simulink model "DYN_02x"  (R2021a)
(part 48 of 53)

 (de2*(0.5*(sin(e6)*(sin(e2 + e3)*sin(e5) - 1.0*cos(e2 + e3)*cos(e4)*cos(e5)) - 1.0*cos(e2 + e3)*cos(e6)*sin(e4))*(I6xy*(cos(e4)*cos(e6) - 1.0*cos(e5)*sin(e4)*sin(e6)) - 1.0*I6yy*(cos(e4)*sin(e6) + cos(e5)*cos(e6)*sin(e4))) + 0.5*(cos(e4)*sin(e6) + cos(e5)*cos(e6)*sin(e4))*(I6zy*(sin(e2 + e3)*cos(e5) + cos(e2 + e3)*cos(e4)*sin(e5)) + I6xy*(cos(e6)*(sin(e2 + e3)*sin(e5) - 1.0*cos(e2 + e3)*cos(e4)*cos(e5)) + cos(e2 + e3)*sin(e4)*sin(e6)) - 1.0*I6yy*(sin(e6)*(sin(e2 + e3)*sin(e5) - 1.0*cos(e2 + e3)*cos(e4)*cos(e5)) - 1.0*cos(e2 + e3)*cos(e6)*sin(e4))) + 0.5*(cos(e6)*(sin(e2 + e3)*sin(e5) - 1.0*cos(e2 + e3)*cos(e4)*cos(e5)) + cos(e2 + e3)*sin(e4)*sin(e6))*(I6yy*(cos(e4)*cos(e6) - 1.0*cos(e5)*sin(e4)*sin(e6)) + I6xy*(cos(e4)*sin(e6) + cos(e5)*cos(e6)*sin(e4)) - 1.0*I6zy*sin(e4)*sin(e5)) - 0.5*(cos(e4)*cos(e6) - 1.0*cos(e5)*sin(e4)*sin(e6))*(I6zx*(sin(e2 + e3)*cos(e5) + cos(e2 + e3)*cos(e4)*sin(e5)) + I6xx*(cos(e6)*(sin(e2 + e3)*sin(e5) - 1.0*cos(e2 + e3)*cos(e4)*cos(e5)) + cos(e2 + e3)*sin(e4)*sin(e6)) - 1.0*I6yx*(sin(e6)*(sin(e2 + e3)*sin(e5) - 1.0*cos(e2 + e3)*cos(e4)*cos(e5)) - 1.0*cos(e2 + e3)*cos(e6)*sin(e4))) + 0.5*(sin(e6)*(sin(e2 + e3)*sin(e5) - 1.0*cos(e2 + e3)*cos(e4)*cos(e5)) - 1.0*cos(e2 + e3)*cos(e6)*sin(e4))*(I6yx*(cos(e4)*cos(e6) - 1.0*cos(e5)*sin(e4)*sin(e6)) + I6xx*(cos(e4)*sin(e6) + cos(e5)*cos(e6)*sin(e4)) - 1.0*I6zx*sin(e4)*sin(e5)) - 0.5*(I6xz*(cos(e4)*cos(e6) - 1.0*cos(e5)*sin(e4)*sin(e6)) - 1.0*I6yz*(cos(e4)*sin(e6) + cos(e5)*cos(e6)*sin(e4)))*(sin(e2 + e3)*cos(e5) + cos(e2 + e3)*cos(e4)*sin(e5)) + 0.5*(I6yx*(cos(e6)*(sin(e2 + e3)*sin(e5) - 1.0*cos(e2 + e3)*cos(e4)*cos(e5)) + cos(e2 + e3)*sin(e4)*sin(e6)) + I6xx*(sin(e6)*(sin(e2 + e3)*sin(e5) - 1.0*cos(e2 + e3)*cos(e4)*cos(e5)) - 1.0*cos(e2 + e3)*cos(e6)*sin(e4)))*(cos(e4)*sin(e6) + cos(e5)*cos(e6)*sin(e4)) + 0.5*(I6yy*(cos(e6)*(sin(e2 + e3)*sin(e5) - 1.0*cos(e2 + e3)*cos(e4)*cos(e5)) + cos(e2 + e3)*sin(e4)*sin(e6)) + I6xy*(sin(e6)*(sin(e2 + e3)*sin(e5) - 1.0*cos(e2 + e3)*cos(e4)*cos(e5)) - 1.0*cos(e2 + e3)*cos(e6)*sin(e4)))*(cos(e4)*cos(e6) - 1.0*cos(e5)*sin(e4)*sin(e6)) - 0.5*(cos(e6)*(sin(e2 + e3)*sin(e5) - 1.0*cos(e2 + e3)*cos(e4)*cos(e5)) + cos(e2 + e3)*sin(e4)*sin(e6))*(I6xx*(cos(e4)*cos(e6) - 1.0*cos(e5)*sin(e4)*sin(e6)) - 1.0*I6yx*(cos(e4)*sin(e6) + cos(e5)*cos(e6)*sin(e4))) - 0.5*sin(e4)*sin(e5)*(I6yz*(cos(e6)*(sin(e2 + e3)*sin(e5) - 1.0*cos(e2 + e3)*cos(e4)*cos(e5)) + cos(e2 + e3)*sin(e4)*sin(e6)) + I6xz*(sin(e6)*(sin(e2 + e3)*sin(e5) - 1.0*cos(e2 + e3)*cos(e4)*cos(e5)) - 1.0*cos(e2 + e3)*cos(e6)*sin(e4))) + m6*((cos(e6)*(sin(e5)*(cos(e2)*sin(e3) + cos(e3)*sin(e2)) + cos(e4)*cos(e5)*(sin(e2)*sin(e3) - 1.0*cos(e2)*cos(e3))) - 1.0*sin(e4)*sin(e6)*(sin(e2)*sin(e3) - 1.0*cos(e2)*cos(e3)))*(z6*(cos(e4)*cos(e6) - 1.0*cos(e5)*sin(e4)*sin(e6)) - 1.0*cos(e6)*(sin(e5)*(a3 + a2*cos(e3)) - 1.0*cos(e4)*cos(e5)*(d4 - 1.0*a2*sin(e3))) + y6*sin(e4)*sin(e5) - 1.0*sin(e4)*sin(e6)*(d4 - 1.0*a2*sin(e3))) - 1.0*(cos(e5)*(cos(e2)*sin(e3) + cos(e3)*sin(e2)) - 1.0*cos(e4)*sin(e5)*(sin(e2)*sin(e3) - 1.0*cos(e2)*cos(e3)))*(x6*(cos(e4)*cos(e6) - 1.0*cos(e5)*sin(e4)*sin(e6)) - 1.0*y6*(cos(e4)*sin(e6) + cos(e5)*cos(e6)*sin(e4)) + cos(e5)*(a3 + a2*cos(e3)) + cos(e4)*sin(e5)*(d4 - 1.0*a2*sin(e3))) + (sin(e6)*(sin(e5)*(cos(e2)*sin(e3) + cos(e3)*sin(e2)) + cos(e4)*cos(e5)*(sin(e2)*sin(e3) - 1.0*cos(e2)*cos(e3))) + cos(e6)*sin(e4)*(sin(e2)*sin(e3) - 1.0*cos(e2)*cos(e3)))*(z6*(cos(e4)*sin(e6) + cos(e5)*cos(e6)*sin(e4)) - 1.0*sin(e6)*(sin(e5)*(a3 + a2*cos(e3)) - 1.0*cos(e4)*cos(e5)*(d4 - 1.0*a2*sin(e3))) + x6*sin(e4)*sin(e5) + cos(e6)*sin(e4)*(d4 - 1.0*a2*sin(e3))))*(1.0*(cos(e6)*(sin(e5)*(cos(e2)*sin(e3) + cos(e3)*sin(e2)) + cos(e4)*cos(e5)*(sin(e2)*sin(e3) - 1.0*cos(e2)*cos(e3))) - 1.0*sin(e4)*sin(e6)*(sin(e2)*sin(e3) - 1.0*cos(e2)*cos(e3)))*(x6*(sin(e2 + e3)*cos(e5) + cos(e2 + e3)*cos(e4)*sin(e5)) - 1.0*z6*(cos(e6)*(sin(e2 + e3)*sin(e5) - 1.0*cos(e2 + e3)*cos(e4)*cos(e5)) + cos(e2 + e3)*sin(e4)*sin(e6)) + cos(e4)*cos(e6)*(a1 + d4*cos(e2 + e3) + a3*sin(e2 + e3) + a2*sin(e2)) - 1.0*cos(e5)*sin(e4)*sin(e6)*(a1 + d4*cos(e2 + e3) + a3*sin(e2 + e3) + a2*sin(e2))) - (sin(e6)*(sin(e5)*(cos(e2)*sin(e3) + cos(e3)*sin(e2)) + cos(e4)*cos(e5)*(sin(e2)*sin(e3) - 1.0*cos(e2)*cos(e3))) + cos(e6)*sin(e4)*(sin(e2)*sin(e3) - 1.0*cos(e2)*cos(e3)))*(z6*(sin(e6)*(sin(e2 + e3)*sin(e5) - 1.0*cos(e2 + e3)*cos(e4)*cos(e5)) - 1.0*cos(e2 + e3)*cos(e6)*sin(e4)) + y6*(sin(e2 + e3)*cos(e5) + cos(e2 + e3)*cos(e4)*sin(e5)) - 1.0*cos(e4)*sin(e6)*(a1 + d4*cos(e2 + e3) + a3*sin(e2 + e3) + a2*sin(e2)) - 1.0*cos(e5)*cos(e6)*sin(e4)*(a1 + d4*cos(e2 + e3) + a3*sin(e2 + e3) + a2*sin(e2))) - (sin(e6)*(sin(e5)*(cos(e2)*sin(e3) + cos(e3)*sin(e2)) + cos(e4)*cos(e5)*(sin(e2)*sin(e3) - 1.0*cos(e2)*cos(e3))) + cos(e6)*sin(e4)*(sin(e2)*sin(e3) - 1.0*cos(e2)*cos(e3)))*(cos(e4)*sin(e6)*(a1 + d4*cos(e2 + e3) + a3*sin(e2 + e3) + a2*sin(e2)) - 1.0*z6*(sin(e6)*(sin(e2 + e3)*sin(e5) - 1.0*cos(e2 + e3)*cos(e4)*cos(e5)) - 1.0*cos(e2 + e3)*cos(e6)*sin(e4)) + cos(e5)*cos(e6)*sin(e4)*(a1 + d4*cos(e2 + e3) + a3*sin(e2 + e3) + a2*sin(e2))) + 1.0*(cos(e6)*(sin(e5)*(cos(e2)*sin(e3) + cos(e3)*sin(e2)) + cos(e4)*cos(e5)*(sin(e2)*sin(e3) - 1.0*cos(e2)*cos(e3))) - 1.0*sin(e4)*sin(e6)*(sin(e2)*sin(e3) - 1.0*cos(e2)*cos(e3)))*(z6*(cos(e6)*(sin(e2 + e3)*sin(e5) - 1.0*cos(e2 + e3)*cos(e4)*cos(e5)) + cos(e2 + e3)*sin(e4)*sin(e6)) - 1.0*cos(e4)*cos(e6)*(a1 + d4*cos(e2 + e3) + a3*sin(e2 + e3) + a2*sin(e2)) + cos(e5)*sin(e4)*sin(e6)*(a1 + d4*cos(e2 + e3) + a3*sin(e2 + e3) + a2*sin(e2))) + (1.0*y6*(sin(e6)*(sin(e2 + e3)*sin(e5) - 1.0*cos(e2 + e3)*cos(e4)*cos(e5)) - 1.0*cos(e2 + e3)*cos(e6)*sin(e4)) - x6*(cos(e6)*(sin(e2 + e3)*sin(e5) - 1.0*cos(e2 + e3)*cos(e4)*cos(e5)) + cos(e2 + e3)*sin(e4)*sin(e6)))*(cos(e5)*(cos(e2)*sin(e3) + cos(e3)*sin(e2)) - 1.0*cos(e4)*sin(e5)*(sin(e2)*sin(e3) - 1.0*cos(e2)*cos(e3)))) - m6*((sin(e6)*(1.0*cos(e5)*(cos(e1)*sin(e4) - 1.0*cos(e4)*(cos(e2)*sin(e1)*sin(e3) + cos(e3)*sin(e1)*sin(e2))) - sin(e5)*(cos(e2)*cos(e3)*sin(e1) - 1.0*sin(e1)*sin(e2)*sin(e3))) - cos(e6)*(sin(e4)*(cos(e2)*sin(e1)*sin(e3) + cos(e3)*sin(e1)*sin(e2)) + cos(e1)*cos(e4)))*(x6*(sin(e2 + e3)*cos(e5) + cos(e2 + e3)*cos(e4)*sin(e5)) - 1.0*z6*(cos(e6)*(sin(e2 + e3)*sin(e5) - 1.0*cos(e2 + e3)*cos(e4)*cos(e5)) + cos(e2 + e3)*sin(e4)*sin(e6)) + cos(e4)*cos(e6)*(a1 + d4*cos(e2 + e3) + a3*sin(e2 + e3) + a2*sin(e2)) - 1.0*cos(e5)*sin(e4)*sin(e6)*(a1 + d4*cos(e2 + e3) + a3*sin(e2 + e3) + a2*sin(e2))) + 1.0*(sin(e5)*(cos(e1)*sin(e4) - 1.0*cos(e4)*(cos(e2)*sin(e1)*sin(e3) + cos(e3)*sin(e1)*sin(e2))) + cos(e5)*(cos(e2)*cos(e3)*sin(e1) - 1.0*sin(e1)*sin(e2)*sin(e3)))*(x6*(sin(e6)*(sin(e2 + e3)*sin(e5) - 1.0*cos(e2 + e3)*cos(e4)*cos(e5)) - 1.0*cos(e2 + e3)*cos(e6)*sin(e4)) + y6*(cos(e6)*(sin(e2 + e3)*sin(e5) - 1.0*cos(e2 + e3)*cos(e4)*cos(e5)) + cos(e2 + e3)*sin(e4)*sin(e6)) - 1.0*sin(e4)*sin(e5)*(a1 + d4*cos(e2 + e3) + a3*sin(e2 + e3) + a2*sin(e2))) + (cos(e6)*(1.0*cos(e5)*(cos(e1)*sin(e4) - 1.0*cos(e4)*(cos(e2)*sin(e1)*sin(e3) + cos(e3)*sin(e1)*sin(e2))) - sin(e5)*(cos(e2)*cos(e3)*sin(e1) - 1.0*sin(e1)*sin(e2)*sin(e3))) + 1.0*sin(e6)*(sin(e4)*(cos(e2)*sin(e1)*sin(e3) + cos(e3)*sin(e1)*sin(e2)) + cos(e1)*cos(e4)))*(z6*(sin(e6)*(sin(e2 + e3)*sin(e5) - 1.0*cos(e2 + e3)*cos(e4)*cos(e5)) - 1.0*cos(e2 + e3)*cos(e6)*sin(e4)) + y6*(sin(e2 + e3)*cos(e5) + cos(e2 + e3)*cos(e4)*sin(e5)) - 1.0*cos(e4)*sin(e6)*(a1 + d4*cos(e2 + e3) + a3*sin(e2 + e3) + a2*sin(e2)) - 1.0*cos(e5)*cos(e6)*sin(e4)*(a1 + d4*cos(e2 + e3) + a3*sin(e2 + e3) + a2*sin(e2))))*((sin(e6)*(1.0*cos(e5)*(cos(e1)*sin(e4) - 1.0*cos(e4)*(cos(e2)*sin(e1)*sin(e3) + cos(e3)*sin(e1)*sin(e2))) - sin(e5)*(cos(e2)*cos(e3)*sin(e1) - 1.0*sin(e1)*sin(e2)*sin(e3))) - cos(e6)*(sin(e4)*(cos(e2)*sin(e1)*sin(e3) + cos(e3)*sin(e1)*sin(e2)) + cos(e1)*cos(e4)))*(z6*(cos(e4)*cos(e6) - 1.0*cos(e5)*sin(e4)*sin(e6)) - 1.0*cos(e6)*(sin(e5)*(a3 + a2*cos(e3)) - 1.0*cos(e4)*cos(e5)*(d4 - 1.0*a2*sin(e3))) + y6*sin(e4)*sin(e5) - 1.0*sin(e4)*sin(e6)*(d4 - 1.0*a2*sin(e3))) + (cos(e6)*(1.0*cos(e5)*(cos(e1)*sin(e4) - 1.0*cos(e4)*(cos(e2)*sin(e1)*sin(e3) + cos(e3)*sin(e1)*sin(e2))) - sin(e5)*(cos(e2)*cos(e3)*sin(e1) - 1.0*sin(e1)*sin(e2)*sin(e3))) + 1.0*sin(e6)*(sin(e4)*(cos(e2)*sin(e1)*sin(e3) + cos(e3)*sin(e1)*sin(e2)) + cos(e1)*cos(e4)))*(z6*(cos(e4)*sin(e6) + cos(e5)*cos(e6)*sin(e4)) - 1.0*sin(e6)*(sin(e5)*(a3 + a2*cos(e3)) - 1.0*cos(e4)*cos(e5)*(d4 - 1.0*a2*sin(e3))) + cos(e6)*sin(e4)*(d4 - 1.0*a2*sin(e3))) + (sin(e6)*(1.0*cos(e5)*(cos(e1)*sin(e4) - 1.0*cos(e4)*(cos(e2)*sin(e1)*sin(e3) + cos(e3)*sin(e1)*sin(e2))) - sin(e5)*(cos(e2)*cos(e3)*sin(e1) - 1.0*sin(e1)*sin(e2)*sin(e3))) - cos(e6)*(sin(e4)*(cos(e2)*sin(e1)*sin(e3) + cos(e3)*sin(e1)*sin(e2)) + cos(e1)*cos(e4)))*(cos(e6)*(sin(e5)*(a3 + a2*cos(e3)) - 1.0*cos(e4)*cos(e5)*(d4 - 1.0*a2*sin(e3))) - 1.0*z6*(cos(e4)*cos(e6) - 1.0*cos(e5)*sin(e4)*sin(e6)) + sin(e4)*sin(e6)*(d4 - 1.0*a2*sin(e3))) - 1.0*(cos(e6)*(1.0*cos(e5)*(cos(e1)*sin(e4) - 1.0*cos(e4)*(cos(e2)*sin(e1)*sin(e3) + cos(e3)*sin(e1)*sin(e2))) - sin(e5)*(cos(e2)*cos(e3)*sin(e1) - 1.0*sin(e1)*sin(e2)*sin(e3))) + 1.0*sin(e6)*(sin(e4)*(cos(e2)*sin(e1)*sin(e3) + cos(e3)*sin(e1)*sin(e2)) + cos(e1)*cos(e4)))*(z6*(cos(e4)*sin(e6) + cos(e5)*cos(e6)*sin(e4)) - 1.0*sin(e6)*(sin(e5)*(a3 + a2*cos(e3)) - 1.0*cos(e4)*cos(e5)*(d4 - 1.0*a2*sin(e3))) + x6*sin(e4)*sin(e5) + cos(e6)*sin(e4)*(d4 - 1.0*a2*sin(e3))) + 1.0*(y6*(cos(e4)*cos(e6) - 1.0*cos(e5)*sin(e4)*sin(e6)) + x6*(cos(e4)*sin(e6) + cos(e5)*cos(e6)*sin(e4)))*(sin(e5)*(cos(e1)*sin(e4) - 1.0*cos(e4)*(cos(e2)*sin(e1)*sin(e3) + cos(e3)*sin(e1)*sin(e2))) + cos(e5)*(cos(e2)*cos(e3)*sin(e1) - 1.0*sin(e1)*sin(e2)*sin(e3)))) - m6*((sin(e6)*(sin(e5)*(cos(e2)*sin(e3) + cos(e3)*sin(e2)) + cos(e4)*cos(e5)*(sin(e2)*sin(e3) - 1.0*cos(e2)*cos(e3))) + cos(e6)*sin(e4)*(sin(e2)*sin(e3) - 1.0*cos(e2)*cos(e3)))*(x6*(sin(e2 + e3)*cos(e5) + cos(e2 + e3)*cos(e4)*sin(e5)) - 1.0*z6*(cos(e6)*(sin(e2 + e3)*sin(e5) - 1.0*cos(e2 + e3)*cos(e4)*cos(e5)) + cos(e2 + e3)*sin(e4)*sin(e6)) + cos(e4)*cos(e6)*(a1 + d4*cos(e2 + e3) + a3*sin(e2 + e3) + a2*sin(e2)) - 1.0*cos(e5)*sin(e4)*sin(e6)*(a1 + d4*cos(e2 + e3) + a3*sin(e2 + e3) + a2*sin(e2))) + (cos(e6)*(sin(e5)*(cos(e2)*sin(e3) + cos(e3)*sin(e2)) + cos(e4)*cos(e5)*(sin(e2)*sin(e3) - 1.0*cos(e2)*cos(e3))) - 1.0*sin(e4)*sin(e6)*(sin(e2)*sin(e3) - 1.0*cos(e2)*cos(e3)))*(z6*(sin(e6)*(sin(e2 + e3)*sin(e5) - 1.0*cos(e2 + e3)*cos(e4)*cos(e5)) - 1.0*cos(e2 + e3)*cos(e6)*sin(e4)) + y6*(sin(e2 + e3)*cos(e5) + cos(e2 + e3)*cos(e4)*sin(e5)) - 1.0*cos(e4)*sin(e6)*(a1 + d4*cos(e2 + e3) + a3*sin(e2 + e3) + a2*sin(e2)) - 1.0*cos(e5)*cos(e6)*sin(e4)*(a1 + d4*cos(e2 + e3) + a3*sin(e2 + e3) + a2*sin(e2))) - 1.0*(cos(e5)*(cos(e2)*sin(e3) + cos(e3)*sin(e2)) - 1.0*cos(e4)*sin(e5)*(sin(e2)*sin(e3) - 1.0*cos(e2)*cos(e3)))*(x6*(sin(e6)*(sin(e2 + e3)*sin(e5) - 1.0*cos(e2 + e3)*cos(e4)*cos(e5)) - 1.0*cos(e2 + e3)*cos(e6)*sin(e4)) + y6*(cos(e6)*(sin(e2 + e3)*sin(e5) - 1.0*cos(e2 + e3)*cos(e4)*cos(e5)) + cos(e2 + e3)*sin(e4)*sin(e6)) - 1.0*sin(e4)*sin(e5)*(a1 + d4*cos(e2 + e3) + a3*sin(e2 + e3) + a2*sin(e2))))*((sin(e6)*(sin(e5)*(cos(e2)*sin(e3) + cos(e3)*sin(e2)) + cos(e4)*cos(e5)*(sin(e2)*sin(e3) - 1.0*cos(e2)*cos(e3))) + cos(e6)*sin(e4)*(sin(e2)*sin(e3) - 1.0*cos(e2)*cos(e3)))*(z6*(cos(e4)*cos(e6) - 1.0*cos(e5)*sin(e4)*sin(e6)) - 1.0*cos(e6)*(sin(e5)*(a3 + a2*cos(e3)) - 1.0*cos(e4)*cos(e5)*(d4 - 1.0*a2*sin(e3))) + y6*sin(e4)*sin(e5) - 1.0*sin(e4)*sin(e6)*(d4 - 1.0*a2*sin(e3))) - 1.0*(cos(e6)*(sin(e5)*(cos(e2)*sin(e3) + cos(e3)*sin(e2)) + cos(e4)*cos(e5)*(sin(e2)*sin(e3) - 1.0*cos(e2)*cos(e3))) - 1.0*sin(e4)*sin(e6)*(sin(e2)*sin(e3) - 1.0*cos(e2)*cos(e3)))*(z6*(cos(e4)*sin(e6) + cos(e5)*cos(e6)*sin(e4)) - 1.0*sin(e6)*(sin(e5)*(a3 + a2*cos(e3)) - 1.0*cos(e4)*cos(e5)*(d4 - 1.0*a2*sin(e3))) + x6*sin(e4)*sin(e5) + cos(e6)*sin(e4)*(d4 - 1.0*a2*sin(e3))) + (sin(e6)*(sin(e5)*(cos(e2)*sin(e3) + cos(e3)*sin(e2)) + cos(e4)*cos(e5)*(sin(e2)*sin(e3) - 1.0*cos(e2)*cos(e3))) + cos(e6)*sin(e4)*(sin(e2)*sin(e3) - 1.0*cos(e2)*cos(e3)))*(cos(e6)*(sin(e5)*(a3 + a2*cos(e3)) - 1.0*cos(e4)*cos(e5)*(d4 - 1.0*a2*sin(e3))) - 1.0*z6*(cos(e4)*cos(e6) - 1.0*cos(e5)*sin(e4)*sin(e6)) + sin(e4)*sin(e6)*(d4 - 1.0*a2*sin(e3))) + (cos(e6)*(sin(e5)*(cos(e2)*sin(e3) + cos(e3)*sin(e2)) + cos(e4)*cos(e5)*(sin(e2)*sin(e3) - 1.0*cos(e2)*cos(e3))) - 1.0*sin(e4)*sin(e6)*(sin(e2)*sin(e3) - 1.0*cos(e2)*cos(e3)))*(z6*(cos(e4)*sin(e6) + cos(e5)*cos(e6)*sin(e4)) - 1.0*sin(e6)*(sin(e5)*(a3 + a2*cos(e3)) - 1.0*cos(e4)*cos(e5)*(d4 - 1.0*a2*sin(e3))) + cos(e6)*sin(e4)*(d4 - 1.0*a2*sin(e3))) - 1.0*(y6*(cos(e4)*cos(e6) - 1.0*cos(e5)*sin(e4)*sin(e6)) + x6*(cos(e4)*sin(e6) + cos(e5)*cos(e6)*sin(e4)))*(cos(e5)*(cos(e2)*sin(e3) + cos(e3)*sin(e2)) - 1.0*cos(e4)*sin(e5)*(sin(e2)*sin(e3) - 1.0*cos(e2)*cos(e3)))) + m6*((sin(e6)*(sin(e5)*(cos(e1)*cos(e2)*cos(e3) - 1.0*cos(e1)*sin(e2)*sin(e3)) + cos(e5)*(sin(e1)*sin(e4) + cos(e4)*(cos(e1)*cos(e2)*sin(e3) + cos(e1)*cos(e3)*sin(e2)))) - 1.0*cos(e6)*(cos(e4)*sin(e1) - 1.0*sin(e4)*(cos(e1)*cos(e2)*sin(e3) + cos(e1)*cos(e3)*sin(e2))))*(z6*(cos(e4)*sin(e6) + cos(e5)*cos(e6)*sin(e4)) - 1.0*sin(e6)*(sin(e5)*(a3 + a2*cos(e3)) - 1.0*cos(e4)*cos(e5)*(d4 - 1.0*a2*sin(e3))) + x6*sin(e4)*sin(e5) + cos(e6)*sin(e4)*(d4 - 1.0*a2*sin(e3))) - 1.0*(cos(e5)*(cos(e1)*cos(e2)*cos(e3) - 1.0*cos(e1)*sin(e2)*sin(e3)) - 1.0*sin(e5)*(sin(e1)*sin(e4) + cos(e4)*(cos(e1)*cos(e2)*sin(e3) + cos(e1)*cos(e3)*sin(e2))))*(x6*(cos(e4)*cos(e6) - 1.0*cos(e5)*sin(e4)*sin(e6)) - 1.0*y6*(cos(e4)*sin(e6) + cos(e5)*cos(e6)*sin(e4)) + cos(e5)*(a3 + a2*cos(e3)) + cos(e4)*sin(e5)*(d4 - 1.0*a2*sin(e3))) + (sin(e6)*(cos(e4)*sin(e1) - 1.0*sin(e4)*(cos(e1)*cos(e2)*sin(e3) + cos(e1)*cos(e3)*sin(e2))) + cos(e6)*(sin(e5)*(cos(e1)*cos(e2)*cos(e3) - 1.0*cos(e1)*sin(e2)*sin(e3)) + cos(e5)*(sin(e1)*sin(e4) + cos(e4)*(cos(e1)*cos(e2)*sin(e3) + cos(e1)*cos(e3)*sin(e2)))))*(z6*(cos(e4)*cos(e6) - 1.0*cos(e5)*sin(e4)*sin(e6)) - 1.0*cos(e6)*(sin(e5)*(a3 + a2*cos(e3)) - 1.0*cos(e4)*cos(e5)*(d4 - 1.0*a2*sin(e3))) + y6*sin(e4)*sin(e5) - 1.0*sin(e4)*sin(e6)*(d4 - 1.0*a2*sin(e3))))*(1.0*(sin(e6)*(cos(e4)*sin(e1) - 1.0*sin(e4)*(cos(e1)*cos(e2)*sin(e3) + cos(e1)*cos(e3)*sin(e2))) + cos(e6)*(sin(e5)*(cos(e1)*cos(e2)*cos(e3) - 1.0*cos(e1)*sin(e2)*sin(e3)) + cos(e5)*(sin(e1)*sin(e4) + cos(e4)*(cos(e1)*cos(e2)*sin(e3) + cos(e1)*cos(e3)*sin(e2)))))*(x6*(sin(e2 + e3)*cos(e5) + cos(e2 + e3)*cos(e4)*sin(e5)) - 1.0*z6*(cos(e6)*(sin(e2 + e3)*sin(e5) - 1.0*cos(e2 + e3)*cos(e4)*cos(e5)) + cos(e2 + e3)*sin(e4)*sin(e6)) + cos(e4)*cos(e6)*(a1 + d4*cos(e2 + e3) + a3*sin(e2 + e3) + a2*sin(e2)) - 1.0*cos(e5)*sin(e4)*sin(e6)*(a1 + d4*cos(e2 + e3) + a3*sin(e2 + e3) + a2*sin(e2))) - (sin(e6)*(sin(e5)*(cos(e1)*cos(e2)*cos(e3) - 1.0*cos(e1)*sin(e2)*sin(e3)) + cos(e5)*(sin(e1)*sin(e4) + cos(e4)*(cos(e1)*cos(e2)*sin(e3) + cos(e1)*cos(e3)*sin(e2)))) - 1.0*cos(e6)*(cos(e4)*sin(e1) - 1.0*sin(e4)*(cos(e1)*cos(e2)*sin(e3) + cos(e1)*cos(e3)*sin(e2))))*(cos(e4)*sin(e6)*(a1 + d4*cos(e2 + e3) + a3*sin(e2 + e3) + a2*sin(e2)) - 1.0*z6*(sin(e6)*(sin(e2 + e3)*sin(e5) - 1.0*cos(e2 + e3)*cos(e4)*cos(e5)) - 1.0*cos(e2 + e3)*cos(e6)*sin(e4)) + cos(e5)*cos(e6)*sin(e4)*(a1 + d4*cos(e2 + e3) + a3*sin(e2 + e3) + a2*sin(e2))) - (sin(e6)*(sin(e5)*(cos(e1)*cos(e2)*cos(e3) - 1.0*cos(e1)*sin(e2)*sin(e3)) + cos(e5)*(sin(e1)*sin(e4) + cos(e4)*(cos(e1)*cos(e2)*sin(e3) + cos(e1)*cos(e3)*sin(e2)))) - 1.0*cos(e6)*(cos(e4)*sin(e1) - 1.0*sin(e4)*(cos(e1)*cos(e2)*sin(e3) + cos(e1)*cos(e3)*sin(e2))))*(z6*(sin(e6)*(sin(e2 + e3)*sin(e5) - 1.0*cos(e2 + e3)*cos(e4)*cos(e5)) - 1.0*cos(e2 + e3)*cos(e6)*sin(e4)) + y6*(sin(e2 + e3)*cos(e5) + cos(e2 + e3)*cos(e4)*sin(e5)) - 1.0*cos(e4)*sin(e6)*(a1 + d4*cos(e2 + e3) + a3*sin(e2 + e3) + a2*sin(e2)) - 1.0*cos(e5)*cos(e6)*sin(e4)*(a1 + d4*cos(e2 + e3) + a3*sin(e2 + e3) + a2*sin(e2))) + 1.0*(sin(e6)*(cos(e4)*sin(e1) - 1.0*sin(e4)*(cos(e1)*cos(e2)*sin(e3) + cos(e1)*cos(e3)*sin(e2))) + cos(e6)*(sin(e5)*(cos(e1)*cos(e2)*cos(e3) - 1.0*cos(e1)*sin(e2)*sin(e3)) + cos(e5)*(sin(e1)*sin(e4) + cos(e4)*(cos(e1)*cos(e2)*sin(e3) + cos(e1)*cos(e3)*sin(e2)))))*(z6*(cos(e6)*(sin(e2 + e3)*sin(e5) - 1.0*cos(e2 + e3)*cos(e4)*cos(e5)) + cos(e2 + e3)*sin(e4)*sin(e6)) - 1.0*cos(e4)*cos(e6)*(a1 + d4*cos(e2 + e3) + a3*sin(e2 + e3) + a2*sin(e2)) + cos(e5)*sin(e4)*sin(e6)*(a1 + d4*cos(e2 + e3) + a3*sin(e2 + e3) + a2*sin(e2))) + (cos(e5)*(cos(e1)*cos(e2)*cos(e3) - 1.0*cos(e1)*sin(e2)*sin(e3)) - 1.0*sin(e5)*(sin(e1)*sin(e4) + cos(e4)*(cos(e1)*cos(e2)*sin(e3) + cos(e1)*cos(e3)*sin(e2))))*(1.0*y6*(sin(e6)*(sin(e2 + e3)*sin(e5) - 1.0*cos(e2 + e3)*cos(e4)*cos(e5)) - 1.0*cos(e2 + e3)*cos(e6)*sin(e4)) - x6*(cos(e6)*(sin(e2 + e3)*sin(e5) - 1.0*cos(e2 + e3)*cos(e4)*cos(e5)) + cos(e2 + e3)*sin(e4)*sin(e6)))) - m6*((sin(e6)*(sin(e5)*(cos(e1)*cos(e2)*cos(e3) - 1.0*cos(e1)*sin(e2)*sin(e3)) + cos(e5)*(sin(e1)*sin(e4) + cos(e4)*(cos(e1)*cos(e2)*sin(e3) + cos(e1)*cos(e3)*sin(e2)))) - 1.0*cos(e6)*(cos(e4)*sin(e1) - 1.0*sin(e4)*(cos(e1)*cos(e2)*sin(e3) + cos(e1)*cos(e3)*sin(e2))))*(x6*(sin(e2 + e3)*cos(e5) + cos(e2 + e3)*cos(e4)*sin(e5)) - 1.0*z6*(cos(e6)*(sin(e2 + e3)*sin(e5) - 1.0*cos(e2 + e3)*cos(e4)*cos(e5)) + cos(e2 + e3)*sin(e4)*sin(e6)) + cos(e4)*cos(e6)*(a1 + d4*cos(e2 + e3) + a3*sin(e2 + e3) + a2*sin(e2)) - 1.0*cos(e5)*sin(e4)*sin(e6)*(a1 + d4*cos(e2 + e3) + a3*sin(e2 + e3) + a2*sin(e2))) + (sin(e6)*(cos(e4)*sin(e1) - 1.0*sin(e4)*(cos(e1)*cos(e2)*sin(e3) + cos(e1)*cos(e3)*sin(e2))) + cos(e6)*(sin(e5)*(cos(e1)*cos(e2)*cos(e3) - 1.0*cos(e1)*sin(e2)*sin(e3)) + cos(e5)*(sin(e1)*sin(e4) + cos(e4)*(cos(e1)*cos(e2)*sin(e3) + cos(e1)*cos(e3)*sin(e2)))))*(z6*(sin(e6)*(sin(e2 + e3)*sin(e5) - 1.0*cos(e2 + e3)*cos(e4)*cos(e5)) - 1.0*cos(e2 + e3)*cos(e6)*sin(e4)) + y6*(sin(e2 + e3)*cos(e5) + cos(e2 + e3)*cos(e4)*sin(e5)) - 1.0*cos(e4)*sin(e6)*(a1 + d4*cos(e2 + e3) + a3*sin(e2 + e3) + a2*sin(e2)) - 1.0*cos(e5)*cos(e6)*sin(e4)*(a1 + d4*cos(e2 + e3) + a3*sin(e2 + e3) + a2*sin(e2))) - 1.0*(cos(e5)*(cos(e1)*cos(e2)*cos(e3) - 1.0*cos(e1)*sin(e2)*sin(e3)) - 1.0*sin(e5)*(sin(e1)*sin(e4) + cos(e4)*(cos(e1)*cos(e2)*sin(e3) + cos(e1)*cos(e3)*sin(e2))))*(x6*(sin(e6)*(sin(e2 + e3)*sin(e5) - 1.0*cos(e2 + e3)*cos(e4)*cos(e5)) - 1.0*cos(e2 + e3)*cos(e6)*sin(e4)) + y6*(cos(e6)*(sin(e2 + e3)*sin(e5) - 1.0*cos(e2 + e3)*cos(e4)*cos(e5)) + cos(e2 + e3)*sin(e4)*sin(e6)) - 1.0*sin(e4)*sin(e5)*(a1 + d4*cos(e2 + e3) + a3*sin(e2 + e3) + a2*sin(e2))))*((sin(e6)*(sin(e5)*(cos(e1)*cos(e2)*cos(e3) - 1.0*cos(e1)*sin(e2)*sin(e3)) + cos(e5)*(sin(e1)*sin(e4) + cos(e4)*(cos(e1)*cos(e2)*sin(e3) + cos(e1)*cos(e3)*sin(e2)))) - 1.0*cos(e6)*(cos(e4)*sin(e1) - 1.0*sin(e4)*(cos(e1)*cos(e2)*sin(e3) + cos(e1)*cos(e3)*sin(e2))))*(cos(e6)*(sin(e5)*(a3 + a2*cos(e3)) - 1.0*cos(e4)*cos(e5)*(d4 - 1.0*a2*sin(e3))) - 1.0*z6*(cos(e4)*cos(e6) - 1.0*cos(e5)*sin(e4)*sin(e6)) + sin(e4)*sin(e6)*(d4 - 1.0*a2*sin(e3))) - 1.0*(sin(e6)*(cos(e4)*sin(e1) - 1.0*sin(e4)*(cos(e1)*cos(e2)*sin(e3) + cos(e1)*cos(e3)*sin(e2))) + cos(e6)*(sin(e5)*(cos(e1)*cos(e2)*cos(e3) - 1.0*cos(e1)*sin(e2)*sin(e3)) + cos(e5)*(sin(e1)*sin(e4) + cos(e4)*(cos(e1)*cos(e2)*sin(e3) + cos(e1)*cos(e3)*sin(e2)))))*(z6*(cos(e4)*sin(e6) + cos(e5)*cos(e6)*sin(e4)) - 1.0*sin(e6)*(sin(e5)*(a3 + a2*cos(e3)) - 1.0*cos(e4)*cos(e5)*(d4 - 1.0*a2*sin(e3))) + x6*sin(e4)*sin(e5) + cos(e6)*sin(e4)*(d4 - 1.0*a2*sin(e3))) + (sin(e6)*(cos(e4)*sin(e1) - 1.0*sin(e4)*(cos(e1)*cos(e2)*sin(e3) + cos(e1)*cos(e3)*sin(e2))) + cos(e6)*(sin(e5)*(cos(e1)*cos(e2)*cos(e3) - 1.0*cos(e1)*sin(e2)*sin(e3)) + cos(e5)*(sin(e1)*sin(e4) + cos(e4)*(cos(e1)*cos(e2)*sin(e3) + cos(e1)*cos(e3)*sin(e2)))))*(z6*(cos(e4)*sin(e6) + cos(e5)*cos(e6)*sin(e4)) - 1.0*sin(e6)*(sin(e5)*(a3 + a2*cos(e3)) - 1.0*cos(e4)*cos(e5)*(d4 - 1.0*a2*sin(e3))) + cos(e6)*sin(e4)*(d4 - 1.0*a2*sin(e3))) - 1.0*(y6*(cos(e4)*cos(e6) - 1.0*cos(e5)*sin(e4)*sin(e6)) + x6*(cos(e4)*sin(e6) + cos(e5)*cos(e6)*sin(e4)))*(cos(e5)*(cos(e1)*cos(e2)*cos(e3) - 1.0*cos(e1)*sin(e2)*sin(e3)) - 1.0*sin(e5)*(sin(e1)*sin(e4) + cos(e4)*(cos(e1)*cos(e2)*sin(e3) + cos(e1)*cos(e3)*sin(e2)))) + (sin(e6)*(sin(e5)*(cos(e1)*cos(e2)*cos(e3) - 1.0*cos(e1)*sin(e2)*sin(e3)) + cos(e5)*(sin(e1)*sin(e4) + cos(e4)*(cos(e1)*cos(e2)*sin(e3) + cos(e1)*cos(e3)*sin(e2)))) - 1.0*cos(e6)*(cos(e4)*sin(e1) - 1.0*sin(e4)*(cos(e1)*cos(e2)*sin(e3) + cos(e1)*cos(e3)*sin(e2))))*(z6*(cos(e4)*cos(e6) - 1.0*cos(e5)*sin(e4)*sin(e6)) - 1.0*cos(e6)*(sin(e5)*(a3 + a2*cos(e3)) - 1.0*cos(e4)*cos(e5)*(d4 - 1.0*a2*sin(e3))) + y6*sin(e4)*sin(e5) - 1.0*sin(e4)*sin(e6)*(d4 - 1.0*a2*sin(e3)))) - m6*(1.0*(sin(e5)*(cos(e1)*sin(e4) - 1.0*cos(e4)*(cos(e2)*sin(e1)*sin(e3) + cos(e3)*sin(e1)*sin(e2))) + cos(e5)*(cos(e2)*cos(e3)*sin(e1) - 1.0*sin(e1)*sin(e2)*sin(e3)))*(x6*(cos(e4)*cos(e6) - 1.0*cos(e5)*sin(e4)*sin(e6)) - 1.0*y6*(cos(e4)*sin(e6) + cos(e5)*cos(e6)*sin(e4)) + cos(e5)*(a3 + a2*cos(e3)) + cos(e4)*sin(e5)*(d4 - 1.0*a2*sin(e3))) + (cos(e6)*(1.0*cos(e5)*(cos(e1)*sin(e4) - 1.0*cos(e4)*(cos(e2)*sin(e1)*sin(e3) + cos(e3)*sin(e1)*sin(e2))) - sin(e5)*(cos(e2)*cos(e3)*sin(e1) - 1.0*sin(e1)*sin(e2)*sin(e3))) + 1.0*sin(e6)*(sin(e4)*(cos(e2)*sin(e1)*sin(e3) + cos(e3)*sin(e1)*sin(e2)) + cos(e1)*cos(e4)))*(z6*(cos(e4)*cos(e6) - 1.0*cos(e5)*sin(e4)*sin(e6)) - 1.0*cos(e6)*(sin(e5)*(a3 + a2*cos(e3)) - 1.0*cos(e4)*cos(e5)*(d4 - 1.0*a2*sin(e3))) + y6*sin(e4)*sin(e5) - 1.0*sin(e4)*sin(e6)*(d4 - 1.0*a2*sin(e3))) + (sin(e6)*(1.0*cos(e5)*(cos(e1)*sin(e4) - 1.0*cos(e4)*(cos(e2)*sin(e1)*sin(e3) + cos(e3)*sin(e1)*sin(e2))) - sin(e5)*(cos(e2)*cos(e3)*sin(e1) - 1.0*sin(e1)*sin(e2)*sin(e3))) - cos(e6)*(sin(e4)*(cos(e2)*sin(e1)*sin(e3) + cos(e3)*sin(e1)*sin(e2)) + cos(e1)*cos(e4)))*(z6*(cos(e4)*sin(e6) + cos(e5)*cos(e6)*sin(e4)) - 1.0*sin(e6)*(sin(e5)*(a3 + a2*cos(e3)) - 1.0*cos(e4)*cos(e5)*(d4 - 1.0*a2*sin(e3))) + x6*sin(e4)*sin(e5) + cos(e6)*sin(e4)*(d4 - 1.0*a2*sin(e3))))*((1.0*y6*(sin(e6)*(sin(e2 + e3)*sin(e5) - 1.0*cos(e2 + e3)*cos(e4)*cos(e5)) - 1.0*cos(e2 + e3)*cos(e6)*sin(e4)) - x6*(cos(e6)*(sin(e2 + e3)*sin(e5) - 1.0*cos(e2 + e3)*cos(e4)*cos(e5)) + cos(e2 + e3)*sin(e4)*sin(e6)))*(sin(e5)*(cos(e1)*sin(e4) - 1.0*cos(e4)*(cos(e2)*sin(e1)*sin(e3) + cos(e3)*sin(e1)*sin(e2))) + cos(e5)*(cos(e2)*cos(e3)*sin(e1) - 1.0*sin(e1)*sin(e2)*sin(e3))) - 1.0*(cos(e6)*(1.0*cos(e5)*(cos(e1)*sin(e4) - 1.0*cos(e4)*(cos(e2)*sin(e1)*sin(e3) + cos(e3)*sin(e1)*sin(e2))) - sin(e5)*(cos(e2)*cos(e3)*sin(e1) - 1.0*sin(e1)*sin(e2)*sin(e3))) + 1.0*sin(e6)*(sin(e4)*(cos(e2)*sin(e1)*sin(e3) + cos(e3)*sin(e1)*sin(e2)) + cos(e1)*cos(e4)))*(x6*(sin(e2 + e3)*cos(e5) + cos(e2 + e3)*cos(e4)*sin(e5)) - 1.0*z6*(cos(e6)*(sin(e2 + e3)*sin(e5) - 1.0*cos(e2 + e3)*cos(e4)*cos(e5)) + cos(e2 + e3)*sin(e4)*sin(e6)) + cos(e4)*cos(e6)*(a1 + d4*cos(e2 + e3) + a3*sin(e2 + e3) + a2*sin(e2)) - 1.0*cos(e5)*sin(e4)*sin(e6)*(a1 + d4*cos(e2 + e3) + a3*sin(e2 + e3) + a2*sin(e2))) + (sin(e6)*(1.0*cos(e5)*(cos(e1)*sin(e4) - 1.0*cos(e4)*(cos(e2)*sin(e1)*sin(e3) + cos(e3)*sin(e1)*sin(e2))) - sin(e5)*(cos(e2)*cos(e3)*sin(e1) - 1.0*sin(e1)*sin(e2)*sin(e3))) - cos(e6)*(sin(e4)*(cos(e2)*sin(e1)*sin(e3) + cos(e3)*sin(e1)*sin(e2)) + cos(e1)*cos(e4)))*(z6*(sin(e6)*(sin(e2 + e3)*sin(e5) - 1.0*cos(e2 + e3)*cos(e4)*cos(e5)) - 1.0*cos(e2 + e3)*cos(e6)*sin(e4)) + y6*(sin(e2 + e3)*cos(e5) + cos(e2 + e3)*cos(e4)*sin(e5)) - 1.0*cos(e4)*sin(e6)*(a1 + d4*cos(e2 + e3) + a3*sin(e2 + e3) + a2*sin(e2)) - 1.0*cos(e5)*cos(e6)*sin(e4)*(a1 + d4*cos(e2 + e3) + a3*sin(e2 + e3) + a2*sin(e2))) - 1.0*(cos(e6)*(1.0*cos(e5)*(cos(e1)*sin(e4) - 1.0*cos(e4)*(cos(e2)*sin(e1)*sin(e3) + cos(e3)*sin(e1)*sin(e2))) - sin(e5)*(cos(e2)*cos(e3)*sin(e1) - 1.0*sin(e1)*sin(e2)*sin(e3))) + 1.0*sin(e6)*(sin(e4)*(cos(e2)*sin(e1)*sin(e3) + cos(e3)*sin(e1)*sin(e2)) + cos(e1)*cos(e4)))*(z6*(cos(e6)*(sin(e2 + e3)*sin(e5) - 1.0*cos(e2 + e3)*cos(e4)*cos(e5)) + cos(e2 + e3)*sin(e4)*sin(e6)) - 1.0*cos(e4)*cos(e6)*(a1 + d4*cos(e2 + e3) + a3*sin(e2 + e3) + a2*sin(e2)) + cos(e5)*sin(e4)*sin(e6)*(a1 + d4*cos(e2 + e3) + a3*sin(e2 + e3) + a2*sin(e2))) + (sin(e6)*(1.0*cos(e5)*(cos(e1)*sin(e4) - 1.0*cos(e4)*(cos(e2)*sin(e1)*sin(e3) + cos(e3)*sin(e1)*sin(e2))) - sin(e5)*(cos(e2)*cos(e3)*sin(e1) - 1.0*sin(e1)*sin(e2)*sin(e3))) - cos(e6)*(sin(e4)*(cos(e2)*sin(e1)*sin(e3) + cos(e3)*sin(e1)*sin(e2)) + cos(e1)*cos(e4)))*(cos(e4)*sin(e6)*(a1 + d4*cos(e2 + e3) + a3*sin(e2 + e3) + a2*sin(e2)) - 1.0*z6*(sin(e6)*(sin(e2 + e3)*sin(e5) - 1.0*cos(e2 + e3)*cos(e4)*cos(e5)) - 1.0*cos(e2 + e3)*cos(e6)*sin(e4)) + cos(e5)*cos(e6)*sin(e4)*(a1 + d4*cos(e2 + e3) + a3*sin(e2 + e3) + a2*sin(e2))))))/2 - de5*(m6*(x6*(sin(e6)*(sin(e5)*(cos(e1)*cos(e2)*cos(e3) - cos(e1)*sin(e2)*sin(e3)) + cos(e5)*(sin(e1)*sin(e4) + cos(e4)*(cos(e1)*cos(e2)*sin(e3) + cos(e1)*cos(e3)*sin(e2)))) - cos(e6)*(cos(e4)*sin(e1) - sin(e4)*(cos(e1)*cos(e2)*sin(e3) + cos(e1)*cos(e3)*sin(e2)))) + y6*(cos(e6)*(sin(e5)*(cos(e1)*cos(e2)*cos(e3) - cos(e1)*sin(e2)*sin(e3)) + cos(e5)*(sin(e1)*sin(e4) + cos(e4)*(cos(e1)*cos(e2)*sin(e3) + cos(e1)*cos(e3)*sin(e2)))) + sin(e6)*(cos(e4)*sin(e1) - sin(e4)*(cos(e1)*cos(e2)*sin(e3) + cos(e1)*cos(e3)*sin(e2)))))*((cos(e6)*(sin(e5)*(cos(e1)*cos(e2)*cos(e3) - cos(e1)*sin(e2)*sin(e3)) + cos(e5)*(sin(e1)*sin(e4) + cos(e4)*(cos(e1)*cos(e2)*sin(e3) + cos(e1)*cos(e3)*sin(e2)))) + sin(e6)*(cos(e4)*sin(e1) - sin(e4)*(cos(e1)*cos(e2)*sin(e3) + cos(e1)*cos(e3)*sin(e2))))*(z6*sin(e6)*(sin(e2 + e3)*cos(e5) + cos(e2 + e3)*cos(e4)*sin(e5)) - y6*(sin(e2 + e3)*sin(e5) - cos(e2 + e3)*cos(e4)*cos(e5)) + cos(e6)*sin(e4)*sin(e5)*(a1 + d4*cos(e2 + e3) + a3*sin(e2 + e3) + a2*sin(e2))) - (sin(e6)*(sin(e5)*(cos(e1)*cos(e2)*cos(e3) - cos(e1)*sin(e2)*sin(e3)) + cos(e5)*(sin(e1)*sin(e4) + cos(e4)*(cos(e1)*cos(e2)*sin(e3) + cos(e1)*cos(e3)*sin(e2)))) - cos(e6)*(cos(e4)*sin(e1) - sin(e4)*(cos(e1)*cos(e2)*sin(e3) + cos(e1)*cos(e3)*sin(e2))))*(x6*(sin(e2 + e3)*sin(e5) - cos(e2 + e3)*cos(e4)*cos(e5)) + z6*cos(e6)*(sin(e2 + e3)*cos(e5) + cos(e2 + e3)*cos(e4)*sin(e5)) - sin(e4)*sin(e5)*sin(e6)*(a1 + d4*cos(e2 + e3) + a3*sin(e2 + e3) + a2*sin(e2))) + (sin(e5)*(cos(e1)*cos(e2)*cos(e3) - cos(e1)*sin(e2)*sin(e3)) + cos(e5)*(sin(e1)*sin(e4) + cos(e4)*(cos(e1)*cos(e2)*sin(e3) + cos(e1)*cos(e3)*sin(e2))))*(x6*(sin(e6)*(sin(e2 + e3)*sin(e5) - cos(e2 + e3)*cos(e4)*cos(e5)) - cos(e2 + e3)*cos(e6)*sin(e4)) + y6*(cos(e6)*(sin(e2 + e3)*sin(e5) - cos(e2 + e3)*cos(e4)*cos(e5)) + cos(e2 + e3)*sin(e4)*sin(e6)) - sin(e4)*sin(e5)*(a1 + d4*cos(e2 + e3) + a3*sin(e2 + e3) + a2*sin(e2))) - (cos(e5)*(cos(e1)*cos(e2)*cos(e3) - cos(e1)*sin(e2)*sin(e3)) - sin(e5)*(sin(e1)*sin(e4) + cos(e4)*(cos(e1)*cos(e2)*sin(e3) + cos(e1)*cos(e3)*sin(e2))))*(y6*cos(e6)*(sin(e2 + e3)*cos(e5) + cos(e2 + e3)*cos(e4)*sin(e5)) - cos(e5)*sin(e4)*(a1 + d4*cos(e2 + e3) + a3*sin(e2 + e3) + a2*sin(e2)) + x6*sin(e6)*(sin(e2 + e3)*cos(e5) + cos(e2 + e3)*cos(e4)*sin(e5))) + cos(e6)*(cos(e5)*(cos(e1)*cos(e2)*cos(e3) - cos(e1)*sin(e2)*sin(e3)) - sin(e5)*(sin(e1)*sin(e4) + cos(e4)*(cos(e1)*cos(e2)*sin(e3) + cos(e1)*cos(e3)*sin(e2))))*(y6*(sin(e2 + e3)*cos(e5) + cos(e2 + e3)*cos(e4)*sin(e5)) + z6*(sin(e6)*(sin(e2 + e3)*sin(e5) - cos(e2 + e3)*cos(e4)*cos(e5)) - cos(e2 + e3)*cos(e6)*sin(e4)) - cos(e4)*sin(e6)*(a1 + d4*cos(e2 + e3) + a3*sin(e2 + e3) + a2*sin(e2)) - cos(e5)*cos(e6)*sin(e4)*(a1 + d4*cos(e2 + e3) + a3*sin(e2 + e3) + a2*sin(e2))) + sin(e6)*(cos(e5)*(cos(e1)*cos(e2)*cos(e3) - cos(e1)*sin(e2)*sin(e3)) - sin(e5)*(sin(e1)*sin(e4) + cos(e4)*(cos(e1)*cos(e2)*sin(e3) + cos(e1)*cos(e3)*sin(e2))))*(x6*(sin(e2 + e3)*cos(e5) + cos(e2 + e3)*cos(e4)*sin(e5)) - z6*(cos(e6)*(sin(e2 + e3)*sin(e5) - cos(e2 + e3)*cos(e4)*cos(e5)) + cos(e2 + e3)*sin(e4)*sin(e6)) + cos(e4)*cos(e6)*(a1 + d4*cos(e2 + e3) + a3*sin(e2 + e3) + a2*sin(e2)) - cos(e5)*sin(e4)*sin(e6)*(a1 + d4*cos(e2 + e3) + a3*sin(e2 + e3) + a2*sin(e2)))) - I6zz*(sin(e2 + e3)*sin(e5) - cos(e2 + e3)*cos(e4)*cos(e5)) + (I6xz*cos(e6)*(sin(e2 + e3)*cos(e5) + cos(e2 + e3)*cos(e4)*sin(e5)))/2 + (I6zx*cos(e6)*(sin(e2 + e3)*cos(e5) + cos(e2 + e3)*cos(e4)*sin(e5)))/2 - (I6yz*sin(e6)*(sin(e2 + e3)*cos(e5) + cos(e2 + e3)*cos(e4)*sin(e5)))/2 - (I6zy*sin(e6)*(sin(e2 + e3)*cos(e5) + cos(e2 + e3)*cos(e4)*sin(e5)))/2 + m6*(y6*cos(e6)*(cos(e5)*(cos(e1)*cos(e2)*cos(e3) - cos(e1)*sin(e2)*sin(e3)) - sin(e5)*(sin(e1)*sin(e4) + cos(e4)*(cos(e1)*cos(e2)*sin(e3) + cos(e1)*cos(e3)*sin(e2)))) + x6*sin(e6)*(cos(e5)*(cos(e1)*cos(e2)*cos(e3) - cos(e1)*sin(e2)*sin(e3)) - sin(e5)*(sin(e1)*sin(e4) + cos(e4)*(cos(e1)*cos(e2)*sin(e3) + cos(e1)*cos(e3)*sin(e2)))))*((sin(e6)*(sin(e5)*(cos(e1)*cos(e2)*cos(e3) - cos(e1)*sin(e2)*sin(e3)) + cos(e5)*(sin(e1)*sin(e4) + cos(e4)*(cos(e1)*cos(e2)*sin(e3) + cos(e1)*cos(e3)*sin(e2)))) - cos(e6)*(cos(e4)*sin(e1) - sin(e4)*(cos(e1)*cos(e2)*sin(e3) + cos(e1)*cos(e3)*sin(e2))))*(x6*(sin(e2 + e3)*cos(e5) + cos(e2 + e3)*cos(e4)*sin(e5)) - z6*(cos(e6)*(sin(e2 + e3)*sin(e5) - cos(e2 + e3)*cos(e4)*cos(e5)) + cos(e2 + e3)*sin(e4)*sin(e6)) + cos(e4)*cos(e6)*(a1 + d4*cos(e2 + e3) + a3*sin(e2 + e3) + a2*sin(e2)) - cos(e5)*sin(e4)*sin(e6)*(a1 + d4*cos(e2 + e3) + a3*sin(e2 + e3) + a2*sin(e2))) + (cos(e6)*(sin(e5)*(cos(e1)*cos(e2)*cos(e3) - cos(e1)*sin(e2)*sin(e3)) + cos(e5)*(sin(e1)*sin(e4) + cos(e4)*(cos(e1)*cos(e2)*sin(e3) + cos(e1)*cos(e3)*sin(e2)))) + sin(e6)*(cos(e4)*sin(e1) - sin(e4)*(cos(e1)*cos(e2)*sin(e3) + cos(e1)*cos(e3)*sin(e2))))*(y6*(sin(e2 + e3)*cos(e5) + cos(e2 + e3)*cos(e4)*sin(e5)) + z6*(sin(e6)*(sin(e2 + e3)*sin(e5) - cos(e2 + e3)*cos(e4)*cos(e5)) - cos(e2 + e3)*cos(e6)*sin(e4)) - cos(e4)*sin(e6)*(a1 + d4*cos(e2 + e3) + a3*sin(e2 + e3) + a2*sin(e2)) - cos(e5)*cos(e6)*sin(e4)*(a1 + d4*cos(e2 + e3) + a3*sin(e2 + e3) + a2*sin(e2))) - (cos(e5)*(cos(e1)*cos(e2)*cos(e3) - cos(e1)*sin(e2)*sin(e3)) - sin(e5)*(sin(e1)*sin(e4) + cos(e4)*(cos(e1)*cos(e2)*sin(e3) + cos(e1)*cos(e3)*sin(e2))))*(x6*(sin(e6)*(sin(e2 + e3)*sin(e5) - cos(e2 + e3)*cos(e4)*cos(e5)) - cos(e2 + e3)*cos(e6)*sin(e4)) + y6*(cos(e6)*(sin(e2 + e3)*sin(e5) - cos(e2 + e3)*cos(e4)*cos(e5)) + cos(e2 + e3)*sin(e4)*sin(e6)) - sin(e4)*sin(e5)*(a1 + d4*cos(e2 + e3) + a3*sin(e2 + e3) + a2*sin(e2)))) + m6*(x6*(sin(e6)*(sin(e5)*(cos(e2)*sin(e3) + cos(e3)*sin(e2)) + cos(e4)*cos(e5)*(sin(e2)*sin(e3) - cos(e2)*cos(e3))) + cos(e6)*sin(e4)*(sin(e2)*sin(e3) - cos(e2)*cos(e3))) + y6*(cos(e6)*(sin(e5)*(cos(e2)*sin(e3) + cos(e3)*sin(e2)) + cos(e4)*cos(e5)*(sin(e2)*sin(e3) - cos(e2)*cos(e3))) - sin(e4)*sin(e6)*(sin(e2)*sin(e3) - cos(e2)*cos(e3))))*((sin(e5)*(cos(e2)*sin(e3) + cos(e3)*sin(e2)) + cos(e4)*cos(e5)*(sin(e2)*sin(e3) - cos(e2)*cos(e3)))*(x6*(sin(e6)*(sin(e2 + e3)*sin(e5) - cos(e2 + e3)*cos(e4)*cos(e5)) - cos(e2 + e3)*cos(e6)*sin(e4)) + y6*(cos(e6)*(sin(e2 + e3)*sin(e5) - cos(e2 + e3)*cos(e4)*cos(e5)) + cos(e2 + e3)*sin(e4)*sin(e6)) - sin(e4)*sin(e5)*(a1 + d4*cos(e2 + e3) + a3*sin(e2 + e3) + a2*sin(e2))) - (cos(e5)*(cos(e2)*sin(e3) + cos(e3)*sin(e2)) - cos(e4)*sin(e5)*(sin(e2)*sin(e3) - cos(e2)*cos(e3)))*(y6*cos(e6)*(sin(e2 + e3)*cos(e5) + cos(e2 + e3)*cos(e4)*sin(e5)) - cos(e5)*sin(e4)*(a1 + d4*cos(e2 + e3) + a3*sin(e2 + e3) + a2*sin(e2)) + x6*sin(e6)*(sin(e2 + e3)*cos(e5) + cos(e2 + e3)*cos(e4)*sin(e5))) - (sin(e6)*(sin(e5)*(cos(e2)*sin(e3) + cos(e3)*sin(e2)) + cos(e4)*cos(e5)*(sin(e2)*sin(e3) - cos(e2)*cos(e3))) + cos(e6)*sin(e4)*(sin(e2)*sin(e3) - cos(e2)*cos(e3)))*(x6*(sin(e2 + e3)*sin(e5) - cos(e2 + e3)*cos(e4)*cos(e5)) + z6*cos(e6)*(sin(e2 + e3)*cos(e5) + cos(e2 + e3)*cos(e4)*sin(e5)) - sin(e4)*sin(e5)*sin(e6)*(a1 + d4*cos(e2 + e3) + a3*sin(e2 + e3) + a2*sin(e2))) + (cos(e6)*(sin(e5)*(cos(e2)*sin(e3) + cos(e3)*sin(e2)) + cos(e4)*cos(e5)*(sin(e2)*sin(e3) - cos(e2)*cos(e3))) - sin(e4)*sin(e6)*(sin(e2)*sin(e3) - cos(e2)*cos(e3)))*(z6*sin(e6)*(sin(e2 + e3)*cos(e5) + cos(e2 + e3)*cos(e4)*sin(e5)) - y6*(sin(e2 + e3)*sin(e5) - cos(e2 + e3)*cos(e4)*cos(e5)) + cos(e6)*sin(e4)*sin(e5)*(a1 + d4*cos(e2 + e3) + a3*sin(e2 + e3) + a2*sin(e2))) + cos(e6)*(cos(e5)*(cos(e2)*sin(e3) + cos(e3)*sin(e2)) - cos(e4)*sin(e5)*(sin(e2)*sin(e3) - cos(e2)*cos(e3)))*(y6*(sin(e2 + e3)*cos(e5) + cos(e2 + e3)*cos(e4)*sin(e5)) + z6*(sin(e6)*(sin(e2 + e3)*sin(e5) - cos(e2 + e3)*cos(e4)*cos(e5)) - cos(e2 + e3)*cos(e6)*sin(e4)) - cos(e4)*sin(e6)*(a1 + d4*cos(e2 + e3) + a3*sin(e2 + e3) + a2*sin(e2)) - cos(e5)*cos(e6)*sin(e4)*(a1 + d4*cos(e2 + e3) + a3*sin(e2 + e3) + a2*sin(e2))) + sin(e6)*(cos(e5)*(cos(e2)*sin(e3) + cos(e3)*sin(e2)) - cos(e4)*sin(e5)*(sin(e2)*sin(e3) - cos(e2)*cos(e3)))*(x6*(sin(e2 + e3)*cos(e5) + cos(e2 + e3)*cos(e4)*sin(e5)) - z6*(cos(e6)*(sin(e2 + e3)*sin(e5) - cos(e2 + e3)*cos(e4)*cos(e5)) + cos(e2 + e3)*sin(e4)*sin(e6)) + cos(e4)*cos(e6)*(a1 + d4*cos(e2 + e3) + a3*sin(e2 + e3) + a2*sin(e2)) - cos(e5)*sin(e4)*sin(e6)*(a1 + d4*cos(e2 + e3) + a3*sin(e2 + e3) + a2*sin(e2)))) + m6*(y6*cos(e6)*(cos(e5)*(cos(e2)*cos(e3)*sin(e1) - sin(e1)*sin(e2)*sin(e3)) + sin(e5)*(cos(e1)*sin(e4) - cos(e4)*(cos(e2)*sin(e1)*sin(e3) + cos(e3)*sin(e1)*sin(e2)))) + x6*sin(e6)*(cos(e5)*(cos(e2)*cos(e3)*sin(e1) - sin(e1)*sin(e2)*sin(e3)) + sin(e5)*(cos(e1)*sin(e4) - cos(e4)*(cos(e2)*sin(e1)*sin(e3) + cos(e3)*sin(e1)*sin(e2)))))*((sin(e6)*(sin(e5)*(cos(e2)*cos(e3)*sin(e1) - sin(e1)*sin(e2)*sin(e3)) - cos(e5)*(cos(e1)*sin(e4) - cos(e4)*(cos(e2)*sin(e1)*sin(e3) + cos(e3)*sin(e1)*sin(e2)))) + cos(e6)*(sin(e4)*(cos(e2)*sin(e1)*sin(e3) + cos(e3)*sin(e1)*sin(e2)) + cos(e1)*cos(e4)))*(x6*(sin(e2 + e3)*cos(e5) + cos(e2 + e3)*cos(e4)*sin(e5)) - z6*(cos(e6)*(sin(e2 + e3)*sin(e5) - cos(e2 + e3)*cos(e4)*cos(e5)) + cos(e2 + e3)*sin(e4)*sin(e6)) + cos(e4)*cos(e6)*(a1 + d4*cos(e2 + e3) + a3*sin(e2 + e3) + a2*sin(e2)) - cos(e5)*sin(e4)*sin(e6)*(a1 + d4*cos(e2 + e3) + a3*sin(e2 + e3) + a2*sin(e2))) + (cos(e6)*(sin(e5)*(cos(e2)*cos(e3)*sin(e1) - sin(e1)*sin(e2)*sin(e3)) - cos(e5)*(cos(e1)*sin(e4) - cos(e4)*(cos(e2)*sin(e1)*sin(e3) + cos(e3)*sin(e1)*sin(e2)))) - sin(e6)*(sin(e4)*(cos(e2)*sin(e1)*sin(e3) + cos(e3)*sin(e1)*sin(e2)) + cos(e1)*cos(e4)))*(y6*(sin(e2 + e3)*cos(e5) + cos(e2 + e3)*cos(e4)*sin(e5)) + z6*(sin(e6)*(sin(e2 + e3)*sin(e5) - cos(e2 + e3)*cos(e4)*cos(e5)) - cos(e2 + e3)*cos(e6)*sin(e4)) - cos(e4)*sin(e6)*(a1 + d4*cos(e2 + e3) + a3*sin(e2 + e3) + a2*sin(e2)) - cos(e5)*cos(e6)*sin(e4)*(a1 + d4*cos(e2 + e3) + a3*sin(e2 + e3) + a2*sin(e2))) - (cos(e5)*(cos(e2)*cos(e3)*sin(e1) - sin(e1)*sin(e2)*sin(e3)) + sin(e5)*(cos(e1)*sin(e4) - cos(e4)*(cos(e2)*sin(e1)*sin(e3) + cos(e3)*sin(e1)*sin(e2))))*(x6*(sin(e6)*(sin(e2 + e3)*sin(e5) - cos(e2 + e3)*cos(e4)*cos(e5)) - cos(e2 + e3)*cos(e6)*sin(e4)) + y6*(cos(e6)*(sin(e2 + e3)*sin(e5) - cos(e2 + e3)*cos(e4)*cos(e5)) + cos(e2 + e3)*sin(e4)*sin(e6)) - sin(e4)*sin(e5)*(a1 + d4*cos(e2 + e3) + a3*sin(e2 + e3) + a2*sin(e2)))) + m6*(x6*(sin(e6)*(sin(e5)*(cos(e2)*cos(e3)*sin(e1) - sin(e1)*sin(e2)*sin(e3)) - cos(e5)*(cos(e1)*sin(e4) - cos(e4)*(cos(e2)*sin(e1)*sin(e3) + cos(e3)*sin(e1)*sin(e2)))) + cos(e6)*(sin(e4)*(cos(e2)*sin(e1)*sin(e3) + cos(e3)*sin(e1)*sin(e2)) + cos(e1)*cos(e4))) + y6*(cos(e6)*(sin(e5)*(cos(e2)*cos(e3)*sin(e1) - sin(e1)*sin(e2)*sin(e3)) - cos(e5)*(cos(e1)*sin(e4) - cos(e4)*(cos(e2)*sin(e1)*sin(e3) + cos(e3)*sin(e1)*sin(e2)))) - sin(e6)*(sin(e4)*(cos(e2)*sin(e1)*sin(e3) + cos(e3)*sin(e1)*sin(e2)) + cos(e1)*cos(e4))))*((cos(e6)*(sin(e5)*(cos(e2)*cos(e3)*sin(e1) - sin(e1)*sin(e2)*sin(e3)) - cos(e5)*(cos(e1)*sin(e4) - cos(e4)*(cos(e2)*sin(e1)*sin(e3) + cos(e3)*sin(e1)*sin(e2)))) - sin(e6)*(sin(e4)*(cos(e2)*sin(e1)*sin(e3) + cos(e3)*sin(e1)*sin(e2)) + cos(e1)*cos(e4)))*(z6*sin(e6)*(sin(e2 + e3)*cos(e5) + cos(e2 + e3)*cos(e4)*sin(e5)) - y6*(sin(e2 + e3)*sin(e5) - cos(e2 + e3)*cos(e4)*cos(e5)) + cos(e6)*sin(e4)*sin(e5)*(a1 + d4*cos(e2 + e3) + a3*sin(e2 + e3) + a2*sin(e2))) - (sin(e6)*(sin(e5)*(cos(e2)*cos(e3)*sin(e1) - sin(e1)*sin(e2)*sin(e3)) - cos(e5)*(cos(e1)*sin(e4) - cos(e4)*(cos(e2)*sin(e1)*sin(e3) + cos(e3)*sin(e1)*sin(e2)))) + cos(e6)*(sin(e4)*(cos(e2)*sin(e1)*sin(e3) + cos(e3)*sin(e1)*sin(e2)) + cos(e1)*cos(e4)))*(x6*(sin(e2 + e3)*sin(e5) - cos(e2 + e3)*cos(e4)*cos(e5)) + z6*cos(e6)*(sin(e2 + e3)*cos(e5) + cos(e2 + e3)*cos(e4)*sin(e5)) - sin(e4)*sin(e5)*sin(e6)*(a1 + d4*cos(e2 + e3) + a3*sin(e2 + e3) + a2*sin(e2))) + (sin(e5)*(cos(e2)*cos(e3)*sin(e1) - sin(e1)*sin(e2)*sin(e3)) - cos(e5)*(cos(e1)*sin(e4) - cos(e4)*(cos(e2)*sin(e1)*sin(e3) + cos(e3)*sin(e1)*sin(e2))))*(x6*(sin(e6)*(sin(e2 + e3)*sin(e5) - cos(e2 + e3)*cos(e4)*cos(e5)) - cos(e2 + e3)*cos(e6)*sin(e4)) + y6*(cos(e6)*(sin(e2 + e3)*sin(e5) - cos(e2 + e3)*cos(e4)*cos(e5)) + cos(e2 + e3)*sin(e4)*sin(e6)) - sin(e4)*sin(e5)*(a1 + d4*cos(e2 + e3) + a3*sin(e2 + e3) + a2*sin(e2))) - (cos(e5)*(cos(e2)*cos(e3)*sin(e1) - sin(e1)*sin(e2)*sin(e3)) + sin(e5)*(cos(e1)*sin(e4) - cos(e4)*(cos(e2)*sin(e1)*sin(e3) + cos(e3)*sin(e1)*sin(e2))))*(y6*cos(e6)*(sin(e2 + e3)*cos(e5) + cos(e2 + e3)*cos(e4)*sin(e5)) - cos(e5)*sin(e4)*(a1 + d4*cos(e2 + e3) + a3*sin(e2 + e3) + a2*sin(e2)) + x6*sin(e6)*(sin(e2 + e3)*cos(e5) + cos(e2 + e3)*cos(e4)*sin(e5))) + sin(e6)*(cos(e5)*(cos(e2)*cos(e3)*sin(e1) - sin(e1)*sin(e2)*sin(e3)) + sin(e5)*(cos(e1)*sin(e4) - cos(e4)*(cos(e2)*sin(e1)*sin(e3) + cos(e3)*sin(e1)*sin(e2))))*(x6*(sin(e2 + e3)*cos(e5) + cos(e2 + e3)*cos(e4)*sin(e5)) - z6*(cos(e6)*(sin(e2 + e3)*sin(e5) - cos(e2 + e3)*cos(e4)*cos(e5)) + cos(e2 + e3)*sin(e4)*sin(e6)) + cos(e4)*cos(e6)*(a1 + d4*cos(e2 + e3) + a3*sin(e2 + e3) + a2*sin(e2)) - cos(e5)*sin(e4)*sin(e6)*(a1 + d4*cos(e2 + e3) + a3*sin(e2 + e3) + a2*sin(e2))) + cos(e6)*(cos(e5)*(cos(e2)*cos(e3)*sin(e1) - sin(e1)*sin(e2)*sin(e3)) + sin(e5)*(cos(e1)*sin(e4) - cos(e4)*(cos(e2)*sin(e1)*sin(e3) + cos(e3)*sin(e1)*sin(e2))))*(y6*(sin(e2 + e3)*cos(e5) + cos(e2 + e3)*cos(e4)*sin(e5)) + z6*(sin(e6)*(sin(e2 + e3)*sin(e5) - cos(e2 + e3)*cos(e4)*cos(e5)) - cos(e2 + e3)*cos(e6)*sin(e4)) - cos(e4)*sin(e6)*(a1 + d4*cos(e2 + e3) + a3*sin(e2 + e3) + a2*sin(e2)) - cos(e5)*cos(e6)*sin(e4)*(a1 + d4*cos(e2 + e3) + a3*sin(e2 + e3) + a2*sin(e2)))) + m6*(y6*cos(e6)*(cos(e5)*(cos(e2)*sin(e3) + cos(e3)*sin(e2)) - cos(e4)*sin(e5)*(sin(e2)*sin(e3) - cos(e2)*cos(e3))) + x6*sin(e6)*(cos(e5)*(cos(e2)*sin(e3) + cos(e3)*sin(e2)) - cos(e4)*sin(e5)*(sin(e2)*sin(e3) - cos(e2)*cos(e3))))*((sin(e6)*(sin(e5)*(cos(e2)*sin(e3) + cos(e3)*sin(e2)) + cos(e4)*cos(e5)*(sin(e2)*sin(e3) - cos(e2)*cos(e3))) + cos(e6)*sin(e4)*(sin(e2)*sin(e3) - cos(e2)*cos(e3)))*(x6*(sin(e2 + e3)*cos(e5) + cos(e2 + e3)*cos(e4)*sin(e5)) - z6*(cos(e6)*(sin(e2 + e3)*sin(e5) - cos(e2 + e3)*cos(e4)*cos(e5)) + cos(e2 + e3)*sin(e4)*sin(e6)) + cos(e4)*cos(e6)*(a1 + d4*cos(e2 + e3) + a3*sin(e2 + e3) + a2*sin(e2)) - cos(e5)*sin(e4)*sin(e6)*(a1 + d4*cos(e2 + e3) + a3*sin(e2 + e3) + a2*sin(e2))) + (cos(e6)*(sin(e5)*(cos(e2)*sin(e3) + cos(e3)*sin(e2)) + cos(e4)*cos(e5)*(sin(e2)*sin(e3) - cos(e2)*cos(e3))) - sin(e4)*sin(e6)*(sin(e2)*sin(e3) - cos(e2)*cos(e3)))*(y6*(sin(e2 + e3)*cos(e5) + cos(e2 + e3)*cos(e4)*sin(e5)) + z6*(sin(e6)*(sin(e2 + e3)*sin(e5) - cos(e2 + e3)*cos(e4)*cos(e5)) - cos(e2 + e3)*cos(e6)*sin(e4)) - cos(e4)*sin(e6)*(a1 + d4*cos(e2 + e3) + a3*sin(e2 + e3) + a2*sin(e2)) - cos(e5)*cos(e6)*sin(e4)*(a1 + d4*cos(e2 + e3) + a3*sin(e2 + e3) + a2*sin(e2))) - (cos(e5)*(cos(e2)*sin(e3) + cos(e3)*sin(e2)) - cos(e4)*sin(e5)*(sin(e2)*sin(e3) - cos(e2)*cos(e3)))*(x6*(sin(e6)*(sin(e2 + e3)*sin(e5) - cos(e2 + e3)*cos(e4)*cos(e5)) - cos(e2 + e3)*cos(e6)*sin(e4)) + y6*(cos(e6)*(sin(e2 + e3)*sin(e5) - cos(e2 + e3)*cos(e4)*cos(e5)) + cos(e2 + e3)*sin(e4)*sin(e6)) - sin(e4)*sin(e5)*(a1 + d4*cos(e2 + e3) + a3*sin(e2 + e3) + a2*sin(e2))))) - de4*((I6xz*(cos(e2 + e3)*cos(e4)*sin(e6) + cos(e2 + e3)*cos(e5)*cos(e6)*sin(e4)))/2 + (I6yz*(cos(e2 + e3)*cos(e4)*cos(e6) - cos(e2 + e3)*cos(e5)*sin(e4)*sin(e6)))/2 + (I6zx*(cos(e2 + e3)*cos(e4)*sin(e6) + cos(e2 + e3)*cos(e5)*cos(e6)*sin(e4)))/2 + (I6zy*(cos(e2 + e3)*cos(e4)*cos(e6) - cos(e2 + e3)*cos(e5)*sin(e4)*sin(e6)))/2 + m6*(x6*(sin(e6)*(sin(e5)*(cos(e1)*cos(e2)*cos(e3) - cos(e1)*sin(e2)*sin(e3)) + cos(e5)*(sin(e1)*sin(e4) + cos(e4)*(cos(e1)*cos(e2)*sin(e3) + cos(e1)*cos(e3)*sin(e2)))) - cos(e6)*(cos(e4)*sin(e1) - sin(e4)*(cos(e1)*cos(e2)*sin(e3) + cos(e1)*cos(e3)*sin(e2)))) + y6*(cos(e6)*(sin(e5)*(cos(e1)*cos(e2)*cos(e3) - cos(e1)*sin(e2)*sin(e3)) + cos(e5)*(sin(e1)*sin(e4) + cos(e4)*(cos(e1)*cos(e2)*sin(e3) + cos(e1)*cos(e3)*sin(e2)))) + sin(e6)*(cos(e4)*sin(e1) - sin(e4)*(cos(e1)*cos(e2)*sin(e3) + cos(e1)*cos(e3)*sin(e2)))))*((cos(e5)*(cos(e1)*cos(e2)*cos(e3) - cos(e1)*sin(e2)*sin(e3)) - sin(e5)*(sin(e1)*sin(e4) + cos(e4)*(cos(e1)*cos(e2)*sin(e3) + cos(e1)*cos(e3)*sin(e2))))*(x6*(cos(e2 + e3)*cos(e4)*cos(e6) - cos(e2 + e3)*cos(e5)*sin(e4)*sin(e6)) - y6*(cos(e2 + e3)*cos(e4)*sin(e6) + cos(e2 + e3)*cos(e5)*cos(e6)*sin(e4)) + cos(e4)*sin(e5)*(a1 + d4*cos(e2 + e3) + a3*sin(e2 + e3) + a2*sin(e2))) - (sin(e6)*(sin(e5)*(cos(e1)*cos(e2)*cos(e3) - cos(e1)*sin(e2)*sin(e3)) + cos(e5)*(sin(e1)*sin(e4) + cos(e4)*(cos(e1)*cos(e2)*sin(e3) + cos(e1)*cos(e3)*sin(e2)))) - cos(e6)*(cos(e4)*sin(e1) - sin(e4)*(cos(e1)*cos(e2)*sin(e3) + cos(e1)*cos(e3)*sin(e2))))*(z6*(cos(e2 + e3)*cos(e4)*sin(e6) + cos(e2 + e3)*cos(e5)*cos(e6)*sin(e4)) + cos(e6)*sin(e4)*(a1 + d4*cos(e2 + e3) + a3*sin(e2 + e3) + a2*sin(e2)) + x6*cos(e2 + e3)*sin(e4)*sin(e5) + cos(e4)*cos(e5)*sin(e6)*(a1 + d4*cos(e2 + e3) + a3*sin(e2 + e3) + a2*sin(e2))) - (cos(e6)*(sin(e5)*(cos(e1)*cos(e2)*cos(e3) - cos(e1)*sin(e2)*sin(e3)) + cos(e5)*(sin(e1)*sin(e4) + cos(e4)*(cos(e1)*cos(e2)*sin(e3) + cos(e1)*cos(e3)*sin(e2)))) + sin(e6)*(cos(e4)*sin(e1) - sin(e4)*(cos(e1)*cos(e2)*sin(e3) + cos(e1)*cos(e3)*sin(e2))))*(z6*(cos(e2 + e3)*cos(e4)*cos(e6) - cos(e2 + e3)*cos(e5)*sin(e4)*sin(e6)) - sin(e4)*sin(e6)*(a1 + d4*cos(e2 + e3) + a3*sin(e2 + e3) + a2*sin(e2)) + y6*cos(e2 + e3)*sin(e4)*sin(e5) + cos(e4)*cos(e5)*cos(e6)*(a1 + d4*cos(e2 + e3) + a3*sin(e2 + e3) + a2*sin(e2))) + (cos(e6)*(sin(e1)*sin(e4) + cos(e4)*(cos(e1)*cos(e2)*sin(e3) + cos(e1)*cos(e3)*sin(e2))) + cos(e5)*sin(e6)*(cos(e4)*sin(e1) - sin(e4)*(cos(e1)*cos(e2)*sin(e3) + cos(e1)*cos(e3)*sin(e2))))*(x6*(sin(e2 + e3)*cos(e5) + cos(e2 + e3)*cos(e4)*sin(e5)) - z6*(cos(e6)*(sin(e2 + e3)*sin(e5) - cos(e2 + e3)*cos(e4)*cos(e5)) + cos(e2 + e3)*sin(e4)*sin(e6)) + cos(e4)*cos(e6)*(a1 + d4*cos(e2 + e3) + a3*sin(e2 + e3) + a2*sin(e2)) - cos(e5)*sin(e4)*sin(e6)*(a1 + d4*cos(e2 + e3) + a3*sin(e2 + e3) + a2*sin(e2))) - (sin(e6)*(sin(e1)*sin(e4) + cos(e4)*(cos(e1)*cos(e2)*sin(e3) + cos(e1)*cos(e3)*sin(e2))) - cos(e5)*cos(e6)*(cos(e4)*sin(e1) - sin(e4)*(cos(e1)*cos(e2)*sin(e3) + cos(e1)*cos(e3)*sin(e2))))*(y6*(sin(e2 + e3)*cos(e5) + cos(e2 + e3)*cos(e4)*sin(e5)) + z6*(sin(e6)*(sin(e2 + e3)*sin(e5) - cos(e2 + e3)*cos(e4)*cos(e5)) - cos(e2 + e3)*cos(e6)*sin(e4)) - cos(e4)*sin(e6)*(a1 + d4*cos(e2 + e3) + a3*sin(e2 + e3) + a2*sin(e2)) - cos(e5)*cos(e6)*sin(e4)*(a1 + d4*cos(e2 + e3) + a3*sin(e2 + e3) + a2*sin(e2))) + sin(e5)*(cos(e4)*sin(e1) - sin(e4)*(cos(e1)*cos(e2)*sin(e3) + cos(e1)*cos(e3)*sin(e2)))*(x6*(sin(e6)*(sin(e2 + e3)*sin(e5) - cos(e2 + e3)*cos(e4)*cos(e5)) - cos(e2 + e3)*cos(e6)*sin(e4)) + y6*(cos(e6)*(sin(e2 + e3)*sin(e5) - cos(e2 + e3)*cos(e4)*cos(e5)) + cos(e2 + e3)*sin(e4)*sin(e6)) - sin(e4)*sin(e5)*(a1 + d4*cos(e2 + e3) + a3*sin(e2 + e3) + a2*sin(e2)))) - m6*(x6*(cos(e6)*(cos(e1)*sin(e4) - cos(e4)*(cos(e2)*sin(e1)*sin(e3) + cos(e3)*sin(e1)*sin(e2))) + cos(e5)*sin(e6)*(sin(e4)*(cos(e2)*sin(e1)*sin(e3) + cos(e3)*sin(e1)*sin(e2)) + cos(e1)*cos(e4))) - y6*(sin(e6)*(cos(e1)*sin(e4) - cos(e4)*(cos(e2)*sin(e1)*sin(e3) + cos(e3)*sin(e1)*sin(e2))) - cos(e5)*cos(e6)*(sin(e4)*(cos(e2)*sin(e1)*sin(e3) + cos(e3)*sin(e1)*sin(e2)) + cos(e1)*cos(e4))))*((sin(e6)*(sin(e5)*(cos(e2)*cos(e3)*sin(e1) - sin(e1)*sin(e2)*sin(e3)) - cos(e5)*(cos(e1)*sin(e4) - cos(e4)*(cos(e2)*sin(e1)*sin(e3) + cos(e3)*sin(e1)*sin(e2)))) + cos(e6)*(sin(e4)*(cos(e2)*sin(e1)*sin(e3) + cos(e3)*sin(e1)*sin(e2)) + cos(e1)*cos(e4)))*(x6*(sin(e2 + e3)*cos(e5) + cos(e2 + e3)*cos(e4)*sin(e5)) - z6*(cos(e6)*(sin(e2 + e3)*sin(e5) - cos(e2 + e3)*cos(e4)*cos(e5)) + cos(e2 + e3)*sin(e4)*sin(e6)) + cos(e4)*cos(e6)*(a1 + d4*cos(e2 + e3) + a3*sin(e2 + e3) + a2*sin(e2)) - cos(e5)*sin(e4)*sin(e6)*(a1 + d4*cos(e2 + e3) + a3*sin(e2 + e3) + a2*sin(e2))) + (cos(e6)*(sin(e5)*(cos(e2)*cos(e3)*sin(e1) - sin(e1)*sin(e2)*sin(e3)) - cos(e5)*(cos(e1)*sin(e4) - cos(e4)*(cos(e2)*sin(e1)*sin(e3) + cos(e3)*sin(e1)*sin(e2)))) - sin(e6)*(sin(e4)*(cos(e2)*sin(e1)*sin(e3) + cos(e3)*sin(e1)*sin(e2)) + cos(e1)*cos(e4)))*(y6*(sin(e2 + e3)*cos(e5) + cos(e2 + e3)*cos(e4)*sin(e5)) + z6*(sin(e6)*(sin(e2 + e3)*sin(e5) - cos(e2 + e3)*cos(e4)*cos(e5)) - cos(e2 + e3)*cos(e6)*sin(e4)) - cos(e4)*sin(e6)*(a1 + d4*cos(e2 + e3) + a3*sin(e2 + e3) + a2*sin(e2)) - cos(e5)*cos(e6)*sin(e4)*(a1 + d4*cos(e2 + e3) + a3*sin(e2 + e3) + a2*sin(e2))) - (cos(e5)*(cos(e2)*cos(e3)*sin(e1) - sin(e1)*sin(e2)*sin(e3)) + sin(e5)*(cos(e1)*sin(e4) - cos(e4)*(cos(e2)*sin(e1)*sin(e3) + cos(e3)*sin(e1)*sin(e2))))*(x6*(sin(e6)*(sin(e2 + e3)*sin(e5) - cos(e2 + e3)*cos(e4)*cos(e5)) - cos(e2 + e3)*cos(e6)*sin(e4)) + y6*(cos(e6)*(sin(e2 + e3)*sin(e5) - cos(e2 + e3)*cos(e4)*cos(e5)) + cos(e2 + e3)*sin(e4)*sin(e6)) - sin(e4)*sin(e5)*(a1 + d4*cos(e2 + e3) + a3*sin(e2 + e3) + a2*sin(e2)))) + m6*(x6*(cos(e6)*(sin(e1)*sin(e4) + cos(e4)*(cos(e1)*cos(e2)*sin(e3) + cos(e1)*cos(e3)*sin(e2))) + cos(e5)*sin(e6)*(cos(e4)*sin(e1) - sin(e4)*(cos(e1)*cos(e2)*sin(e3) + cos(e1)*cos(e3)*sin(e2)))) - y6*(sin(e6)*(sin(e1)*sin(e4) + cos(e4)*(cos(e1)*cos(e2)*sin(e3) + cos(e1)*cos(e3)*sin(e2))) - cos(e5)*cos(e6)*(cos(e4)*sin(e1) - sin(e4)*(cos(e1)*cos(e2)*sin(e3) + cos(e1)*cos(e3)*sin(e2)))))*((sin(e6)*(sin(e5)*(cos(e1)*cos(e2)*cos(e3) - cos(e1)*sin(e2)*sin(e3)) + cos(e5)*(sin(e1)*sin(e4) + cos(e4)*(cos(e1)*cos(e2)*sin(e3) + cos(e1)*cos(e3)*sin(e2)))) - cos(e6)*(cos(e4)*sin(e1) - sin(e4)*(cos(e1)*cos(e2)*sin(e3) + cos(e1)*cos(e3)*sin(e2))))*(x6*(sin(e2 + e3)*cos(e5) + cos(e2 + e3)*cos(e4)*sin(e5)) - z6*(cos(e6)*(sin(e2 + e3)*sin(e5) - cos(e2 + e3)*cos(e4)*cos(e5)) + cos(e2 + e3)*sin(e4)*sin(e6)) + cos(e4)*cos(e6)*(a1 + d4*cos(e2 + e3) + a3*sin(e2 + e3) + a2*sin(e2)) - cos(e5)*sin(e4)*sin(e6)*(a1 + d4*cos(e2 + e3) + a3*sin(e2 + e3) + a2*sin(e2))) + (cos(e6)*(sin(e5)*(cos(e1)*cos(e2)*cos(e3) - cos(e1)*sin(e2)*sin(e3)) + cos(e5)*(sin(e1)*sin(e4) + cos(e4)*(cos(e1)*cos(e2)*sin(e3) + cos(e1)*cos(e3)*sin(e2)))) + sin(e6)*(cos(e4)*sin(e1) - sin(e4)*(cos(e1)*cos(e2)*sin(e3) + cos(e1)*cos(e3)*sin(e2))))*(y6*(sin(e2 + e3)*cos(e5) + cos(e2 + e3)*cos(e4)*sin(e5)) + z6*(sin(e6)*(sin(e2 + e3)*sin(e5) - cos(e2 + e3)*cos(e4)*cos(e5)) - cos(e2 + e3)*cos(e6)*sin(e4)) - cos(e4)*sin(e6)*(a1 + d4*cos(e2 + e3) + a3*sin(e2 + e3) + a2*sin(e2)) - cos(e5)*cos(e6)*sin(e4)*(a1 + d4*cos(e2 + e3) + a3*sin(e2 + e3) + a2*sin(e2))) - (cos(e5)*(cos(e1)*cos(e2)*cos(e3) - cos(e1)*sin(e2)*sin(e3)) - sin(e5)*(sin(e1)*sin(e4) + cos(e4)*(cos(e1)*cos(e2)*sin(e3) + cos(e1)*cos(e3)*sin(e2))))*(x6*(sin(e6)*(sin(e2 + e3)*sin(e5) - cos(e2 + e3)*cos(e4)*cos(e5)) - cos(e2 + e3)*cos(e6)*sin(e4)) + y6*(cos(e6)*(sin(e2 + e3)*sin(e5) - cos(e2 + e3)*cos(e4)*cos(e5)) + cos(e2 + e3)*sin(e4)*sin(e6)) - sin(e4)*sin(e5)*(a1 + d4*cos(e2 + e3) + a3*sin(e2 + e3) + a2*sin(e2)))) + m6*(x6*(cos(e4)*cos(e6)*(sin(e2)*sin(e3) - cos(e2)*cos(e3)) - cos(e5)*sin(e4)*sin(e6)*(sin(e2)*sin(e3) - cos(e2)*cos(e3))) - y6*(cos(e4)*sin(e6)*(sin(e2)*sin(e3) - cos(e2)*cos(e3)) + cos(e5)*cos(e6)*sin(e4)*(sin(e2)*sin(e3) - cos(e2)*cos(e3))))*((sin(e6)*(sin(e5)*(cos(e2)*sin(e3) + cos(e3)*sin(e2)) + cos(e4)*cos(e5)*(sin(e2)*sin(e3) - cos(e2)*cos(e3))) + cos(e6)*sin(e4)*(sin(e2)*sin(e3) - cos(e2)*cos(e3)))*(x6*(sin(e2 + e3)*cos(e5) + cos(e2 + e3)*cos(e4)*sin(e5)) - z6*(cos(e6)*(sin(e2 + e3)*sin(e5) - cos(e2 + e3)*cos(e4)*cos(e5)) + cos(e2 + e3)*sin(e4)*sin(e6)) + cos(e4)*cos(e6)*(a1 + d4*cos(e2 + e3) + a3*sin(e2 + e3) + a2*sin(e2)) - cos(e5)*sin(e4)*sin(e6)*(a1 + d4*cos(e2 + e3) + a3*sin(e2 + e3) + a2*sin(e2))) + (cos(e6)*(sin(e5)*(cos(e2)*sin(e3) + cos(e3)*sin(e2)) + cos(e4)*cos(e5)*(sin(e2)*sin(e3) - cos(e2)*cos(e3))) - sin(e4)*sin(e6)*(sin(e2)*sin(e3) - cos(e2)*cos(e3)))*(y6*(sin(e2 + e3)*cos(e5) + cos(e2 + e3)*cos(e4)*sin(e5)) + z6*(sin(e6)*(sin(e2 + e3)*sin(e5) - cos(e2 + e3)*cos(e4)*cos(e5)) - cos(e2 + e3)*cos(e6)*sin(e4)) - cos(e4)*sin(e6)*(a1 + d4*cos(e2 + e3) + a3*sin(e2 + e3) + a2*sin(e2)) - cos(e5)*cos(e6)*sin(e4)*(a1 + d4*cos(e2 + e3) + a3*sin(e2 + e3) + a2*sin(e2))) - (cos(e5)*(cos(e2)*sin(e3) + cos(e3)*sin(e2)) - cos(e4)*sin(e5)*(sin(e2)*sin(e3) - cos(e2)*cos(e3)))*(x6*(sin(e6)*(sin(e2 + e3)*sin(e5) - cos(e2 + e3)*cos(e4)*cos(e5)) - cos(e2 + e3)*cos(e6)*sin(e4)) + y6*(cos(e6)*(sin(e2 + e3)*sin(e5) - cos(e2 + e3)*cos(e4)*cos(e5)) + cos(e2 + e3)*sin(e4)*sin(e6)) - sin(e4)*sin(e5)*(a1 + d4*cos(e2 + e3) + a3*sin(e2 + e3) + a2*sin(e2)))) - m6*(x6*(sin(e6)*(sin(e5)*(cos(e2)*sin(e3) + cos(e3)*sin(e2)) + cos(e4)*cos(e5)*(sin(e2)*sin(e3) - cos(e2)*cos(e3))) + cos(e6)*sin(e4)*(sin(e2)*sin(e3) - cos(e2)*cos(e3))) + y6*(cos(e6)*(sin(e5)*(cos(e2)*sin(e3) + cos(e3)*sin(e2)) + cos(e4)*cos(e5)*(sin(e2)*sin(e3) - cos(e2)*cos(e3))) - sin(e4)*sin(e6)*(sin(e2)*sin(e3) - cos(e2)*cos(e3))))*((sin(e6)*(sin(e5)*(cos(e2)*sin(e3) + cos(e3)*sin(e2)) + cos(e4)*cos(e5)*(sin(e2)*sin(e3) - cos(e2)*cos(e3))) + cos(e6)*sin(e4)*(sin(e2)*sin(e3) - cos(e2)*cos(e3)))*(z6*(cos(e2 + e3)*cos(e4)*sin(e6) + cos(e2 + e3)*cos(e5)*cos(e6)*sin(e4)) + cos(e6)*sin(e4)*(a1 + d4*cos(e2 + e3) + a3*sin(e2 + e3) + a2*sin(e2)) + x6*cos(e2 + e3)*sin(e4)*sin(e5) + cos(e4)*cos(e5)*sin(e6)*(a1 + d4*cos(e2 + e3) + a3*sin(e2 + e3) + a2*sin(e2))) + (cos(e6)*(sin(e5)*(cos(e2)*sin(e3) + cos(e3)*sin(e2)) + cos(e4)*cos(e5)*(sin(e2)*sin(e3) - cos(e2)*cos(e3))) - sin(e4)*sin(e6)*(sin(e2)*sin(e3) - cos(e2)*cos(e3)))*(z6*(cos(e2 + e3)*cos(e4)*cos(e6) - cos(e2 + e3)*cos(e5)*sin(e4)*sin(e6)) - sin(e4)*sin(e6)*(a1 + d4*cos(e2 + e3) + a3*sin(e2 + e3) + a2*sin(e2)) + y6*cos(e2 + e3)*sin(e4)*sin(e5) + cos(e4)*cos(e5)*cos(e6)*(a1 + d4*cos(e2 + e3) + a3*sin(e2 + e3) + a2*sin(e2))) - (cos(e5)*(cos(e2)*sin(e3) + cos(e3)*sin(e2)) - cos(e4)*sin(e5)*(sin(e2)*sin(e3) - cos(e2)*cos(e3)))*(x6*(cos(e2 + e3)*cos(e4)*cos(e6) - cos(e2 + e3)*cos(e5)*sin(e4)*sin(e6)) - y6*(cos(e2 + e3)*cos(e4)*sin(e6) + cos(e2 + e3)*cos(e5)*cos(e6)*sin(e4)) + cos(e4)*sin(e5)*(a1 + d4*cos(e2 + e3) + a3*sin(e2 + e3) + a2*sin(e2))) - (cos(e4)*cos(e6)*(sin(e2)*sin(e3) - cos(e2)*cos(e3)) - cos(e5)*sin(e4)*sin(e6)*(sin(e2)*sin(e3) - cos(e2)*cos(e3)))*(x6*(sin(e2 + e3)*cos(e5) + cos(e2 + e3)*cos(e4)*sin(e5)) - z6*(cos(e6)*(sin(e2 + e3)*sin(e5) - cos(e2 + e3)*cos(e4)*cos(e5)) + cos(e2 + e3)*sin(e4)*sin(e6)) + cos(e4)*cos(e6)*(a1 + d4*cos(e2 + e3) + a3*sin(e2 + e3) + a2*sin(e2)) - cos(e5)*sin(e4)*sin(e6)*(a1 + d4*cos(e2 + e3) + a3*sin(e2 + e3) + a2*sin(e2))) + (cos(e4)*sin(e6)*(sin(e2)*sin(e3) - cos(e2)*cos(e3)) + cos(e5)*cos(e6)*sin(e4)*(sin(e2)*sin(e3) - cos(e2)*cos(e3)))*(y6*(sin(e2 + e3)*cos(e5) + cos(e2 + e3)*cos(e4)*sin(e5)) + z6*(sin(e6)*(sin(e2 + e3)*sin(e5) - cos(e2 + e3)*cos(e4)*cos(e5)) - cos(e2 + e3)*cos(e6)*sin(e4)) - cos(e4)*sin(e6)*(a1 + d4*cos(e2 + e3) + a3*sin(e2 + e3) + a2*sin(e2)) - cos(e5)*cos(e6)*sin(e4)*(a1 + d4*cos(e2 + e3) + a3*sin(e2 + e3) + a2*sin(e2))) + sin(e4)*sin(e5)*(sin(e2)*sin(e3) - cos(e2)*cos(e3))*(x6*(sin(e6)*(sin(e2 + e3)*sin(e5) - cos(e2 + e3)*cos(e4)*cos(e5)) - cos(e2 + e3)*cos(e6)*sin(e4)) + y6*(cos(e6)*(sin(e2 + e3)*sin(e5) - cos(e2 + e3)*cos(e4)*cos(e5)) + cos(e2 + e3)*sin(e4)*sin(e6)) - sin(e4)*sin(e5)*(a1 + d4*cos(e2 + e3) + a3*sin(e2 + e3) + a2*sin(e2)))) - m6*(x6*(sin(e6)*(sin(e5)*(cos(e2)*cos(e3)*sin(e1) - sin(e1)*sin(e2)*sin(e3)) - cos(e5)*(cos(e1)*sin(e4) - cos(e4)*(cos(e2)*sin(e1)*sin(e3) + cos(e3)*sin(e1)*sin(e2)))) + cos(e6)*(sin(e4)*(cos(e2)*sin(e1)*sin(e3) + cos(e3)*sin(e1)*sin(e2)) + cos(e1)*cos(e4))) + y6*(cos(e6)*(sin(e5)*(cos(e2)*cos(e3)*sin(e1) - sin(e1)*sin(e2)*sin(e3)) - cos(e5)*(cos(e1)*sin(e4) - cos(e4)*(cos(e2)*sin(e1)*sin(e3) + cos(e3)*sin(e1)*sin(e2)))) - sin(e6)*(sin(e4)*(cos(e2)*sin(e1)*sin(e3) + cos(e3)*sin(e1)*sin(e2)) + cos(e1)*cos(e4))))*((cos(e6)*(cos(e1)*sin(e4) - cos(e4)*(cos(e2)*sin(e1)*sin(e3) + cos(e3)*sin(e1)*sin(e2))) + cos(e5)*sin(e6)*(sin(e4)*(cos(e2)*sin(e1)*sin(e3) + cos(e3)*sin(e1)*sin(e2)) + cos(e1)*cos(e4)))*(x6*(sin(e2 + e3)*cos(e5) + cos(e2 + e3)*cos(e4)*sin(e5)) - z6*(cos(e6)*(sin(e2 + e3)*sin(e5) - cos(e2 + e3)*cos(e4)*cos(e5)) + cos(e2 + e3)*sin(e4)*sin(e6)) + cos(e4)*cos(e6)*(a1 + d4*cos(e2 + e3) + a3*sin(e2 + e3) + a2*sin(e2)) - cos(e5)*sin(e4)*sin(e6)*(a1 + d4*cos(e2 + e3) + a3*sin(e2 + e3) + a2*sin(e2))) - (cos(e5)*(cos(e2)*cos(e3)*sin(e1) - sin(e1)*sin(e2)*sin(e3)) + sin(e5)*(cos(e1)*sin(e4) - cos(e4)*(cos(e2)*sin(e1)*sin(e3) + cos(e3)*sin(e1)*sin(e2))))*(x6*(cos(e2 + e3)*cos(e4)*cos(e6) - cos(e2 + e3)*cos(e5)*sin(e4)*sin(e6)) - y6*(cos(e2 + e3)*cos(e4)*sin(e6) + cos(e2 + e3)*cos(e5)*cos(e6)*sin(e4)) + cos(e4)*sin(e5)*(a1 + d4*cos(e2 + e3) + a3*sin(e2 + e3) + a2*sin(e2))) + (sin(e6)*(sin(e5)*(cos(e2)*cos(e3)*sin(e1) - sin(e1)*sin(e2)*sin(e3)) - cos(e5)*(cos(e1)*sin(e4) - cos(e4)*(cos(e2)*sin(e1)*sin(e3) + cos(e3)*sin(e1)*sin(e2)))) + cos(e6)*(sin(e4)*(cos(e2)*sin(e1)*sin(e3) + cos(e3)*sin(e1)*sin(e2)) + cos(e1)*cos(e4)))*(z6*(cos(e2 + e3)*cos(e4)*sin(e6) + cos(e2 + e3)*cos(e5)*cos(e6)*sin(e4)) + cos(e6)*sin(e4)*(a1 + d4*cos(e2 + e3) + a3*sin(e2 + e3) + a2*sin(e2)) + x6*cos(e2 + e3)*sin(e4)*sin(e5) + cos(e4)*cos(e5)*sin(e6)*(a1 + d4*cos(e2 + e3) + a3*sin(e2 + e3) + a2*sin(e2))) - (sin(e6)*(cos(e1)*sin(e4) - cos(e4)*(cos(e2)*sin(e1)*sin(e3) + cos(e3)*sin(e1)*sin(e2))) - cos(e5)*cos(e6)*(sin(e4)*(cos(e2)*sin(e1)*sin(e3) + cos(e3)*sin(e1)*sin(e2)) + cos(e1)*cos(e4)))*(y6*(sin(e2 + e3)*cos(e5) + cos(e2 + e3)*cos(e4)*sin(e5)) + z6*(sin(e6)*(sin(e2 + e3)*sin(e5) - cos(e2 + e3)*cos(e4)*cos(e5)) - cos(e2 + e3)*cos(e6)*sin(e4)) - cos(e4)*sin(e6)*(a1 + d4*cos(e2 + e3) + a3*sin(e2 + e3) + a2*sin(e2)) - cos(e5)*cos(e6)*sin(e4)*(a1 + d4*cos(e2 + e3) + a3*sin(e2 + e3) + a2*sin(e2))) + (cos(e6)*(sin(e5)*(cos(e2)*cos(e3)*sin(e1) - sin(e1)*sin(e2)*sin(e3)) - cos(e5)*(cos(e1)*sin(e4) - cos(e4)*(cos(e2)*sin(e1)*sin(e3) + cos(e3)*sin(e1)*sin(e2)))) - sin(e6)*(sin(e4)*(cos(e2)*sin(e1)*sin(e3) + cos(e3)*sin(e1)*sin(e2)) + cos(e1)*cos(e4)))*(z6*(cos(e2 + e3)*cos(e4)*cos(e6) - cos(e2 + e3)*cos(e5)*sin(e4)*sin(e6)) - sin(e4)*sin(e6)*(a1 + d4*cos(e2 + e3) + a3*sin(e2 + e3) + a2*sin(e2)) + y6*cos(e2 + e3)*sin(e4)*sin(e5) + cos(e4)*cos(e5)*cos(e6)*(a1 + d4*cos(e2 + e3) + a3*sin(e2 + e3) + a2*sin(e2))) + sin(e5)*(sin(e4)*(cos(e2)*sin(e1)*sin(e3) + cos(e3)*sin(e1)*sin(e2)) + cos(e1)*cos(e4))*(x6*(sin(e6)*(sin(e2 + e3)*sin(e5) - cos(e2 + e3)*cos(e4)*cos(e5)) - cos(e2 + e3)*cos(e6)*sin(e4)) + y6*(cos(e6)*(sin(e2 + e3)*sin(e5) - cos(e2 + e3)*cos(e4)*cos(e5)) + cos(e2 + e3)*sin(e4)*sin(e6)) - sin(e4)*sin(e5)*(a1 + d4*cos(e2 + e3) + a3*sin(e2 + e3) + a2*sin(e2)))) - I6zz*cos(e2 + e3)*sin(e4)*sin(e5)) - (de6*(0.5*I6yz*(cos(e6)*(sin(e2 + e3)*sin(e5) - 1.0*cos(e2 + e3)*cos(e4)*cos(e5)) + cos(e2 + e3)*sin(e4)*sin(e6)) + 0.5*I6zy*(cos(e6)*(sin(e2 + e3)*sin(e5) - 1.0*cos(e2 + e3)*cos(e4)*cos(e5)) + cos(e2 + e3)*sin(e4)*sin(e6)) + 0.5*I6xz*(sin(e6)*(sin(e2 + e3)*sin(e5) - 1.0*cos(e2 + e3)*cos(e4)*cos(e5)) - 1.0*cos(e2 + e3)*cos(e6)*sin(e4)) + 0.5*I6zx*(sin(e6)*(sin(e2 + e3)*sin(e5) - 1.0*cos(e2 + e3)*cos(e4)*cos(e5)) - 1.0*cos(e2 + e3)*cos(e6)*sin(e4)) - m6*(x6*(sin(e6)*(sin(e5)*(cos(e1)*cos(e2)*cos(e3) - 1.0*cos(e1)*sin(e2)*sin(e3)) + cos(e5)*(sin(e1)*sin(e4) + cos(e4)*(cos(e1)*cos(e2)*sin(e3) + cos(e1)*cos(e3)*sin(e2)))) - 1.0*cos(e6)*(cos(e4)*sin(e1) - 1.0*sin(e4)*(cos(e1)*cos(e2)*sin(e3) + cos(e1)*cos(e3)*sin(e2)))) + y6*(sin(e6)*(cos(e4)*sin(e1) - 1.0*sin(e4)*(cos(e1)*cos(e2)*sin(e3) + cos(e1)*cos(e3)*sin(e2))) + cos(e6)*(sin(e5)*(cos(e1)*cos(e2)*cos(e3) - 1.0*cos(e1)*sin(e2)*sin(e3)) + cos(e5)*(sin(e1)*sin(e4) + cos(e4)*(cos(e1)*cos(e2)*sin(e3) + cos(e1)*cos(e3)*sin(e2))))))*(1.0*(sin(e6)*(cos(e4)*sin(e1) - 1.0*sin(e4)*(cos(e1)*cos(e2)*sin(e3) + cos(e1)*cos(e3)*sin(e2))) + cos(e6)*(sin(e5)*(cos(e1)*cos(e2)*cos(e3) - 1.0*cos(e1)*sin(e2)*sin(e3)) + cos(e5)*(sin(e1)*sin(e4) + cos(e4)*(cos(e1)*cos(e2)*sin(e3) + cos(e1)*cos(e3)*sin(e2)))))*(x6*(sin(e2 + e3)*cos(e5) + cos(e2 + e3)*cos(e4)*sin(e5)) - 1.0*z6*(cos(e6)*(sin(e2 + e3)*sin(e5) - 1.0*cos(e2 + e3)*cos(e4)*cos(e5)) + cos(e2 + e3)*sin(e4)*sin(e6)) + cos(e4)*cos(e6)*(a1 + d4*cos(e2 + e3) + a3*sin(e2 + e3) + a2*sin(e2)) - 1.0*cos(e5)*sin(e4)*sin(e6)*(a1 + d4*cos(e2 + e3) + a3*sin(e2 + e3) + a2*sin(e2))) - (sin(e6)*(sin(e5)*(cos(e1)*cos(e2)*cos(e3) - 1.0*cos(e1)*sin(e2)*sin(e3)) + cos(e5)*(sin(e1)*sin(e4) + cos(e4)*(cos(e1)*cos(e2)*sin(e3) + cos(e1)*cos(e3)*sin(e2)))) - 1.0*cos(e6)*(cos(e4)*sin(e1) - 1.0*sin(e4)*(cos(e1)*cos(e2)*sin(e3) + cos(e1)*cos(e3)*sin(e2))))*(cos(e4)*sin(e6)*(a1 + d4*cos(e2 + e3) + a3*sin(e2 + e3) + a2*sin(e2)) - 1.0*z6*(sin(e6)*(sin(e2 + e3)*sin(e5) - 1.0*cos(e2 + e3)*cos(e4)*cos(e5)) - 1.0*cos(e2 + e3)*cos(e6)*sin(e4)) + cos(e5)*cos(e6)*sin(e4)*(a1 + d4*cos(e2 + e3) + a3*sin(e2 + e3) + a2*sin(e2))) - (sin(e6)*(sin(e5)*(cos(e1)*cos(e2)*cos(e3) - 1.0*cos(e1)*sin(e2)*sin(e3)) + cos(e5)*(sin(e1)*sin(e4) + cos(e4)*(cos(e1)*cos(e2)*sin(e3) + cos(e1)*cos(e3)*sin(e2)))) - 1.0*cos(e6)*(cos(e4)*sin(e1) - 1.0*sin(e4)*(cos(e1)*cos(e2)*sin(e3) + cos(e1)*cos(e3)*sin(e2))))*(z6*(sin(e6)*(sin(e2 + e3)*sin(e5) - 1.0*cos(e2 + e3)*cos(e4)*cos(e5)) - 1.0*cos(e2 + e3)*cos(e6)*sin(e4)) + y6*(sin(e2 + e3)*cos(e5) + cos(e2 + e3)*cos(e4)*sin(e5)) - 1.0*cos(e4)*sin(e6)*(a1 + d4*cos(e2 + e3) + a3*sin(e2 + e3) + a2*sin(e2)) - 1.0*cos(e5)*cos(e6)*sin(e4)*(a1 + d4*cos(e2 + e3) + a3*sin(e2 + e3) + a2*sin(e2))) + 1.0*(sin(e6)*(cos(e4)*sin(e1) - 1.0*sin(e4)*(cos(e1)*cos(e2)*sin(e3) + cos(e1)*cos(e3)*sin(e2))) + cos(e6)*(sin(e5)*(cos(e1)*cos(e2)*cos(e3) - 1.0*cos(e1)*sin(e2)*sin(e3)) + cos(e5)*(sin(e1)*sin(e4) + cos(e4)*(cos(e1)*cos(e2)*sin(e3) + cos(e1)*cos(e3)*sin(e2)))))*(z6*(cos(e6)*(sin(e2 + e3)*sin(e5) - 1.0*cos(e2 + e3)*cos(e4)*cos(e5)) + cos(e2 + e3)*sin(e4)*sin(e6)) - 1.0*cos(e4)*cos(e6)*(a1 + d4*cos(e2 + e3) + a3*sin(e2 + e3) + a2*sin(e2)) + cos(e5)*sin(e4)*sin(e6)*(a1 + d4*cos(e2 + e3) + a3*sin(e2 + e3) + a2*sin(e2))) + (cos(e5)*(cos(e1)*cos(e2)*cos(e3) - 1.0*cos(e1)*sin(e2)*sin(e3)) - 1.0*sin(e5)*(sin(e1)*sin(e4) + cos(e4)*(cos(e1)*cos(e2)*sin(e3) + cos(e1)*cos(e3)*sin(e2))))*(1.0*y6*(sin(e6)*(sin(e2 + e3)*sin(e5) - 1.0*cos(e2 + e3)*cos(e4)*cos(e5)) - 1.0*cos(e2 + e3)*cos(e6)*sin(e4)) - x6*(cos(e6)*(sin(e2 + e3)*sin(e5) - 1.0*cos(e2 + e3)*cos(e4)*cos(e5)) + cos(e2 + e3)*sin(e4)*sin(e6)))) + 1.0*m6*(1.0*y6*(sin(e6)*(sin(e5)*(cos(e1)*cos(e2)*cos(e3) - 1.0*cos(e1)*sin(e2)*sin(e3)) + cos(e5)*(sin(e1)*sin(e4) + cos(e4)*(cos(e1)*cos(e2)*sin(e3) + cos(e1)*cos(e3)*sin(e2)))) - 1.0*cos(e6)*(cos(e4)*sin(e1) - 1.0*sin(e4)*(cos(e1)*cos(e2)*sin(e3) + cos(e1)*cos(e3)*sin(e2)))) - x6*(sin(e6)*(cos(e4)*sin(e1) - 1.0*sin(e4)*(cos(e1)*cos(e2)*sin(e3) + cos(e1)*cos(e3)*sin(e2))) + cos(e6)*(sin(e5)*(cos(e1)*cos(e2)*cos(e3) - 1.0*cos(e1)*sin(e2)*sin(e3)) + cos(e5)*(sin(e1)*sin(e4) + cos(e4)*(cos(e1)*cos(e2)*sin(e3) + cos(e1)*cos(e3)*sin(e2))))))*((sin(e6)*(sin(e5)*(cos(e1)*cos(e2)*cos(e3) - 1.0*cos(e1)*sin(e2)*sin(e3)) + cos(e5)*(sin(e1)*sin(e4) + cos(e4)*(cos(e1)*cos(e2)*sin(e3) + cos(e1)*cos(e3)*sin(e2)))) - 1.0*cos(e6)*(cos(e4)*sin(e1) - 1.0*sin(e4)*(cos(e1)*cos(e2)*sin(e3) + cos(e1)*cos(e3)*sin(e2))))*(x6*(sin(e2 + e3)*cos(e5) + cos(e2 + e3)*cos(e4)*sin(e5)) - 1.0*z6*(cos(e6)*(sin(e2 + e3)*sin(e5) - 1.0*cos(e2 + e3)*cos(e4)*cos(e5)) + cos(e2 + e3)*sin(e4)*sin(e6)) + cos(e4)*cos(e6)*(a1 + d4*cos(e2 + e3) + a3*sin(e2 + e3) + a2*sin(e2)) - 1.0*cos(e5)*sin(e4)*sin(e6)*(a1 + d4*cos(e2 + e3) + a3*sin(e2 + e3) + a2*sin(e2))) + (sin(e6)*(cos(e4)*sin(e1) - 1.0*sin(e4)*(cos(e1)*cos(e2)*sin(e3) + cos(e1)*cos(e3)*sin(e2))) + cos(e6)*(sin(e5)*(cos(e1)*cos(e2)*cos(e3) - 1.0*cos(e1)*sin(e2)*sin(e3)) + cos(e5)*(sin(e1)*sin(e4) + cos(e4)*(cos(e1)*cos(e2)*sin(e3) + cos(e1)*cos(e3)*sin(e2)))))*(z6*(sin(e6)*(sin(e2 + e3)*sin(e5) - 1.0*cos(e2 + e3)*cos(e4)*cos(e5)) - 1.0*cos(e2 + e3)*cos(e6)*sin(e4)) + y6*(sin(e2 + e3)*cos(e5) + cos(e2 + e3)*cos(e4)*sin(e5)) - 1.0*cos(e4)*sin(e6)*(a1 + d4*cos(e2 + e3) + a3*sin(e2 + e3) + a2*sin(e2)) - 1.0*cos(e5)*cos(e6)*sin(e4)*(a1 + d4*cos(e2 + e3) + a3*sin(e2 + e3) + a2*sin(e2))) - 1.0*(cos(e5)*(cos(e1)*cos(e2)*cos(e3) - 1.0*cos(e1)*sin(e2)*sin(e3)) - 1.0*sin(e5)*(sin(e1)*sin(e4) + cos(e4)*(cos(e1)*cos(e2)*sin(e3) + cos(e1)*cos(e3)*sin(e2))))*(x6*(sin(e6)*(sin(e2 + e3)*sin(e5) - 1.0*cos(e2 + e3)*cos(e4)*cos(e5)) - 1.0*cos(e2 + e3)*cos(e6)*sin(e4)) + y6*(cos(e6)*(sin(e2 + e3)*sin(e5) - 1.0*cos(e2 + e3)*cos(e4)*cos(e5)) + cos(e2 + e3)*sin(e4)*sin(e6)) - 1.0*sin(e4)*sin(e5)*(a1 + d4*cos(e2 + e3) + a3*sin(e2 + e3) + a2*sin(e2)))) + 1.0*m6*(1.0*y6*(sin(e6)*(sin(e5)*(cos(e2)*sin(e3) + cos(e3)*sin(e2)) + cos(e4)*cos(e5)*(sin(e2)*sin(e3) - 1.0*cos(e2)*cos(e3))) + cos(e6)*sin(e4)*(sin(e2)*sin(e3) - 1.0*cos(e2)*cos(e3))) - x6*(cos(e6)*(sin(e5)*(cos(e2)*sin(e3) + cos(e3)*sin(e2)) + cos(e4)*cos(e5)*(sin(e2)*sin(e3) - 1.0*cos(e2)*cos(e3))) - 1.0*sin(e4)*sin(e6)*(sin(e2)*sin(e3) - 1.0*cos(e2)*cos(e3))))*((sin(e6)*(sin(e5)*(cos(e2)*sin(e3) + cos(e3)*sin(e2)) + cos(e4)*cos(e5)*(sin(e2)*sin(e3) - 1.0*cos(e2)*cos(e3))) + cos(e6)*sin(e4)*(sin(e2)*sin(e3) - 1.0*cos(e2)*cos(e3)))*(x6*(sin(e2 + e3)*cos(e5) + cos(e2 + e3)*cos(e4)*sin(e5)) - 1.0*z6*(cos(e6)*(sin(e2 + e3)*sin(e5) - 1.0*cos(e2 + e3)*cos(e4)*cos(e5)) + cos(e2 + e3)*sin(e4)*sin(e6)) + cos(e4)*cos(e6)*(a1 + d4*cos(e2 + e3) + a3*sin(e2 + e3) + a2*sin(e2)) - 1.0*cos(e5)*sin(e4)*sin(e6)*(a1 + d4*cos(e2 + e3) + a3*sin(e2 + e3) + a2*sin(e2))) + (cos(e6)*(sin(e5)*(cos(e2)*sin(e3) + cos(e3)*sin(e2)) + cos(e4)*cos(e5)*(sin(e2)*sin(e3) - 1.0*cos(e2)*cos(e3))) - 1.0*sin(e4)*sin(e6)*(sin(e2)*sin(e3) - 1.0*cos(e2)*cos(e3)))*(z6*(sin(e6)*(sin(e2 + e3)*sin(e5) - 1.0*cos(e2 + e3)*cos(e4)*cos(e5)) - 1.0*cos(e2 + e3)*cos(e6)*sin(e4)) + y6*(sin(e2 + e3)*cos(e5) + cos(e2 + e3)*cos(e4)*sin(e5)) - 1.0*cos(e4)*sin(e6)*(a1 + d4*cos(e2 + e3) + a3*sin(e2 + e3) + a2*sin(e2)) - 1.0*cos(e5)*cos(e6)*sin(e4)*(a1 + d4*cos(e2 + e3) + a3*sin(e2 + e3) + a2*sin(e2))) - 1.0*(cos(e5)*(cos(e2)*sin(e3) + cos(e3)*sin(e2)) - 1.0*cos(e4)*sin(e5)*(sin(e2)*sin(e3) - 1.0*cos(e2)*cos(e3)))*(x6*(sin(e6)*(sin(e2 + e3)*sin(e5) - 1.0*cos(e2 + e3)*cos(e4)*cos(e5)) - 1.0*cos(e2 + e3)*cos(e6)*sin(e4)) + y6*(cos(e6)*(sin(e2 + e3)*sin(e5) - 1.0*cos(e2 + e3)*cos(e4)*cos(e5)) + cos(e2 + e3)*sin(e4)*sin(e6)) - 1.0*sin(e4)*sin(e5)*(a1 + d4*cos(e2 + e3) + a3*sin(e2 + e3) + a2*sin(e2)))) + m6*(x6*(sin(e6)*(1.0*cos(e5)*(cos(e1)*sin(e4) - 1.0*cos(e4)*(cos(e2)*sin(e1)*sin(e3) + cos(e3)*sin(e1)*sin(e2))) - sin(e5)*(cos(e2)*cos(e3)*sin(e1) - 1.0*sin(e1)*sin(e2)*sin(e3))) - cos(e6)*(sin(e4)*(cos(e2)*sin(e1)*sin(e3) + cos(e3)*sin(e1)*sin(e2)) + cos(e1)*cos(e4))) + y6*(cos(e6)*(1.0*cos(e5)*(cos(e1)*sin(e4) - 1.0*cos(e4)*(cos(e2)*sin(e1)*sin(e3) + cos(e3)*sin(e1)*sin(e2))) - sin(e5)*(cos(e2)*cos(e3)*sin(e1) - 1.0*sin(e1)*sin(e2)*sin(e3))) + 1.0*sin(e6)*(sin(e4)*(cos(e2)*sin(e1)*sin(e3) + cos(e3)*sin(e1)*sin(e2)) + cos(e1)*cos(e4))))*((1.0*y6*(sin(e6)*(sin(e2 + e3)*sin(e5) - 1.0*cos(e2 + e3)*cos(e4)*cos(e5)) - 1.0*cos(e2 + e3)*cos(e6)*sin(e4)) - x6*(cos(e6)*(sin(e2 + e3)*sin(e5) - 1.0*cos(e2 + e3)*cos(e4)*cos(e5)) + cos(e2 + e3)*sin(e4)*sin(e6)))*(sin(e5)*(cos(e1)*sin(e4) - 1.0*cos(e4)*(cos(e2)*sin(e1)*sin(e3) + cos(e3)*sin(e1)*sin(e2))) + cos(e5)*(cos(e2)*cos(e3)*sin(e1) - 1.0*sin(e1)*sin(e2)*sin(e3))) - 1.0*(cos(e6)*(1.0*cos(e5)*(cos(e1)*sin(e4) - 1.0*cos(e4)*(cos(e2)*sin(e1)*sin(e3) + cos(e3)*sin(e1)*sin(e2))) - sin(e5)*(cos(e2)*cos(e3)*sin(e1) - 1.0*sin(e1)*sin(e2)*sin(e3))) + 1.0*sin(e6)*(sin(e4)*(cos(e2)*sin(e1)*sin(e3) + cos(e3)*sin(e1)*sin(e2)) + cos(e1)*cos(e4)))*(x6*(sin(e2 + e3)*cos(e5) + cos(e2 + e3)*cos(e4)*sin(e5)) - 1.0*z6*(cos(e6)*(sin(e2 + e3)*sin(e5) - 1.0*cos(e2 + e3)*cos(e4)*cos(e5)) + cos(e2 + e3)*sin(e4)*sin(e6)) + cos(e4)*cos(e6)*(a1 + d4*cos(e2 + e3) + a3*sin(e2 + e3) + a2*sin(e2)) - 1.0*cos(e5)*sin(e4)*sin(e6)*(a1 + d4*cos(e2 + e3) + a3*sin(e2 + e3) + a2*sin(e2))) + (sin(e6)*(1.0*cos(e5)*(cos(e1)*sin(e4) - 1.0*cos(e4)*(cos(e2)*sin(e1)*sin(e3) + cos(e3)*sin(e1)*sin(e2))) - sin(e5)*(cos(e2)*cos(e3)*sin(e1) - 1.0*sin(e1)*sin(e2)*sin(e3))) - cos(e6)*(sin(e4)*(cos(e2)*sin(e1)*sin(e3) + cos(e3)*sin(e1)*sin(e2)) + cos(e1)*cos(e4)))*(z6*(sin(e6)*(sin(e2 + e3)*sin(e5) - 1.0*cos(e2 + e3)*cos(e4)*cos(e5)) - 1.0*cos(e2 + e3)*cos(e6)*sin(e4)) + y6*(sin(e2 + e3)*cos(e5) + cos(e2 + e3)*cos(e4)*sin(e5)) - 1.0*cos(e4)*sin(e6)*(a1 + d4*cos(e2 + e3) + a3*sin(e2 + e3) + a2*sin(e2)) - 1.0*cos(e5)*cos(e6)*sin(e4)*(a1 + d4*cos(e2 + e3) + a3*sin(e2 + e3) + a2*sin(e2))) - 1.0*(cos(e6)*(1.0*cos(e5)*(cos(e1)*sin(e4) - 1.0*cos(e4)*(cos(e2)*sin(e1)*sin(e3) + cos(e3)*sin(e1)*sin(e2))) - sin(e5)*(cos(e2)*cos(e3)*sin(e1) - 1.0*sin(e1)*sin(e2)*sin(e3))) + 1.0*sin(e6)*(sin(e4)*(cos(e2)*sin(e1)*sin(e3) + cos(e3)*sin(e1)*sin(e2)) + cos(e1)*cos(e4)))*(z6*(cos(e6)*(sin(e2 + e3)*sin(e5) - 1.0*cos(e2 + e3)*cos(e4)*cos(e5)) + cos(e2 + e3)*sin(e4)*sin(e6)) - 1.0*cos(e4)*cos(e6)*(a1 + d4*cos(e2 + e3) + a3*sin(e2 + e3) + a2*sin(e2)) + cos(e5)*sin(e4)*sin(e6)*(a1 + d4*cos(e2 + e3) + a3*sin(e2 + e3) + a2*sin(e2))) + (sin(e6)*(1.0*cos(e5)*(cos(e1)*sin(e4) - 1.0*cos(e4)*(cos(e2)*sin(e1)*sin(e3) + cos(e3)*sin(e1)*sin(e2))) - sin(e5)*(cos(e2)*cos(e3)*sin(e1) - 1.0*sin(e1)*sin(e2)*sin(e3))) - cos(e6)*(sin(e4)*(cos(e2)*sin(e1)*sin(e3) + cos(e3)*sin(e1)*sin(e2)) + cos(e1)*cos(e4)))*(cos(e4)*sin(e6)*(a1 + d4*cos(e2 + e3) + a3*sin(e2 + e3) + a2*sin(e2)) - 1.0*z6*(sin(e6)*(sin(e2 + e3)*sin(e5) - 1.0*cos(e2 + e3)*cos(e4)*cos(e5)) - 1.0*cos(e2 + e3)*cos(e6)*sin(e4)) + cos(e5)*cos(e6)*sin(e4)*(a1 + d4*cos(e2 + e3) + a3*sin(e2 + e3) + a2*sin(e2)))) + 1.0*m6*(1.0*y6*(sin(e6)*(1.0*cos(e5)*(cos(e1)*sin(e4) - 1.0*cos(e4)*(cos(e2)*sin(e1)*sin(e3) + cos(e3)*sin(e1)*sin(e2))) - sin(e5)*(cos(e2)*cos(e3)*sin(e1) - 1.0*sin(e1)*sin(e2)*sin(e3))) - cos(e6)*(sin(e4)*(cos(e2)*sin(e1)*sin(e3) + cos(e3)*sin(e1)*sin(e2)) + cos(e1)*cos(e4))) - x6*(cos(e6)*(1.0*cos(e5)*(cos(e1)*sin(e4) - 1.0*cos(e4)*(cos(e2)*sin(e1)*sin(e3) + cos(e3)*sin(e1)*sin(e2))) - sin(e5)*(cos(e2)*cos(e3)*sin(e1) - 1.0*sin(e1)*sin(e2)*sin(e3))) + 1.0*sin(e6)*(sin(e4)*(cos(e2)*sin(e1)*sin(e3) + cos(e3)*sin(e1)*sin(e2)) + cos(e1)*cos(e4))))*((sin(e6)*(1.0*cos(e5)*(cos(e1)*sin(e4) - 1.0*cos(e4)*(cos(e2)*sin(e1)*sin(e3) + cos(e3)*sin(e1)*sin(e2))) - sin(e5)*(cos(e2)*cos(e3)*sin(e1) - 1.0*sin(e1)*sin(e2)*sin(e3))) - cos(e6)*(sin(e4)*(cos(e2)*sin(e1)*sin(e3) + cos(e3)*sin(e1)*sin(e2)) + cos(e1)*cos(e4)))*(x6*(sin(e2 + e3)*cos(e5) + cos(e2 + e3)*cos(e4)*sin(e5)) - 1.0*z6*(cos(e6)*(sin(e2 + e3)*sin(e5) - 1.0*cos(e2 + e3)*cos(e4)*cos(e5)) + cos(e2 + e3)*sin(e4)*sin(e6)) + cos(e4)*cos(e6)*(a1 + d4*cos(e2 + e3) + a3*sin(e2 + e3) + a2*sin(e2)) - 1.0*cos(e5)*sin(e4)*sin(e6)*(a1 + d4*cos(e2 + e3) + a3*sin(e2 + e3) + a2*sin(e2))) + 1.0*(sin(e5)*(cos(e1)*sin(e4) - 1.0*cos(e4)*(cos(e2)*sin(e1)*sin(e3) + cos(e3)*sin(e1)*sin(e2))) + cos(e5)*(cos(e2)*cos(e3)*sin(e1) - 1.0*sin(e1)*sin(e2)*sin(e3)))*(x6*(sin(e6)*(sin(e2 + e3)*sin(e5) - 1.0*cos(e2 + e3)*cos(e4)*cos(e5)) - 1.0*cos(e2 + e3)*cos(e6)*sin(e4)) + y6*(cos(e6)*(sin(e2 + e3)*sin(e5) - 1.0*cos(e2 + e3)*cos(e4)*cos(e5)) + cos(e2 + e3)*sin(e4)*sin(e6)) - 1.0*sin(e4)*sin(e5)*(a1 + d4*cos(e2 + e3) + a3*sin(e2 + e3) + a2*sin(e2))) + (cos(e6)*(1.0*cos(e5)*(cos(e1)*sin(e4) - 1.0*cos(e4)*(cos(e2)*sin(e1)*sin(e3) + cos(e3)*sin(e1)*sin(e2))) - sin(e5)*(cos(e2)*cos(e3)*sin(e1) - 1.0*sin(e1)*sin(e2)*sin(e3))) + 1.0*sin(e6)*(sin(e4)*(cos(e2)*sin(e1)*sin(e3) + cos(e3)*sin(e1)*sin(e2)) + cos(e1)*cos(e4)))*(z6*(sin(e6)*(sin(e2 + e3)*sin(e5) - 1.0*cos(e2 + e3)*cos(e4)*cos(e5)) - 1.0*cos(e2 + e3)*cos(e6)*sin(e4)) + y6*(sin(e2 + e3)*cos(e5) + cos(e2 + e3)*cos(e4)*sin(e5)) - 1.0*cos(e4)*sin(e6)*(a1 + d4*cos(e2 + e3) + a3*sin(e2 + e3) + a2*sin(e2)) - 1.0*cos(e5)*cos(e6)*sin(e4)*(a1 + d4*cos(e2 + e3) + a3*sin(e2 + e3) + a2*sin(e2)))) - m6*(x6*(sin(e6)*(sin(e5)*(cos(e2)*sin(e3) + cos(e3)*sin(e2)) + cos(e4)*cos(e5)*(sin(e2)*sin(e3) - 1.0*cos(e2)*cos(e3))) + cos(e6)*sin(e4)*(sin(e2)*sin(e3) - 1.0*cos(e2)*cos(e3))) + y6*(cos(e6)*(sin(e5)*(cos(e2)*sin(e3) + cos(e3)*sin(e2)) + cos(e4)*cos(e5)*(sin(e2)*sin(e3) - 1.0*cos(e2)*cos(e3))) - 1.0*sin(e4)*sin(e6)*(sin(e2)*sin(e3) - 1.0*cos(e2)*cos(e3))))*(1.0*(cos(e6)*(sin(e5)*(cos(e2)*sin(e3) + cos(e3)*sin(e2)) + cos(e4)*cos(e5)*(sin(e2)*sin(e3) - 1.0*cos(e2)*cos(e3))) - 1.0*sin(e4)*sin(e6)*(sin(e2)*sin(e3) - 1.0*cos(e2)*cos(e3)))*(x6*(sin(e2 + e3)*cos(e5) + cos(e2 + e3)*cos(e4)*sin(e5)) - 1.0*z6*(cos(e6)*(sin(e2 + e3)*sin(e5) - 1.0*cos(e2 + e3)*cos(e4)*cos(e5)) + cos(e2 + e3)*sin(e4)*sin(e6)) + cos(e4)*cos(e6)*(a1 + d4*cos(e2 + e3) + a3*sin(e2 + e3) + a2*sin(e2)) - 1.0*cos(e5)*sin(e4)*sin(e6)*(a1 + d4*cos(e2 + e3) + a3*sin(e2 + e3) + a2*sin(e2))) - (sin(e6)*(sin(e5)*(cos(e2)*sin(e3) + cos(e3)*sin(e2)) + cos(e4)*cos(e5)*(sin(e2)*sin(e3) - 1.0*cos(e2)*cos(e3))) + cos(e6)*sin(e4)*(sin(e2)*sin(e3) - 1.0*cos(e2)*cos(e3)))*(z6*(sin(e6)*(sin(e2 + e3)*sin(e5) - 1.0*cos(e2 + e3)*cos(e4)*cos(e5)) - 1.0*cos(e2 + e3)*cos(e6)*sin(e4)) + y6*(sin(e2 + e3)*cos(e5) + cos(e2 + e3)*cos(e4)*sin(e5)) - 1.0*cos(e4)*sin(e6)*(a1 + d4*cos(e2 + e3) + a3*sin(e2 + e3) + a2*sin(e2)) - 1.0*cos(e5)*cos(e6)*sin(e4)*(a1 + d4*cos(e2 + e3) + a3*sin(e2 + e3) + a2*sin(e2))) - (sin(e6)*(sin(e5)*(cos(e2)*sin(e3) + cos(e3)*sin(e2)) + cos(e4)*cos(e5)*(sin(e2)*sin(e3) - 1.0*cos(e2)*cos(e3))) + cos(e6)*sin(e4)*(sin(e2)*sin(e3) - 1.0*cos(e2)*cos(e3)))*(cos(e4)*sin(e6)*(a1 + d4*cos(e2 + e3) + a3*sin(e2 + e3) + a2*sin(e2)) - 1.0*z6*(sin(e6)*(sin(e2 + e3)*sin(e5) - 1.0*cos(e2 + e3)*cos(e4)*cos(e5)) - 1.0*cos(e2 + e3)*cos(e6)*sin(e4)) + cos(e5)*cos(e6)*sin(e4)*(a1 + d4*cos(e2 + e3) + a3*sin(e2 + e3) + a2*sin(e2))) + 1.0*(cos(e6)*(sin(e5)*(cos(e2)*sin(e3) + cos(e3)*sin(e2)) + cos(e4)*cos(e5)*(sin(e2)*sin(e3) - 1.0*cos(e2)*cos(e3))) - 1.0*sin(e4)*sin(e6)*(sin(e2)*sin(e3) - 1.0*cos(e2)*cos(e3)))*(z6*(cos(e6)*(sin(e2 + e3)*sin(e5) - 1.0*cos(e2 + e3)*cos(e4)*cos(e5)) + cos(e2 + e3)*sin(e4)*sin(e6)) - 1.0*cos(e4)*cos(e6)*(a1 + d4*cos(e2 + e3) + a3*sin(e2 + e3) + a2*sin(e2)) + cos(e5)*sin(e4)*sin(e6)*(a1 + d4*cos(e2 + e3) + a3*sin(e2 + e3) + a2*sin(e2))) + (1.0*y6*(sin(e6)*(sin(e2 + e3)*sin(e5) - 1.0*cos(e2 + e3)*cos(e4)*cos(e5)) - 1.0*cos(e2 + e3)*cos(e6)*sin(e4)) - x6*(cos(e6)*(sin(e2 + e3)*sin(e5) - 1.0*cos(e2 + e3)*cos(e4)*cos(e5)) + cos(e2 + e3)*sin(e4)*sin(e6)))*(cos(e5)*(cos(e2)*sin(e3) + cos(e3)*sin(e2)) - 1.0*cos(e4)*sin(e5)*(sin(e2)*sin(e3) - 1.0*cos(e2)*cos(e3))))))/2 + (de5*(0.5*(I6yx*cos(e6) + I6xx*sin(e6))*(sin(e6)*(sin(e2 + e3)*sin(e5) - 1.0*cos(e2 + e3)*cos(e4)*cos(e5)) - 1.0*cos(e2 + e3)*cos(e6)*sin(e4)) - 0.5*(cos(e6)*(sin(e2 + e3)*sin(e5) - 1.0*cos(e2 + e3)*cos(e4)*cos(e5)) + cos(e2 + e3)*sin(e4)*sin(e6))*(I6xx*cos(e6) - 1.0*I6yx*sin(e6)) + 0.5*cos(e6)*(I6yy*(cos(e6)*(sin(e2 + e3)*sin(e5) - 1.0*cos(e2 + e3)*cos(e4)*cos(e5)) + cos(e2 + e3)*sin(e4)*sin(e6)) + I6xy*(sin(e6)*(sin(e2 + e3)*sin(e5) - 1.0*cos(e2 + e3)*cos(e4)*cos(e5)) - 1.0*cos(e2 + e3)*cos(e6)*sin(e4))) + 0.5*(sin(e6)*(sin(e2 + e3)*sin(e5) - 1.0*cos(e2 + e3)*cos(e4)*cos(e5)) - 1.0*cos(e2 + e3)*cos(e6)*sin(e4))*(I6xy*cos(e6) - 1.0*I6yy*sin(e6)) + 0.5*sin(e6)*(I6yx*(cos(e6)*(sin(e2 + e3)*sin(e5) - 1.0*cos(e2 + e3)*cos(e4)*cos(e5)) + cos(e2 + e3)*sin(e4)*sin(e6)) + I6xx*(sin(e6)*(sin(e2 + e3)*sin(e5) - 1.0*cos(e2 + e3)*cos(e4)*cos(e5)) - 1.0*cos(e2 + e3)*cos(e6)*sin(e4))) - 0.5*(I6xz*cos(e6) - 1.0*I6yz*sin(e6))*(sin(e2 + e3)*cos(e5) + cos(e2 + e3)*cos(e4)*sin(e5)) + 0.5*(cos(e6)*(sin(e2 + e3)*sin(e5) - 1.0*cos(e2 + e3)*cos(e4)*cos(e5)) + cos(e2 + e3)*sin(e4)*sin(e6))*(I6yy*cos(e6) + I6xy*sin(e6)) - 0.5*cos(e6)*(I6zx*(sin(e2 + e3)*cos(e5) + cos(e2 + e3)*cos(e4)*sin(e5)) + I6xx*(cos(e6)*(sin(e2 + e3)*sin(e5) - 1.0*cos(e2 + e3)*cos(e4)*cos(e5)) + cos(e2 + e3)*sin(e4)*sin(e6)) - 1.0*I6yx*(sin(e6)*(sin(e2 + e3)*sin(e5) - 1.0*cos(e2 + e3)*cos(e4)*cos(e5)) - 1.0*cos(e2 + e3)*cos(e6)*sin(e4))) + 0.5*sin(e6)*(I6zy*(sin(e2 + e3)*cos(e5) + cos(e2 + e3)*cos(e4)*sin(e5)) + I6xy*(cos(e6)*(sin(e2 + e3)*sin(e5) - 1.0*cos(e2 + e3)*cos(e4)*cos(e5)) + cos(e2 + e3)*sin(e4)*sin(e6)) - 1.0*I6yy*(sin(e6)*(sin(e2 + e3)*sin(e5) - 1.0*cos(e2 + e3)*cos(e4)*cos(e5)) - 1.0*cos(e2 + e3)*cos(e6)*sin(e4))) + m6*(z6*cos(e6)*(sin(e6)*(cos(e4)*sin(e1) - 1.0*sin(e4)*(cos(e1)*cos(e2)*sin(e3) + cos(e1)*cos(e3)*sin(e2))) + cos(e6)*(sin(e5)*(cos(e1)*cos(e2)*cos(e3) - 1.0*cos(e1)*sin(e2)*sin(e3)) + cos(e5)*(sin(e1)*sin(e4) + cos(e4)*(cos(e1)*cos(e2)*sin(e3) + cos(e1)*cos(e3)*sin(e2))))) - 1.0*(cos(e5)*(cos(e1)*cos(e2)*cos(e3) - 1.0*cos(e1)*sin(e2)*sin(e3)) - 1.0*sin(e5)*(sin(e1)*sin(e4) + cos(e4)*(cos(e1)*cos(e2)*sin(e3) + cos(e1)*cos(e3)*sin(e2))))*(x6*cos(e6) - 1.0*y6*sin(e6)) + z6*sin(e6)*(sin(e6)*(sin(e5)*(cos(e1)*cos(e2)*cos(e3) - 1.0*cos(e1)*sin(e2)*sin(e3)) + cos(e5)*(sin(e1)*sin(e4) + cos(e4)*(cos(e1)*cos(e2)*sin(e3) + cos(e1)*cos(e3)*sin(e2)))) - 1.0*cos(e6)*(cos(e4)*sin(e1) - 1.0*sin(e4)*(cos(e1)*cos(e2)*sin(e3) + cos(e1)*cos(e3)*sin(e2)))))*(1.0*(sin(e6)*(cos(e4)*sin(e1) - 1.0*sin(e4)*(cos(e1)*cos(e2)*sin(e3) + cos(e1)*cos(e3)*sin(e2))) + cos(e6)*(sin(e5)*(cos(e1)*cos(e2)*cos(e3) - 1.0*cos(e1)*sin(e2)*sin(e3)) + cos(e5)*(sin(e1)*sin(e4) + cos(e4)*(cos(e1)*cos(e2)*sin(e3) + cos(e1)*cos(e3)*sin(e2)))))*(x6*(sin(e2 + e3)*cos(e5) + cos(e2 + e3)*cos(e4)*sin(e5)) - 1.0*z6*(cos(e6)*(sin(e2 + e3)*sin(e5) - 1.0*cos(e2 + e3)*cos(e4)*cos(e5)) + cos(e2 + e3)*sin(e4)*sin(e6)) + cos(e4)*cos(e6)*(a1 + d4*cos(e2 + e3) + a3*sin(e2 + e3) + a2*sin(e2)) - 1.0*cos(e5)*sin(e4)*sin(e6)*(a1 + d4*cos(e2 + e3) + a3*sin(e2 + e3) + a2*sin(e2))) - (sin(e6)*(sin(e5)*(cos(e1)*cos(e2)*cos(e3) - 1.0*cos(e1)*sin(e2)*sin(e3)) + cos(e5)*(sin(e1)*sin(e4) + cos(e4)*(cos(e1)*cos(e2)*sin(e3) + cos(e1)*cos(e3)*sin(e2)))) - 1.0*cos(e6)*(cos(e4)*sin(e1) - 1.0*sin(e4)*(cos(e1)*cos(e2)*sin(e3) + cos(e1)*cos(e3)*sin(e2))))*(cos(e4)*sin(e6)*(a1 + d4*cos(e2 + e3) + a3*sin(e2 + e3) + a2*sin(e2)) - 1.0*z6*(sin(e6)*(sin(e2 + e3)*sin(e5) - 1.0*cos(e2 + e3)*cos(e4)*cos(e5)) - 1.0*cos(e2 + e3)*cos(e6)*sin(e4)) + cos(e5)*cos(e6)*sin(e4)*(a1 + d4*cos(e2 + e3) + a3*sin(e2 + e3) + a2*sin(e2))) - (sin(e6)*(sin(e5)*(cos(e1)*cos(e2)*cos(e3) - 1.0*cos(e1)*sin(e2)*sin(e3)) + cos(e5)*(sin(e1)*sin(e4) + cos(e4)*(cos(e1)*cos(e2)*sin(e3) + cos(e1)*cos(e3)*sin(e2)))) - 1.0*cos(e6)*(cos(e4)*sin(e1) - 1.0*sin(e4)*(cos(e1)*cos(e2)*sin(e3) + cos(e1)*cos(e3)*sin(e2))))*(z6*(sin(e6)*(sin(e2 + e3)*sin(e5) - 1.0*cos(e2 + e3)*cos(e4)*cos(e5)) - 1.0*cos(e2 + e3)*cos(e6)*sin(e4)) + y6*(sin(e2 + e3)*cos(e5) + cos(e2 + e3)*cos(e4)*sin(e5)) - 1.0*cos(e4)*sin(e6)*(a1 + d4*cos(e2 + e3) + a3*sin(e2 + e3) + a2*sin(e2)) - 1.0*cos(e5)*cos(e6)*sin(e4)*(a1 + d4*cos(e2 + e3) + a3*sin(e2 + e3) + a2*sin(e2))) + 1.0*(sin(e6)*(cos(e4)*sin(e1) - 1.0*sin(e4)*(cos(e1)*cos(e2)*sin(e3) + cos(e1)*cos(e3)*sin(e2))) + cos(e6)*(sin(e5)*(cos(e1)*cos(e2)*cos(e3) - 1.0*cos(e1)*sin(e2)*sin(e3)) + cos(e5)*(sin(e1)*sin(e4) + cos(e4)*(cos(e1)*cos(e2)*sin(e3) + cos(e1)*cos(e3)*sin(e2)))))*(z6*(cos(e6)*(sin(e2 + e3)*sin(e5) - 1.0*cos(e2 + e3)*cos(e4)*cos(e5)) + cos(e2 + e3)*sin(e4)*sin(e6)) - 1.0*cos(e4)*cos(e6)*(a1 + d4*cos(e2 + e3) + a3*sin(e2 + e3) + a2*sin(e2)) + cos(e5)*sin(e4)*sin(e6)*(a1 + d4*cos(e2 + e3) + a3*sin(e2 + e3) + a2*sin(e2))) + (cos(e5)*(cos(e1)*cos(e2)*cos(e3) - 1.0*cos(e1)*sin(e2)*sin(e3)) - 1.0*sin(e5)*(sin(e1)*sin(e4) + cos(e4)*(cos(e1)*cos(e2)*sin(e3) + cos(e1)*cos(e3)*sin(e2))))*(1.0*y6*(sin(e6)*(sin(e2 + e3)*sin(e5) - 1.0*cos(e2 + e3)*cos(e4)*cos(e5)) - 1.0*cos(e2 + e3)*cos(e6)*sin(e4)) - x6*(cos(e6)*(sin(e2 + e3)*sin(e5) - 1.0*cos(e2 + e3)*cos(e4)*cos(e5)) + cos(e2 + e3)*sin(e4)*sin(e6)))) - m6*(1.0*(sin(e5)*(cos(e1)*sin(e4) - 1.0*cos(e4)*(cos(e2)*sin(e1)*sin(e3) + cos(e3)*sin(e1)*sin(e2))) + cos(e5)*(cos(e2)*cos(e3)*sin(e1) - 1.0*sin(e1)*sin(e2)*sin(e3)))*(x6*cos(e6) - 1.0*y6*sin(e6)) + z6*sin(e6)*(sin(e6)*(1.0*cos(e5)*(cos(e1)*sin(e4) - 1.0*cos(e4)*(cos(e2)*sin(e1)*sin(e3) + cos(e3)*sin(e1)*sin(e2))) - sin(e5)*(cos(e2)*cos(e3)*sin(e1) - 1.0*sin(e1)*sin(e2)*sin(e3))) - cos(e6)*(sin(e4)*(cos(e2)*sin(e1)*sin(e3) + cos(e3)*sin(e1)*sin(e2)) + cos(e1)*cos(e4))) + z6*cos(e6)*(cos(e6)*(1.0*cos(e5)*(cos(e1)*sin(e4) - 1.0*cos(e4)*(cos(e2)*sin(e1)*sin(e3) + cos(e3)*sin(e1)*sin(e2))) - sin(e5)*(cos(e2)*cos(e3)*sin(e1) - 1.0*sin(e1)*sin(e2)*sin(e3))) + 1.0*sin(e6)*(sin(e4)*(cos(e2)*sin(e1)*sin(e3) + cos(e3)*sin(e1)*sin(e2)) + cos(e1)*cos(e4))))*((1.0*y6*(sin(e6)*(sin(e2 + e3)*sin(e5) - 1.0*cos(e2 + e3)*cos(e4)*cos(e5)) - 1.0*cos(e2 + e3)*cos(e6)*sin(e4)) - x6*(cos(e6)*(sin(e2 + e3)*sin(e5) - 1.0*cos(e2 + e3)*cos(e4)*cos(e5)) + cos(e2 + e3)*sin(e4)*sin(e6)))*(sin(e5)*(cos(e1)*sin(e4) - 1.0*cos(e4)*(cos(e2)*sin(e1)*sin(e3) + cos(e3)*sin(e1)*sin(e2))) + cos(e5)*(cos(e2)*cos(e3)*sin(e1) - 1.0*sin(e1)*sin(e2)*sin(e3))) - 1.0*(cos(e6)*(1.0*cos(e5)*(cos(e1)*sin(e4) - 1.0*cos(e4)*(cos(e2)*sin(e1)*sin(e3) + cos(e3)*sin(e1)*sin(e2))) - sin(e5)*(cos(e2)*cos(e3)*sin(e1) - 1.0*sin(e1)*sin(e2)*sin(e3))) + 1.0*sin(e6)*(sin(e4)*(cos(e2)*sin(e1)*sin(e3) + cos(e3)*sin(e1)*sin(e2)) + cos(e1)*cos(e4)))*(x6*(sin(e2 + e3)*cos(e5) + cos(e2 + e3)*cos(e4)*sin(e5)) - 1.0*z6*(cos(e6)*(sin(e2 + e3)*sin(e5) - 1.0*cos(e2 + e3)*cos(e4)*cos(e5)) + cos(e2 + e3)*sin(e4)*sin(e6)) + cos(e4)*cos(e6)*(a1 + d4*cos(e2 + e3) + a3*sin(e2 + e3) + a2*sin(e2)) - 1.0*cos(e5)*sin(e4)*sin(e6)*(a1 + d4*cos(e2 + e3) + a3*sin(e2 + e3) + a2*sin(e2))) + (sin(e6)*(1.0*cos(e5)*(cos(e1)*sin(e4) - 1.0*cos(e4)*(cos(e2)*sin(e1)*sin(e3) + cos(e3)*sin(e1)*sin(e2))) - sin(e5)*(cos(e2)*cos(e3)*sin(e1) - 1.0*sin(e1)*sin(e2)*sin(e3))) - cos(e6)*(sin(e4)*(cos(e2)*sin(e1)*sin(e3) + cos(e3)*sin(e1)*sin(e2)) + cos(e1)*cos(e4)))*(z6*(sin(e6)*(sin(e2 + e3)*sin(e5) - 1.0*cos(e2 + e3)*cos(e4)*cos(e5)) - 1.0*cos(e2 + e3)*cos(e6)*sin(e4)) + y6*(sin(e2 + e3)*cos(e5) + cos(e2 + e3)*cos(e4)*sin(e5)) - 1.0*cos(e4)*sin(e6)*(a1 + d4*cos(e2 + e3) + a3*sin(e2 + e3) + a2*sin(e2)) - 1.0*cos(e5)*cos(e6)*sin(e4)*(a1 + d4*cos(e2 + e3) + a3*sin(e2 + e3) + a2*sin(e2))) - 1.0*(cos(e6)*(1.0*cos(e5)*(cos(e1)*sin(e4) - 1.0*cos(e4)*(cos(e2)*sin(e1)*sin(e3) + cos(e3)*sin(e1)*sin(e2))) - sin(e5)*(cos(e2)*cos(e3)*sin(e1) - 1.0*sin(e1)*sin(e2)*sin(e3))) + 1.0*sin(e6)*(sin(e4)*(cos(e2)*sin(e1)*sin(e3) + cos(e3)*sin(e1)*sin(e2)) + cos(e1)*cos(e4)))*(z6*(cos(e6)*(sin(e2 + e3)*sin(e5) - 1.0*cos(e2 + e3)*cos(e4)*cos(e5)) + cos(e2 + e3)*sin(e4)*sin(e6)) - 1.0*cos(e4)*cos(e6)*(a1 + d4*cos(e2 + e3) + a3*sin(e2 + e3) + a2*sin(e2)) + cos(e5)*sin(e4)*sin(e6)*(a1 + d4*cos(e2 + e3) + a3*sin(e2 + e3) + a2*sin(e2))) + (sin(e6)*(1.0*cos(e5)*(cos(e1)*sin(e4) - 1.0*cos(e4)*(cos(e2)*sin(e1)*sin(e3) + cos(e3)*sin(e1)*sin(e2))) - sin(e5)*(cos(e2)*cos(e3)*sin(e1) - 1.0*sin(e1)*sin(e2)*sin(e3))) - cos(e6)*(sin(e4)*(cos(e2)*sin(e1)*sin(e3) + cos(e3)*sin(e1)*sin(e2)) + cos(e1)*cos(e4)))*(cos(e4)*sin(e6)*(a1 + d4*cos(e2 + e3) + a3*sin(e2 + e3) + a2*sin(e2)) - 1.0*z6*(sin(e6)*(sin(e2 + e3)*sin(e5) - 1.0*cos(e2 + e3)*cos(e4)*cos(e5)) - 1.0*cos(e2 + e3)*cos(e6)*sin(e4)) + cos(e5)*cos(e6)*sin(e4)*(a1 + d4*cos(e2 + e3) + a3*sin(e2 + e3) + a2*sin(e2)))) + m6*(z6*sin(e6)*(sin(e6)*(sin(e5)*(cos(e2)*sin(e3) + cos(e3)*sin(e2)) + cos(e4)*cos(e5)*(sin(e2)*sin(e3) - 1.0*cos(e2)*cos(e3))) + cos(e6)*sin(e4)*(sin(e2)*sin(e3) - 1.0*cos(e2)*cos(e3))) - 1.0*(cos(e5)*(cos(e2)*sin(e3) + cos(e3)*sin(e2)) - 1.0*cos(e4)*sin(e5)*(sin(e2)*sin(e3) - 1.0*cos(e2)*cos(e3)))*(x6*cos(e6) - 1.0*y6*sin(e6)) + z6*cos(e6)*(cos(e6)*(sin(e5)*(cos(e2)*sin(e3) + cos(e3)*sin(e2)) + cos(e4)*cos(e5)*(sin(e2)*sin(e3) - 1.0*cos(e2)*cos(e3))) - 1.0*sin(e4)*sin(e6)*(sin(e2)*sin(e3) - 1.0*cos(e2)*cos(e3))))*(1.0*(cos(e6)*(sin(e5)*(cos(e2)*sin(e3) + cos(e3)*sin(e2)) + cos(e4)*cos(e5)*(sin(e2)*sin(e3) - 1.0*cos(e2)*cos(e3))) - 1.0*sin(e4)*sin(e6)*(sin(e2)*sin(e3) - 1.0*cos(e2)*cos(e3)))*(x6*(sin(e2 + e3)*cos(e5) + cos(e2 + e3)*cos(e4)*sin(e5)) - 1.0*z6*(cos(e6)*(sin(e2 + e3)*sin(e5) - 1.0*cos(e2 + e3)*cos(e4)*cos(e5)) + cos(e2 + e3)*sin(e4)*sin(e6)) + cos(e4)*cos(e6)*(a1 + d4*cos(e2 + e3) + a3*sin(e2 + e3) + a2*sin(e2)) - 1.0*cos(e5)*sin(e4)*sin(e6)*(a1 + d4*cos(e2 + e3) + a3*sin(e2 + e3) + a2*sin(e2))) - (sin(e6)*(sin(e5)*(cos(e2)*sin(e3) + cos(e3)*sin(e2)) + cos(e4)*cos(e5)*(sin(e2)*sin(e3) - 1.0*cos(e2)*cos(e3))) + cos(e6)*sin(e4)*(sin(e2)*sin(e3) - 1.0*cos(e2)*cos(e3)))*(z6*(sin(e6)*(sin(e2 + e3)*sin(e5) - 1.0*cos(e2 + e3)*cos(e4)*cos(e5)) - 1.0*cos(e2 + e3)*cos(e6)*sin(e4)) + y6*(sin(e2 + e3)*cos(e5) + cos(e2 + e3)*cos(e4)*sin(e5)) - 1.0*cos(e4)*sin(e6)*(a1 + d4*cos(e2 + e3) + a3*sin(e2 + e3) + a2*sin(e2)) - 1.0*cos(e5)*cos(e6)*sin(e4)*(a1 + d4*cos(e2 + e3) + a3*sin(e2 + e3) + a2*sin(e2))) - (sin(e6)*(sin(e5)*(cos(e2)*sin(e3) + cos(e3)*sin(e2)) + cos(e4)*cos(e5)*(sin(e2)*sin(e3) - 1.0*cos(e2)*cos(e3))) + cos(e6)*sin(e4)*(sin(e2)*sin(e3) - 1.0*cos(e2)*cos(e3)))*(cos(e4)*sin(e6)*(a1 + d4*cos(e2 + e3) + a3*sin(e2 + e3) + a2*sin(e2)) - 1.0*z6*(sin(e6)*(sin(e2 + e3)*sin(e5) - 1.0*cos(e2 + e3)*cos(e4)*cos(e5)) - 1.0*cos(e2 + e3)*cos(e6)*sin(e4)) + cos(e5)*cos(e6)*sin(e4)*(a1 + d4*cos(e2 + e3) + a3*sin(e2 + e3) + a2*sin(e2))) + 1.0*(cos(e6)*(sin(e5)*(cos(e2)*sin(e3) + cos(e3)*sin(e2)) + cos(e4)*cos(e5)*(sin(e2)*sin(e3) - 1.0*cos(e2)*cos(e3))) - 1.0*sin(e4)*sin(e6)*(sin(e2)*sin(e3) - 1.0*cos(e2)*cos(e3)))*(z6*(cos(e6)*(sin(e2 + e3)*sin(e5) - 1.0*cos(e2 + e3)*cos(e4)*cos(e5)) + cos(e2 + e3)*sin(e4)*sin(e6)) - 1.0*cos(e4)*cos(e6)*(a1 + d4*cos(e2 + e3) + a3*sin(e2 + e3) + a2*sin(e2)) + cos(e5)*sin(e4)*sin(e6)*(a1 + d4*cos(e2 + e3) + a3*sin(e2 + e3) + a2*sin(e2))) + (1.0*y6*(sin(e6)*(sin(e2 + e3)*sin(e5) - 1.0*cos(e2 + e3)*cos(e4)*cos(e5)) - 1.0*cos(e2 + e3)*cos(e6)*sin(e4)) - x6*(cos(e6)*(sin(e2 + e3)*sin(e5) - 1.0*cos(e2 + e3)*cos(e4)*cos(e5)) + cos(e2 + e3)*sin(e4)*sin(e6)))*(cos(e5)*(cos(e2)*sin(e3) + cos(e3)*sin(e2)) - 1.0*cos(e4)*sin(e5)*(sin(e2)*sin(e3) - 1.0*cos(e2)*cos(e3)))) + 1.0*m6*(y6*cos(e6) + x6*sin(e6))*(cos(e5)*(cos(e1)*cos(e2)*cos(e3) - 1.0*cos(e1)*sin(e2)*sin(e3)) - 1.0*sin(e5)*(sin(e1)*sin(e4) + cos(e4)*(cos(e1)*cos(e2)*sin(e3) + cos(e1)*cos(e3)*sin(e2))))*((sin(e6)*(sin(e5)*(cos(e1)*cos(e2)*cos(e3) - 1.0*cos(e1)*sin(e2)*sin(e3)) + cos(e5)*(sin(e1)*sin(e4) + cos(e4)*(cos(e1)*cos(e2)*sin(e3) + cos(e1)*cos(e3)*sin(e2)))) - 1.0*cos(e6)*(cos(e4)*sin(e1) - 1.0*sin(e4)*(cos(e1)*cos(e2)*sin(e3) + cos(e1)*cos(e3)*sin(e2))))*(x6*(sin(e2 + e3)*cos(e5) + cos(e2 + e3)*cos(e4)*sin(e5)) - 1.0*z6*(cos(e6)*(sin(e2 + e3)*sin(e5) - 1.0*cos(e2 + e3)*cos(e4)*cos(e5)) + cos(e2 + e3)*sin(e4)*sin(e6)) + cos(e4)*cos(e6)*(a1 + d4*cos(e2 + e3) + a3*sin(e2 + e3) + a2*sin(e2)) - 1.0*cos(e5)*sin(e4)*sin(e6)*(a1 + d4*cos(e2 + e3) + a3*sin(e2 + e3) + a2*sin(e2))) + (sin(e6)*(cos(e4)*sin(e1) - 1.0*sin(e4)*(cos(e1)*cos(e2)*sin(e3) + cos(e1)*cos(e3)*sin(e2))) + cos(e6)*(sin(e5)*(cos(e1)*cos(e2)*cos(e3) - 1.0*cos(e1)*sin(e2)*sin(e3)) + cos(e5)*(sin(e1)*sin(e4) + cos(e4)*(cos(e1)*cos(e2)*sin(e3) + cos(e1)*cos(e3)*sin(e2)))))*(z6*(sin(e6)*(sin(e2 + e3)*sin(e5) - 1.0*cos(e2 + e3)*cos(e4)*cos(e5)) - 1.0*cos(e2 + e3)*cos(e6)*sin(e4)) + y6*(sin(e2 + e3)*cos(e5) + cos(e2 + e3)*cos(e4)*sin(e5)) - 1.0*cos(e4)*sin(e6)*(a1 + d4*cos(e2 + e3) + a3*sin(e2 + e3) + a2*sin(e2)) - 1.0*cos(e5)*cos(e6)*sin(e4)*(a1 + d4*cos(e2 + e3) + a3*sin(e2 + e3) + a2*sin(e2))) - 1.0*(cos(e5)*(cos(e1)*cos(e2)*cos(e3) - 1.0*cos(e1)*sin(e2)*sin(e3)) - 1.0*sin(e5)*(sin(e1)*sin(e4) + cos(e4)*(cos(e1)*cos(e2)*sin(e3) + cos(e1)*cos(e3)*sin(e2))))*(x6*(sin(e6)*(sin(e2 + e3)*sin(e5) - 1.0*cos(e2 + e3)*cos(e4)*cos(e5)) - 1.0*cos(e2 + e3)*cos(e6)*sin(e4)) + y6*(cos(e6)*(sin(e2 + e3)*sin(e5) - 1.0*cos(e2 + e3)*cos(e4)*cos(e5)) + cos(e2 + e3)*sin(e4)*sin(e6)) - 1.0*sin(e4)*sin(e5)*(a1 + d4*cos(e2 + e3) + a3*sin(e2 + e3) + a2*sin(e2)))) - 1.0*m6*(y6*cos(e6) + x6*sin(e6))*(sin(e5)*(cos(e1)*sin(e4) - 1.0*cos(e4)*(cos(e2)*sin(e1)*sin(e3) + cos(e3)*sin(e1)*sin(e2))) + cos(e5)*(cos(e2)*cos(e3)*sin(e1) - 1.0*sin(e1)*sin(e2)*sin(e3)))*((sin(e6)*(1.0*cos(e5)*(cos(e1)*sin(e4) - 1.0*cos(e4)*(cos(e2)*sin(e1)*sin(e3) + cos(e3)*sin(e1)*sin(e2))) - sin(e5)*(cos(e2)*cos(e3)*sin(e1) - 1.0*sin(e1)*sin(e2)*sin(e3))) - cos(e6)*(sin(e4)*(cos(e2)*sin(e1)*sin(e3) + cos(e3)*sin(e1)*sin(e2)) + cos(e1)*cos(e4)))*(x6*(sin(e2 + e3)*cos(e5) + cos(e2 + e3)*cos(e4)*sin(e5)) - 1.0*z6*(cos(e6)*(sin(e2 + e3)*sin(e5) - 1.0*cos(e2 + e3)*cos(e4)*cos(e5)) + cos(e2 + e3)*sin(e4)*sin(e6)) + cos(e4)*cos(e6)*(a1 + d4*cos(e2 + e3) + a3*sin(e2 + e3) + a2*sin(e2)) - 1.0*cos(e5)*sin(e4)*sin(e6)*(a1 + d4*cos(e2 + e3) + a3*sin(e2 + e3) + a2*sin(e2))) + 1.0*(sin(e5)*(cos(e1)*sin(e4) - 1.0*cos(e4)*(cos(e2)*sin(e1)*sin(e3) + cos(e3)*sin(e1)*sin(e2))) + cos(e5)*(cos(e2)*cos(e3)*sin(e1) - 1.0*sin(e1)*sin(e2)*sin(e3)))*(x6*(sin(e6)*(sin(e2 + e3)*sin(e5) - 1.0*cos(e2 + e3)*cos(e4)*cos(e5)) - 1.0*cos(e2 + e3)*cos(e6)*sin(e4)) + y6*(cos(e6)*(sin(e2 + e3)*sin(e5) - 1.0*cos(e2 + e3)*cos(e4)*cos(e5)) + cos(e2 + e3)*sin(e4)*sin(e6)) - 1.0*sin(e4)*sin(e5)*(a1 + d4*cos(e2 + e3) + a3*sin(e2 + e3) + a2*sin(e2))) + (cos(e6)*(1.0*cos(e5)*(cos(e1)*sin(e4) - 1.0*cos(e4)*(cos(e2)*sin(e1)*sin(e3) + cos(e3)*sin(e1)*sin(e2))) - sin(e5)*(cos(e2)*cos(e3)*sin(e1) - 1.0*sin(e1)*sin(e2)*sin(e3))) + 1.0*sin(e6)*(sin(e4)*(cos(e2)*sin(e1)*sin(e3) + cos(e3)*sin(e1)*sin(e2)) + cos(e1)*cos(e4)))*(z6*(sin(e6)*(sin(e2 + e3)*sin(e5) - 1.0*cos(e2 + e3)*cos(e4)*cos(e5)) - 1.0*cos(e2 + e3)*cos(e6)*sin(e4)) + y6*(sin(e2 + e3)*cos(e5) + cos(e2 + e3)*cos(e4)*sin(e5)) - 1.0*cos(e4)*sin(e6)*(a1 + d4*cos(e2 + e3) + a3*sin(e2 + e3) + a2*sin(e2)) - 1.0*cos(e5)*cos(e6)*sin(e4)*(a1 + d4*cos(e2 + e3) + a3*sin(e2 + e3) + a2*sin(e2)))) + 1.0*m6*(y6*cos(e6) + x6*sin(e6))*(cos(e5)*(cos(e2)*sin(e3) + cos(e3)*sin(e2)) - 1.0*cos(e4)*sin(e5)*(sin(e2)*sin(e3) - 1.0*cos(e2)*cos(e3)))*((sin(e6)*(sin(e5)*(cos(e2)*sin(e3) + cos(e3)*sin(e2)) + cos(e4)*cos(e5)*(sin(e2)*sin(e3) - 1.0*cos(e2)*cos(e3))) + cos(e6)*sin(e4)*(sin(e2)*sin(e3) - 1.0*cos(e2)*cos(e3)))*(x6*(sin(e2 + e3)*cos(e5) + cos(e2 + e3)*cos(e4)*sin(e5)) - 1.0*z6*(cos(e6)*(sin(e2 + e3)*sin(e5) - 1.0*cos(e2 + e3)*cos(e4)*cos(e5)) + cos(e2 + e3)*sin(e4)*sin(e6)) + cos(e4)*cos(e6)*(a1 + d4*cos(e2 + e3) + a3*sin(e2 + e3) + a2*sin(e2)) - 1.0*cos(e5)*sin(e4)*sin(e6)*(a1 + d4*cos(e2 + e3) + a3*sin(e2 + e3) + a2*sin(e2))) + (cos(e6)*(sin(e5)*(cos(e2)*sin(e3) + cos(e3)*sin(e2)) + cos(e4)*cos(e5)*(sin(e2)*sin(e3) - 1.0*cos(e2)*cos(e3))) - 1.0*sin(e4)*sin(e6)*(sin(e2)*sin(e3) - 1.0*cos(e2)*cos(e3)))*(z6*(sin(e6)*(sin(e2 + e3)*sin(e5) - 1.0*cos(e2 + e3)*cos(e4)*cos(e5)) - 1.0*cos(e2 + e3)*cos(e6)*sin(e4)) + y6*(sin(e2 + e3)*cos(e5) + cos(e2 + e3)*cos(e4)*sin(e5)) - 1.0*cos(e4)*sin(e6)*(a1 + d4*cos(e2 + e3) + a3*sin(e2 + e3) + a2*sin(e2)) - 1.0*cos(e5)*cos(e6)*sin(e4)*(a1 + d4*cos(e2 + e3) + a3*sin(e2 + e3) + a2*sin(e2))) - 1.0*(cos(e5)*(cos(e2)*sin(e3) + cos(e3)*sin(e2)) - 1.0*cos(e4)*sin(e5)*(sin(e2)*sin(e3) - 1.0*cos(e2)*cos(e3)))*(x6*(sin(e6)*(sin(e2 + e3)*sin(e5) - 1.0*cos(e2 + e3)*cos(e4)*cos(e5)) - 1.0*cos(e2 + e3)*cos(e6)*sin(e4)) + y6*(cos(e6)*(sin(e2 + e3)*sin(e5) - 1.0*cos(e2 + e3)*cos(e4)*cos(e5)) + cos(e2 + e3)*sin(e4)*sin(e6)) - 1.0*sin(e4)*sin(e5)*(a1 + d4*cos(e2 + e3) + a3*sin(e2 + e3) + a2*sin(e2))))))/2 + de6*((I6xz*(sin(e6)*(sin(e2 + e3)*sin(e5) - cos(e2 + e3)*cos(e4)*cos(e5)) - cos(e2 + e3)*cos(e6)*sin(e4)))/2 + (I6yz*(cos(e6)*(sin(e2 + e3)*sin(e5) - cos(e2 + e3)*cos(e4)*cos(e5)) + cos(e2 + e3)*sin(e4)*sin(e6)))/2 + (I6zx*(sin(e6)*(sin(e2 + e3)*sin(e5) - cos(e2 + e3)*cos(e4)*cos(e5)) - cos(e2 + e3)*cos(e6)*sin(e4)))/2 + (I6zy*(cos(e6)*(sin(e2 + e3)*sin(e5) - cos(e2 + e3)*cos(e4)*cos(e5)) + cos(e2 + e3)*sin(e4)*sin(e6)))/2 + m6*(x6*(sin(e6)*(sin(e5)*(cos(e2)*sin(e3) + cos(e3)*sin(e2)) + cos(e4)*cos(e5)*(sin(e2)*sin(e3) - cos(e2)*cos(e3))) + cos(e6)*sin(e4)*(sin(e2)*sin(e3) - cos(e2)*cos(e3))) + y6*(cos(e6)*(sin(e5)*(cos(e2)*sin(e3) + cos(e3)*sin(e2)) + cos(e4)*cos(e5)*(sin(e2)*sin(e3) - cos(e2)*cos(e3))) - sin(e4)*sin(e6)*(sin(e2)*sin(e3) - cos(e2)*cos(e3))))*((sin(e6)*(sin(e5)*(cos(e2)*sin(e3) + cos(e3)*sin(e2)) + cos(e4)*cos(e5)*(sin(e2)*sin(e3) - cos(e2)*cos(e3))) + cos(e6)*sin(e4)*(sin(e2)*sin(e3) - cos(e2)*cos(e3)))*(y6*(sin(e2 + e3)*cos(e5) + cos(e2 + e3)*cos(e4)*sin(e5)) + z6*(sin(e6)*(sin(e2 + e3)*sin(e5) - cos(e2 + e3)*cos(e4)*cos(e5)) - cos(e2 + e3)*cos(e6)*sin(e4)) - cos(e4)*sin(e6)*(a1 + d4*cos(e2 + e3) + a3*sin(e2 + e3) + a2*sin(e2)) - cos(e5)*cos(e6)*sin(e4)*(a1 + d4*cos(e2 + e3) + a3*sin(e2 + e3) + a2*sin(e2))) - (cos(e6)*(sin(e5)*(cos(e2)*sin(e3) + cos(e3)*sin(e2)) + cos(e4)*cos(e5)*(sin(e2)*sin(e3) - cos(e2)*cos(e3))) - sin(e4)*sin(e6)*(sin(e2)*sin(e3) - cos(e2)*cos(e3)))*(x6*(sin(e2 + e3)*cos(e5) + cos(e2 + e3)*cos(e4)*sin(e5)) - z6*(cos(e6)*(sin(e2 + e3)*sin(e5) - cos(e2 + e3)*cos(e4)*cos(e5)) + cos(e2 + e3)*sin(e4)*sin(e6)) + cos(e4)*cos(e6)*(a1 + d4*cos(e2 + e3) + a3*sin(e2 + e3) + a2*sin(e2)) - cos(e5)*sin(e4)*sin(e6)*(a1 + d4*cos(e2 + e3) + a3*sin(e2 + e3) + a2*sin(e2))) + (cos(e5)*(cos(e2)*sin(e3) + cos(e3)*sin(e2)) - cos(e4)*sin(e5)*(sin(e2)*sin(e3) - cos(e2)*cos(e3)))*(x6*(cos(e6)*(sin(e2 + e3)*sin(e5) - cos(e2 + e3)*cos(e4)*cos(e5)) + cos(e2 + e3)*sin(e4)*sin(e6)) - y6*(sin(e6)*(sin(e2 + e3)*sin(e5) - cos(e2 + e3)*cos(e4)*cos(e5)) - cos(e2 + e3)*cos(e6)*sin(e4))) + (sin(e6)*(sin(e5)*(cos(e2)*sin(e3) + cos(e3)*sin(e2)) + cos(e4)*cos(e5)*(sin(e2)*sin(e3) - cos(e2)*cos(e3))) + cos(e6)*sin(e4)*(sin(e2)*sin(e3) - cos(e2)*cos(e3)))*(cos(e4)*sin(e6)*(a1 + d4*cos(e2 + e3) + a3*sin(e2 + e3) + a2*sin(e2)) - z6*(sin(e6)*(sin(e2 + e3)*sin(e5) - cos(e2 + e3)*cos(e4)*cos(e5)) - cos(e2 + e3)*cos(e6)*sin(e4)) + cos(e5)*cos(e6)*sin(e4)*(a1 + d4*cos(e2 + e3) + a3*sin(e2 + e3) + a2*sin(e2))) - (cos(e6)*(sin(e5)*(cos(e2)*sin(e3) + cos(e3)*sin(e2)) + cos(e4)*cos(e5)*(sin(e2)*sin(e3) - cos(e2)*cos(e3))) - sin(e4)*sin(e6)*(sin(e2)*sin(e3) - cos(e2)*cos(e3)))*(z6*(cos(e6)*(sin(e2 + e3)*sin(e5) - cos(e2 + e3)*cos(e4)*cos(e5)) + cos(e2 + e3)*sin(e4)*sin(e6)) - cos(e4)*cos(e6)*(a1 + d4*cos(e2 + e3) + a3*sin(e2 + e3) + a2*sin(e2)) + cos(e5)*sin(e4)*sin(e6)*(a1 + d4*cos(e2 + e3) + a3*sin(e2 + e3) + a2*sin(e2)))) - m6*(x6*(cos(e6)*(sin(e5)*(cos(e1)*cos(e2)*cos(e3) - cos(e1)*sin(e2)*sin(e3)) + cos(e5)*(sin(e1)*sin(e4) + cos(e4)*(cos(e1)*cos(e2)*sin(e3) + cos(e1)*cos(e3)*sin(e2)))) + sin(e6)*(cos(e4)*sin(e1) - sin(e4)*(cos(e1)*cos(e2)*sin(e3) + cos(e1)*cos(e3)*sin(e2)))) - y6*(sin(e6)*(sin(e5)*(cos(e1)*cos(e2)*cos(e3) - cos(e1)*sin(e2)*sin(e3)) + cos(e5)*(sin(e1)*sin(e4) + cos(e4)*(cos(e1)*cos(e2)*sin(e3) + cos(e1)*cos(e3)*sin(e2)))) - cos(e6)*(cos(e4)*sin(e1) - sin(e4)*(cos(e1)*cos(e2)*sin(e3) + cos(e1)*cos(e3)*sin(e2)))))*((sin(e6)*(sin(e5)*(cos(e1)*cos(e2)*cos(e3) - cos(e1)*sin(e2)*sin(e3)) + cos(e5)*(sin(e1)*sin(e4) + cos(e4)*(cos(e1)*cos(e2)*sin(e3) + cos(e1)*cos(e3)*sin(e2)))) - cos(e6)*(cos(e4)*sin(e1) - sin(e4)*(cos(e1)*cos(e2)*sin(e3) + cos(e1)*cos(e3)*sin(e2))))*(x6*(sin(e2 + e3)*cos(e5) + cos(e2 + e3)*cos(e4)*sin(e5)) - z6*(cos(e6)*(sin(e2 + e3)*sin(e5) - cos(e2 + e3)*cos(e4)*cos(e5)) + cos(e2 + e3)*sin(e4)*sin(e6)) + cos(e4)*cos(e6)*(a1 + d4*cos(e2 + e3) + a3*sin(e2 + e3) + a2*sin(e2)) - cos(e5)*sin(e4)*sin(e6)*(a1 + d4*cos(e2 + e3) + a3*sin(e2 + e3) + a2*sin(e2))) + (cos(e6)*(sin(e5)*(cos(e1)*cos(e2)*cos(e3) - cos(e1)*sin(e2)*sin(e3)) + cos(e5)*(sin(e1)*sin(e4) + cos(e4)*(cos(e1)*cos(e2)*sin(e3) + cos(e1)*cos(e3)*sin(e2)))) + sin(e6)*(cos(e4)*sin(e1) - sin(e4)*(cos(e1)*cos(e2)*sin(e3) + cos(e1)*cos(e3)*sin(e2))))*(y6*(sin(e2 + e3)*cos(e5) + cos(e2 + e3)*cos(e4)*sin(e5)) + z6*(sin(e6)*(sin(e2 + e3)*sin(e5) - cos(e2 + e3)*cos(e4)*cos(e5)) - cos(e2 + e3)*cos(e6)*sin(e4)) - cos(e4)*sin(e6)*(a1 + d4*cos(e2 + e3) + a3*sin(e2 + e3) + a2*sin(e2)) - cos(e5)*cos(e6)*sin(e4)*(a1 + d4*cos(e2 + e3) + a3*sin(e2 + e3) + a2*sin(e2))) - (cos(e5)*(cos(e1)*cos(e2)*cos(e3) - cos(e1)*sin(e2)*sin(e3)) - sin(e5)*(sin(e1)*sin(e4) + cos(e4)*(cos(e1)*cos(e2)*sin(e3) + cos(e1)*cos(e3)*sin(e2))))*(x6*(sin(e6)*(sin(e2 + e3)*sin(e5) - cos(e2 + e3)*cos(e4)*cos(e5)) - cos(e2 + e3)*cos(e6)*sin(e4)) + y6*(cos(e6)*(sin(e2 + e3)*sin(e5) - cos(e2 + e3)*cos(e4)*cos(e5)) + cos(e2 + e3)*sin(e4)*sin(e6)) - sin(e4)*sin(e5)*(a1 + d4*cos(e2 + e3) + a3*sin(e2 + e3) + a2*sin(e2)))) - m6*(x6*(cos(e6)*(sin(e5)*(cos(e2)*sin(e3) + cos(e3)*sin(e2)) + cos(e4)*cos(e5)*(sin(e2)*sin(e3) - cos(e2)*cos(e3))) - sin(e4)*sin(e6)*(sin(e2)*sin(e3) - cos(e2)*cos(e3))) - y6*(sin(e6)*(sin(e5)*(cos(e2)*sin(e3) + cos(e3)*sin(e2)) + cos(e4)*cos(e5)*(sin(e2)*sin(e3) - cos(e2)*cos(e3))) + cos(e6)*sin(e4)*(sin(e2)*sin(e3) - cos(e2)*cos(e3))))*((sin(e6)*(sin(e5)*(cos(e2)*sin(e3) + cos(e3)*sin(e2)) + cos(e4)*cos(e5)*(sin(e2)*sin(e3) - cos(e2)*cos(e3))) + cos(e6)*sin(e4)*(sin(e2)*sin(e3) - cos(e2)*cos(e3)))*(x6*(sin(e2 + e3)*cos(e5) + cos(e2 + e3)*cos(e4)*sin(e5)) - z6*(cos(e6)*(sin(e2 + e3)*sin(e5) - cos(e2 + e3)*cos(e4)*cos(e5)) + cos(e2 + e3)*sin(e4)*sin(e6)) + cos(e4)*cos(e6)*(a1 + d4*cos(e2 + e3) + a3*sin(e2 + e3) + a2*sin(e2)) - cos(e5)*sin(e4)*sin(e6)*(a1 + d4*cos(e2 + e3) + a3*sin(e2 + e3) + a2*sin(e2))) + (cos(e6)*(sin(e5)*(cos(e2)*sin(e3) + cos(e3)*sin(e2)) + cos(e4)*cos(e5)*(sin(e2)*sin(e3) - cos(e2)*cos(e3))) - sin(e4)*sin(e6)*(sin(e2)*sin(e3) - cos(e2)*cos(e3)))*(y6*(sin(e2 + e3)*cos(e5) + cos(e2 + e3)*cos(e4)*sin(e5)) + z6*(sin(e6)*(sin(e2 + e3)*sin(e5) - cos(e2 + e3)*cos(e4)*cos(e5)) - cos(e2 + e3)*cos(e6)*sin(e4)) - cos(e4)*sin(e6)*(a1 + d4*cos(e2 + e3) + a3*sin(e2 + e3) + a2*sin(e2)) - cos(e5)*cos(e6)*sin(e4)*(a1 + d4*cos(e2 + e3) + a3*sin(e2 + e3) + a2*sin(e2))) - (cos(e5)*(cos(e2)*sin(e3) + cos(e3)*sin(e2)) - cos(e4)*sin(e5)*(sin(e2)*sin(e3) - cos(e2)*cos(e3)))*(x6*(sin(e6)*(sin(e2 + e3)*sin(e5) - cos(e2 + e3)*cos(e4)*cos(e5)) - cos(e2 + e3)*cos(e6)*sin(e4)) + y6*(cos(e6)*(sin(e2 + e3)*sin(e5) - cos(e2 + e3)*cos(e4)*cos(e5)) + cos(e2 + e3)*sin(e4)*sin(e6)) - sin(e4)*sin(e5)*(a1 + d4*cos(e2 + e3) + a3*sin(e2 + e3) + a2*sin(e2)))) + m6*(x6*(sin(e6)*(sin(e5)*(cos(e2)*cos(e3)*sin(e1) - sin(e1)*sin(e2)*sin(e3)) - cos(e5)*(cos(e1)*sin(e4) - cos(e4)*(cos(e2)*sin(e1)*sin(e3) + cos(e3)*sin(e1)*sin(e2)))) + cos(e6)*(sin(e4)*(cos(e2)*sin(e1)*sin(e3) + cos(e3)*sin(e1)*sin(e2)) + cos(e1)*cos(e4))) + y6*(cos(e6)*(sin(e5)*(cos(e2)*cos(e3)*sin(e1) - sin(e1)*sin(e2)*sin(e3)) - cos(e5)*(cos(e1)*sin(e4) - cos(e4)*(cos(e2)*sin(e1)*sin(e3) + cos(e3)*sin(e1)*sin(e2)))) - sin(e6)*(sin(e4)*(cos(e2)*sin(e1)*sin(e3) + cos(e3)*sin(e1)*sin(e2)) + cos(e1)*cos(e4))))*((sin(e6)*(sin(e5)*(cos(e2)*cos(e3)*sin(e1) - sin(e1)*sin(e2)*sin(e3)) - cos(e5)*(cos(e1)*sin(e4) - cos(e4)*(cos(e2)*sin(e1)*sin(e3) + cos(e3)*sin(e1)*sin(e2)))) + cos(e6)*(sin(e4)*(cos(e2)*sin(e1)*sin(e3) + cos(e3)*sin(e1)*sin(e2)) + cos(e1)*cos(e4)))*(cos(e4)*sin(e6)*(a1 + d4*cos(e2 + e3) + a3*sin(e2 + e3) + a2*sin(e2)) - z6*(sin(e6)*(sin(e2 + e3)*sin(e5) - cos(e2 + e3)*cos(e4)*cos(e5)) - cos(e2 + e3)*cos(e6)*sin(e4)) + cos(e5)*cos(e6)*sin(e4)*(a1 + d4*cos(e2 + e3) + a3*sin(e2 + e3) + a2*sin(e2))) - (cos(e6)*(sin(e5)*(cos(e2)*cos(e3)*sin(e1) - sin(e1)*sin(e2)*sin(e3)) - cos(e5)*(cos(e1)*sin(e4) - cos(e4)*(cos(e2)*sin(e1)*sin(e3) + cos(e3)*sin(e1)*sin(e2)))) - sin(e6)*(sin(e4)*(cos(e2)*sin(e1)*sin(e3) + cos(e3)*sin(e1)*sin(e2)) + cos(e1)*cos(e4)))*(z6*(cos(e6)*(sin(e2 + e3)*sin(e5) - cos(e2 + e3)*cos(e4)*cos(e5)) + cos(e2 + e3)*sin(e4)*sin(e6)) - cos(e4)*cos(e6)*(a1 + d4*cos(e2 + e3) + a3*sin(e2 + e3) + a2*sin(e2)) + cos(e5)*sin(e4)*sin(e6)*(a1 + d4*cos(e2 + e3) + a3*sin(e2 + e3) + a2*sin(e2))) + (cos(e5)*(cos(e2)*cos(e3)*sin(e1) - sin(e1)*sin(e2)*sin(e3)) + sin(e5)*(cos(e1)*sin(e4) - cos(e4)*(cos(e2)*sin(e1)*sin(e3) + cos(e3)*sin(e1)*sin(e2))))*(x6*(cos(e6)*(sin(e2 + e3)*sin(e5) - cos(e2 + e3)*cos(e4)*cos(e5)) + cos(e2 + e3)*sin(e4)*sin(e6)) - y6*(sin(e6)*(sin(e2 + e3)*sin(e5) - cos(e2 + e3)*cos(e4)*cos(e5)) - cos(e2 + e3)*cos(e6)*sin(e4))) - (cos(e6)*(sin(e5)*(cos(e2)*cos(e3)*sin(e1) - sin(e1)*sin(e2)*sin(e3)) - cos(e5)*(cos(e1)*sin(e4) - cos(e4)*(cos(e2)*sin(e1)*sin(e3) + cos(e3)*sin(e1)*sin(e2)))) - sin(e6)*(sin(e4)*(cos(e2)*sin(e1)*sin(e3) + cos(e3)*sin(e1)*sin(e2)) + cos(e1)*cos(e4)))*(x6*(sin(e2 + e3)*cos(e5) + cos(e2 + e3)*cos(e4)*sin(e5)) - z6*(cos(e6)*(sin(e2 + e3)*sin(e5) - cos(e2 + e3)*cos(e4)*cos(e5)) + cos(e2 + e3)*sin(e4)*sin(e6)) + cos(e4)*cos(e6)*(a1 + d4*cos(e2 + e3) + a3*sin(e2 + e3) + a2*sin(e2)) - cos(e5)*sin(e4)*sin(e6)*(a1 + d4*cos(e2 + e3) + a3*sin(e2 + e3) + a2*sin(e2))) + (sin(e6)*(sin(e5)*(cos(e2)*cos(e3)*sin(e1) - sin(e1)*sin(e2)*sin(e3)) - cos(e5)*(cos(e1)*sin(e4) - cos(e4)*(cos(e2)*sin(e1)*sin(e3) + cos(e3)*sin(e1)*sin(e2)))) + cos(e6)*(sin(e4)*(cos(e2)*sin(e1)*sin(e3) + cos(e3)*sin(e1)*sin(e2)) + cos(e1)*cos(e4)))*(y6*(sin(e2 + e3)*cos(e5) + cos(e2 + e3)*cos(e4)*sin(e5)) + z6*(sin(e6)*(sin(e2 + e3)*sin(e5) - cos(e2 + e3)*cos(e4)*cos(e5)) - cos(e2 + e3)*cos(e6)*sin(e4)) - cos(e4)*sin(e6)*(a1 + d4*cos(e2 + e3) + a3*sin(e2 + e3) + a2*sin(e2)) - cos(e5)*cos(e6)*sin(e4)*(a1 + d4*cos(e2 + e3) + a3*sin(e2 + e3) + a2*sin(e2)))) - m6*(x6*(cos(e6)*(sin(e5)*(cos(e2)*cos(e3)*sin(e1) - sin(e1)*sin(e2)*sin(e3)) - cos(e5)*(cos(e1)*sin(e4) - cos(e4)*(cos(e2)*sin(e1)*sin(e3) + cos(e3)*sin(e1)*sin(e2)))) - sin(e6)*(sin(e4)*(cos(e2)*sin(e1)*sin(e3) + cos(e3)*sin(e1)*sin(e2)) + cos(e1)*cos(e4))) - y6*(sin(e6)*(sin(e5)*(cos(e2)*cos(e3)*sin(e1) - sin(e1)*sin(e2)*sin(e3)) - cos(e5)*(cos(e1)*sin(e4) - cos(e4)*(cos(e2)*sin(e1)*sin(e3) + cos(e3)*sin(e1)*sin(e2)))) + cos(e6)*(sin(e4)*(cos(e2)*sin(e1)*sin(e3) + cos(e3)*sin(e1)*sin(e2)) + cos(e1)*cos(e4))))*((sin(e6)*(sin(e5)*(cos(e2)*cos(e3)*sin(e1) - sin(e1)*sin(e2)*sin(e3)) - cos(e5)*(cos(e1)*sin(e4) - cos(e4)*(cos(e2)*sin(e1)*sin(e3) + cos(e3)*sin(e1)*sin(e2)))) + cos(e6)*(sin(e4)*(cos(e2)*sin(e1)*sin(e3) + cos(e3)*sin(e1)*sin(e2)) + cos(e1)*cos(e4)))*(x6*(sin(e2 + e3)*cos(e5) + cos(e2 + e3)*cos(e4)*sin(e5)) - z6*(cos(e6)*(sin(e2 + e3)*sin(e5) - cos(e2 + e3)*cos(e4)*cos(e5)) + cos(e2 + e3)*sin(e4)*sin(e6)) + cos(e4)*cos(e6)*(a1 + d4*cos(e2 + e3) + a3*sin(e2 + e3) + a2*sin(e2)) - cos(e5)*sin(e4)*sin(e6)*(a1 + d4*cos(e2 + e3) + a3*sin(e2 + e3) + a2*sin(e2))) + (cos(e6)*(sin(e5)*(cos(e2)*cos(e3)*sin(e1) - sin(e1)*sin(e2)*sin(e3)) - cos(e5)*(cos(e1)*sin(e4) - cos(e4)*(cos(e2)*sin(e1)*sin(e3) + cos(e3)*sin(e1)*sin(e2)))) - sin(e6)*(sin(e4)*(cos(e2)*sin(e1)*sin(e3) + cos(e3)*sin(e1)*sin(e2)) + cos(e1)*cos(e4)))*(y6*(sin(e2 + e3)*cos(e5) + cos(e2 + e3)*cos(e4)*sin(e5)) + z6*(sin(e6)*(sin(e2 + e3)*sin(e5) - cos(e2 + e3)*cos(e4)*cos(e5)) - cos(e2 + e3)*cos(e6)*sin(e4)) - cos(e4)*sin(e6)*(a1 + d4*cos(e2 + e3) + a3*sin(e2 + e3) + a2*sin(e2)) - cos(e5)*cos(e6)*sin(e4)*(a1 + d4*cos(e2 + e3) + a3*sin(e2 + e3) + a2*sin(e2))) - (cos(e5)*(cos(e2)*cos(e3)*sin(e1) - sin(e1)*sin(e2)*sin(e3)) + sin(e5)*(cos(e1)*sin(e4) - cos(e4)*(cos(e2)*sin(e1)*sin(e3) + cos(e3)*sin(e1)*sin(e2))))*(x6*(sin(e6)*(sin(e2 + e3)*sin(e5) - cos(e2 + e3)*cos(e4)*cos(e5)) - cos(e2 + e3)*cos(e6)*sin(e4)) + y6*(cos(e6)*(sin(e2 + e3)*sin(e5) - cos(e2 + e3)*cos(e4)*cos(e5)) + cos(e2 + e3)*sin(e4)*sin(e6)) - sin(e4)*sin(e5)*(a1 + d4*cos(e2 + e3) + a3*sin(e2 + e3) + a2*sin(e2)))) + m6*(x6*(sin(e6)*(sin(e5)*(cos(e1)*cos(e2)*cos(e3) - cos(e1)*sin(e2)*sin(e3)) + cos(e5)*(sin(e1)*sin(e4) + cos(e4)*(cos(e1)*cos(e2)*sin(e3) + cos(e1)*cos(e3)*sin(e2)))) - cos(e6)*(cos(e4)*sin(e1) - sin(e4)*(cos(e1)*cos(e2)*sin(e3) + cos(e1)*cos(e3)*sin(e2)))) + y6*(cos(e6)*(sin(e5)*(cos(e1)*cos(e2)*cos(e3) - cos(e1)*sin(e2)*sin(e3)) + cos(e5)*(sin(e1)*sin(e4) + cos(e4)*(cos(e1)*cos(e2)*sin(e3) + cos(e1)*cos(e3)*sin(e2)))) + sin(e6)*(cos(e4)*sin(e1) - sin(e4)*(cos(e1)*cos(e2)*sin(e3) + cos(e1)*cos(e3)*sin(e2)))))*((sin(e6)*(sin(e5)*(cos(e1)*cos(e2)*cos(e3) - cos(e1)*sin(e2)*sin(e3)) + cos(e5)*(sin(e1)*sin(e4) + cos(e4)*(cos(e1)*cos(e2)*sin(e3) + cos(e1)*cos(e3)*sin(e2)))) - cos(e6)*(cos(e4)*sin(e1) - sin(e4)*(cos(e1)*cos(e2)*sin(e3) + cos(e1)*cos(e3)*sin(e2))))*(y6*(sin(e2 + e3)*cos(e5) + cos(e2 + e3)*cos(e4)*sin(e5)) + z6*(sin(e6)*(sin(e2 + e3)*sin(e5) - cos(e2 + e3)*cos(e4)*cos(e5)) - cos(e2 + e3)*cos(e6)*sin(e4)) - cos(e4)*sin(e6)*(a1 + d4*cos(e2 + e3) + a3*sin(e2 + e3) + a2*sin(e2)) - cos(e5)*cos(e6)*sin(e4)*(a1 + d4*cos(e2 + e3) + a3*sin(e2 + e3) + a2*sin(e2))) - (cos(e6)*(sin(e5)*(cos(e1)*cos(e2)*cos(e3) - cos(e1)*sin(e2)*sin(e3)) + cos(e5)*(sin(e1)*sin(e4) + cos(e4)*(cos(e1)*cos(e2)*sin(e3) + cos(e1)*cos(e3)*sin(e2)))) + sin(e6)*(cos(e4)*sin(e1) - sin(e4)*(cos(e1)*cos(e2)*sin(e3) + cos(e1)*cos(e3)*sin(e2))))*(x6*(sin(e2 + e3)*cos(e5) + cos(e2 + e3)*cos(e4)*sin(e5)) - z6*(cos(e6)*(sin(e2 + e3)*sin(e5) - cos(e2 + e3)*cos(e4)*cos(e5)) + cos(e2 + e3)*sin(e4)*sin(e6)) + cos(e4)*cos(e6)*(a1 + d4*cos(e2 + e3) + a3*sin(e2 + e3) + a2*sin(e2)) - cos(e5)*sin(e4)*sin(e6)*(a1 + d4*cos(e2 + e3) + a3*sin(e2 + e3) + a2*sin(e2))) + (cos(e5)*(cos(e1)*cos(e2)*cos(e3) - cos(e1)*sin(e2)*sin(e3)) - sin(e5)*(sin(e1)*sin(e4) + cos(e4)*(cos(e1)*cos(e2)*sin(e3) + cos(e1)*cos(e3)*sin(e2))))*(x6*(cos(e6)*(sin(e2 + e3)*sin(e5) - cos(e2 + e3)*cos(e4)*cos(e5)) + cos(e2 + e3)*sin(e4)*sin(e6)) - y6*(sin(e6)*(sin(e2 + e3)*sin(e5) - cos(e2 + e3)*cos(e4)*cos(e5)) - cos(e2 + e3)*cos(e6)*sin(e4))) - (cos(e6)*(sin(e5)*(cos(e1)*cos(e2)*cos(e3) - cos(e1)*sin(e2)*sin(e3)) + cos(e5)*(sin(e1)*sin(e4) + cos(e4)*(cos(e1)*cos(e2)*sin(e3) + cos(e1)*cos(e3)*sin(e2)))) + sin(e6)*(cos(e4)*sin(e1) - sin(e4)*(cos(e1)*cos(e2)*sin(e3) + cos(e1)*cos(e3)*sin(e2))))*(z6*(cos(e6)*(sin(e2 + e3)*sin(e5) - cos(e2 + e3)*cos(e4)*cos(e5)) + cos(e2 + e3)*sin(e4)*sin(e6)) - cos(e4)*cos(e6)*(a1 + d4*cos(e2 + e3) + a3*sin(e2 + e3) + a2*sin(e2)) + cos(e5)*sin(e4)*sin(e6)*(a1 + d4*cos(e2 + e3) + a3*sin(e2 + e3) + a2*sin(e2))) + (sin(e6)*(sin(e5)*(cos(e1)*cos(e2)*cos(e3) - cos(e1)*sin(e2)*sin(e3)) + cos(e5)*(sin(e1)*sin(e4) + cos(e4)*(cos(e1)*cos(e2)*sin(e3) + cos(e1)*cos(e3)*sin(e2)))) - cos(e6)*(cos(e4)*sin(e1) - sin(e4)*(cos(e1)*cos(e2)*sin(e3) + cos(e1)*cos(e3)*sin(e2))))*(cos(e4)*sin(e6)*(a1 + d4*cos(e2 + e3) + a3*sin(e2 + e3) + a2*sin(e2)) - z6*(sin(e6)*(sin(e2 + e3)*sin(e5) - cos(e2 + e3)*cos(e4)*cos(e5)) - cos(e2 + e3)*cos(e6)*sin(e4)) + cos(e5)*cos(e6)*sin(e4)*(a1 + d4*cos(e2 + e3) + a3*sin(e2 + e3) + a2*sin(e2))))) + (de3*(0.5*(sin(e6)*(sin(e2 + e3)*sin(e5) - 1.0*cos(e2 + e3)*cos(e4)*cos(e5)) - 1.0*cos(e2 + e3)*cos(e6)*sin(e4))*(I6xy*(cos(e4)*cos(e6) - 1.0*cos(e5)*sin(e4)*sin(e6)) - 1.0*I6yy*(cos(e4)*sin(e6) + cos(e5)*cos(e6)*sin(e4))) + 0.5*(cos(e4)*sin(e6) + cos(e5)*cos(e6)*sin(e4))*(I6zy*(sin(e2 + e3)*cos(e5) + cos(e2 + e3)*cos(e4)*sin(e5)) + I6xy*(cos(e6)*(sin(e2 + e3)*sin(e5) - 1.0*cos(e2 + e3)*cos(e4)*cos(e5)) + cos(e2 + e3)*sin(e4)*sin(e6)) - 1.0*I6yy*(sin(e6)*(sin(e2 + e3)*sin(e5) - 1.0*cos(e2 + e3)*cos(e4)*cos(e5)) - 1.0*cos(e2 + e3)*cos(e6)*sin(e4))) + 0.5*(cos(e6)*(sin(e2 + e3)*sin(e5) - 1.0*cos(e2 + e3)*cos(e4)*cos(e5)) + cos(e2 + e3)*sin(e4)*sin(e6))*(I6yy*(cos(e4)*cos(e6) - 1.0*cos(e5)*sin(e4)*sin(e6)) + I6xy*(cos(e4)*sin(e6) + cos(e5)*cos(e6)*sin(e4)) - 1.0*I6zy*sin(e4)*sin(e5)) - 0.5*(cos(e4)*cos(e6) - 1.0*cos(e5)*sin(e4)*sin(e6))*(I6zx*(sin(e2 + e3)*cos(e5) + cos(e2 + e3)*cos(e4)*sin(e5)) + I6xx*(cos(e6)*(sin(e2 + e3)*sin(e5) - 1.0*cos(e2 + e3)*cos(e4)*cos(e5)) + cos(e2 + e3)*sin(e4)*sin(e6)) - 1.0*I6yx*(sin(e6)*(sin(e2 + e3)*sin(e5) - 1.0*cos(e2 + e3)*cos(e4)*cos(e5)) - 1.0*cos(e2 + e3)*cos(e6)*sin(e4))) + 0.5*(sin(e6)*(sin(e2 + e3)*sin(e5) - 1.0*cos(e2 + e3)*cos(e4)*cos(e5)) - 1.0*cos(e2 + e3)*cos(e6)*sin(e4))*(I6yx*(cos(e4)*cos(e6) - 1.0*cos(e5)*sin(e4)*sin(e6)) + I6xx*(cos(e4)*sin(e6) + cos(e5)*cos(e6)*sin(e4)) - 1.0*I6zx*sin(e4)*sin(e5)) - 0.5*(I6xz*(cos(e4)*cos(e6) - 1.0*cos(e5)*sin(e4)*sin(e6)) - 1.0*I6yz*(cos(e4)*sin(e6) + cos(e5)*cos(e6)*sin(e4)))*(sin(e2 + e3)*cos(e5) + cos(e2 + e3)*cos(e4)*sin(e5)) + 0.5*(I6yx*(cos(e6)*(sin(e2 + e3)*sin(e5) - 1.0*cos(e2 + e3)*cos(e4)*cos(e5)) + cos(e2 + e3)*sin(e4)*sin(e6)) + I6xx*(sin(e6)*(sin(e2 + e3)*sin(e5) - 1.0*cos(e2 + e3)*cos(e4)*cos(e5)) - 1.0*cos(e2 + e3)*cos(e6)*sin(e4)))*(cos(e4)*sin(e6) + cos(e5)*cos(e6)*sin(e4)) + 0.5*(I6yy*(cos(e6)*(sin(e2 + e3)*sin(e5) - 1.0*cos(e2 + e3)*cos(e4)*cos(e5)) + cos(e2 + e3)*sin(e4)*sin(e6)) + I6xy*(sin(e6)*(sin(e2 + e3)*sin(e5) - 1.0*cos(e2 + e3)*cos(e4)*cos(e5)) - 1.0*cos(e2 + e3)*cos(e6)*sin(e4)))*(cos(e4)*cos(e6) - 1.0*cos(e5)*sin(e4)*sin(e6)) - 0.5*(cos(e6)*(sin(e2 + e3)*sin(e5) - 1.0*cos(e2 + e3)*cos(e4)*cos(e5)) + cos(e2 + e3)*sin(e4)*sin(e6))*(I6xx*(cos(e4)*cos(e6) - 1.0*cos(e5)*sin(e4)*sin(e6)) - 1.0*I6yx*(cos(e4)*sin(e6) + cos(e5)*cos(e6)*sin(e4))) - m6*((sin(e6)*(sin(e5)*(cos(e2)*sin(e3) + cos(e3)*sin(e2)) + cos(e4)*cos(e5)*(sin(e2)*sin(e3) - 1.0*cos(e2)*cos(e3))) + cos(e6)*sin(e4)*(sin(e2)*sin(e3) - 1.0*cos(e2)*cos(e3)))*(x6*(sin(e2 + e3)*cos(e5) + cos(e2 + e3)*cos(e4)*sin(e5)) - 1.0*z6*(cos(e6)*(sin(e2 + e3)*sin(e5) - 1.0*cos(e2 + e3)*cos(e4)*cos(e5)) + cos(e2 + e3)*sin(e4)*sin(e6)) + cos(e4)*cos(e6)*(a1 + d4*cos(e2 + e3) + a3*sin(e2 + e3) + a2*sin(e2)) - 1.0*cos(e5)*sin(e4)*sin(e6)*(a1 + d4*cos(e2 + e3) + a3*sin(e2 + e3) + a2*sin(e2))) + (cos(e6)*(sin(e5)*(cos(e2)*sin(e3) + cos(e3)*sin(e2)) + cos(e4)*cos(e5)*(sin(e2)*sin(e3) - 1.0*cos(e2)*cos(e3))) - 1.0*sin(e4)*sin(e6)*(sin(e2)*sin(e3) - 1.0*cos(e2)*cos(e3)))*(z6*(sin(e6)*(sin(e2 + e3)*sin(e5) - 1.0*cos(e2 + e3)*cos(e4)*cos(e5)) - 1.0*cos(e2 + e3)*cos(e6)*sin(e4)) + y6*(sin(e2 + e3)*cos(e5) + cos(e2 + e3)*cos(e4)*sin(e5)) - 1.0*cos(e4)*sin(e6)*(a1 + d4*cos(e2 + e3) + a3*sin(e2 + e3) + a2*sin(e2)) - 1.0*cos(e5)*cos(e6)*sin(e4)*(a1 + d4*cos(e2 + e3) + a3*sin(e2 + e3) + a2*sin(e2))) - 1.0*(cos(e5)*(cos(e2)*sin(e3) + cos(e3)*sin(e2)) - 1.0*cos(e4)*sin(e5)*(sin(e2)*sin(e3) - 1.0*cos(e2)*cos(e3)))*(x6*(sin(e6)*(sin(e2 + e3)*sin(e5) - 1.0*cos(e2 + e3)*cos(e4)*cos(e5)) - 1.0*cos(e2 + e3)*cos(e6)*sin(e4)) + y6*(cos(e6)*(sin(e2 + e3)*sin(e5) - 1.0*cos(e2 + e3)*cos(e4)*cos(e5)) + cos(e2 + e3)*sin(e4)*sin(e6)) - 1.0*sin(e4)*sin(e5)*(a1 + d4*cos(e2 + e3) + a3*sin(e2 + e3) + a2*sin(e2))))*((sin(e6)*(sin(e5)*(cos(e2)*sin(e3) + cos(e3)*sin(e2)) + cos(e4)*cos(e5)*(sin(e2)*sin(e3) - 1.0*cos(e2)*cos(e3))) + cos(e6)*sin(e4)*(sin(e2)*sin(e3) - 1.0*cos(e2)*cos(e3)))*(cos(e6)*(a3*sin(e5) - 1.0*d4*cos(e4)*cos(e5)) - 1.0*z6*(cos(e4)*cos(e6) - 1.0*cos(e5)*sin(e4)*sin(e6)) + d4*sin(e4)*sin(e6)) + (cos(e6)*(sin(e5)*(cos(e2)*sin(e3) + cos(e3)*sin(e2)) + cos(e4)*cos(e5)*(sin(e2)*sin(e3) - 1.0*cos(e2)*cos(e3))) - 1.0*sin(e4)*sin(e6)*(sin(e2)*sin(e3) - 1.0*cos(e2)*cos(e3)))*(z6*(cos(e4)*sin(e6) + cos(e5)*cos(e6)*sin(e4)) - 1.0*sin(e6)*(a3*sin(e5) - 1.0*d4*cos(e4)*cos(e5)) + d4*cos(e6)*sin(e4)) - 1.0*(cos(e6)*(sin(e5)*(cos(e2)*sin(e3) + cos(e3)*sin(e2)) + cos(e4)*cos(e5)*(sin(e2)*sin(e3) - 1.0*cos(e2)*cos(e3))) - 1.0*sin(e4)*sin(e6)*(sin(e2)*sin(e3) - 1.0*cos(e2)*cos(e3)))*(z6*(cos(e4)*sin(e6) + cos(e5)*cos(e6)*sin(e4)) - 1.0*sin(e6)*(a3*sin(e5) - 1.0*d4*cos(e4)*cos(e5)) + d4*cos(e6)*sin(e4) + x6*sin(e4)*sin(e5)) - 1.0*(y6*(cos(e4)*cos(e6) - 1.0*cos(e5)*sin(e4)*sin(e6)) + x6*(cos(e4)*sin(e6) + cos(e5)*cos(e6)*sin(e4)))*(cos(e5)*(cos(e2)*sin(e3) + cos(e3)*sin(e2)) - 1.0*cos(e4)*sin(e5)*(sin(e2)*sin(e3) - 1.0*cos(e2)*cos(e3))) + (sin(e6)*(sin(e5)*(cos(e2)*sin(e3) + cos(e3)*sin(e2)) + cos(e4)*cos(e5)*(sin(e2)*sin(e3) - 1.0*cos(e2)*cos(e3))) + cos(e6)*sin(e4)*(sin(e2)*sin(e3) - 1.0*cos(e2)*cos(e3)))*(z6*(cos(e4)*cos(e6) - 1.0*cos(e5)*sin(e4)*sin(e6)) - 1.0*cos(e6)*(a3*sin(e5) - 1.0*d4*cos(e4)*cos(e5)) - 1.0*d4*sin(e4)*sin(e6) + y6*sin(e4)*sin(e5))) - m6*(1.0*(sin(e5)*(cos(e1)*sin(e4) - 1.0*cos(e4)*(cos(e2)*sin(e1)*sin(e3) + cos(e3)*sin(e1)*sin(e2))) + cos(e5)*(cos(e2)*cos(e3)*sin(e1) - 1.0*sin(e1)*sin(e2)*sin(e3)))*(x6*(cos(e4)*cos(e6) - 1.0*cos(e5)*sin(e4)*sin(e6)) - 1.0*y6*(cos(e4)*sin(e6) + cos(e5)*cos(e6)*sin(e4)) + a3*cos(e5) + d4*cos(e4)*sin(e5)) + (sin(e6)*(1.0*cos(e5)*(cos(e1)*sin(e4) - 1.0*cos(e4)*(cos(e2)*sin(e1)*sin(e3) + cos(e3)*sin(e1)*sin(e2))) - sin(e5)*(cos(e2)*cos(e3)*sin(e1) - 1.0*sin(e1)*sin(e2)*sin(e3))) - cos(e6)*(sin(e4)*(cos(e2)*sin(e1)*sin(e3) + cos(e3)*sin(e1)*sin(e2)) + cos(e1)*cos(e4)))*(z6*(cos(e4)*sin(e6) + cos(e5)*cos(e6)*sin(e4)) - 1.0*sin(e6)*(a3*sin(e5) - 1.0*d4*cos(e4)*cos(e5)) + d4*cos(e6)*sin(e4) + x6*sin(e4)*sin(e5)) + (cos(e6)*(1.0*cos(e5)*(cos(e1)*sin(e4) - 1.0*cos(e4)*(cos(e2)*sin(e1)*sin(e3) + cos(e3)*sin(e1)*sin(e2))) - sin(e5)*(cos(e2)*cos(e3)*sin(e1) - 1.0*sin(e1)*sin(e2)*sin(e3))) + 1.0*sin(e6)*(sin(e4)*(cos(e2)*sin(e1)*sin(e3) + cos(e3)*sin(e1)*sin(e2)) + cos(e1)*cos(e4)))*(z6*(cos(e4)*cos(e6) - 1.0*cos(e5)*sin(e4)*sin(e6)) - 1.0*cos(e6)*(a3*sin(e5) - 1.0*d4*cos(e4)*cos(e5)) - 1.0*d4*sin(e4)*sin(e6) + y6*sin(e4)*sin(e5)))*((1.0*y6*(sin(e6)*(sin(e2 + e3)*sin(e5) - 1.0*cos(e2 + e3)*cos(e4)*cos(e5)) - 1.0*cos(e2 + e3)*cos(e6)*sin(e4)) - x6*(cos(e6)*(sin(e2 + e3)*sin(e5) - 1.0*cos(e2 + e3)*cos(e4)*cos(e5)) + cos(e2 + e3)*sin(e4)*sin(e6)))*(sin(e5)*(cos(e1)*sin(e4) - 1.0*cos(e4)*(cos(e2)*sin(e1)*sin(e3) + cos(e3)*sin(e1)*sin(e2))) + cos(e5)*(cos(e2)*cos(e3)*sin(e1) - 1.0*sin(e1)*sin(e2)*sin(e3))) - 1.0*(cos(e6)*(1.0*cos(e5)*(cos(e1)*sin(e4) - 1.0*cos(e4)*(cos(e2)*sin(e1)*sin(e3) + cos(e3)*sin(e1)*sin(e2))) - sin(e5)*(cos(e2)*cos(e3)*sin(e1) - 1.0*sin(e1)*sin(e2)*sin(e3))) + 1.0*sin(e6)*(sin(e4)*(cos(e2)*sin(e1)*sin(e3) + cos(e3)*sin(e1)*sin(e2)) + cos(e1)*cos(e4)))*(x6*(sin(e2 + e3)*cos(e5) + cos(e2 + e3)*cos(e4)*sin(e5)) - 1.0*z6*(cos(e6)*(sin(e2 + e3)*sin(e5) - 1.0*cos(e2 + e3)*cos(e4)*cos(e5)) + cos(e2 + e3)*sin(e4)*sin(e6)) + cos(e4)*cos(e6)*(a1 + d4*cos(e2 + e3) + a3*sin(e2 + e3) + a2*sin(e2)) - 1.0*cos(e5)*sin(e4)*sin(e6)*(a1 + d4*cos(e2 + e3) + a3*sin(e2 + e3) + a2*sin(e2))) + (sin(e6)*(1.0*cos(e5)*(cos(e1)*sin(e4) - 1.0*cos(e4)*(cos(e2)*sin(e1)*sin(e3) + cos(e3)*sin(e1)*sin(e2))) - sin(e5)*(cos(e2)*cos(e3)*sin(e1) - 1.0*sin(e1)*sin(e2)*sin(e3))) - cos(e6)*(sin(e4)*(cos(e2)*sin(e1)*sin(e3) + cos(e3)*sin(e1)*sin(e2)) + cos(e1)*cos(e4)))*(z6*(sin(e6)*(sin(e2 + e3)*sin(e5) - 1.0*cos(e2 + e3)*cos(e4)*cos(e5)) - 1.0*cos(e2 + e3)*cos(e6)*sin(e4)) + y6*(sin(e2 + e3)*cos(e5) + cos(e2 + e3)*cos(e4)*sin(e5)) - 1.0*cos(e4)*sin(e6)*(a1 + d4*cos(e2 + e3) + a3*sin(e2 + e3) + a2*sin(e2)) - 1.0*cos(e5)*cos(e6)*sin(e4)*(a1 + d4*cos(e2 + e3) + a3*sin(e2 + e3) + a2*sin(e2))) - 1.0*(cos(e6)*(1.0*cos(e5)*(cos(e1)*sin(e4) - 1.0*cos(e4)*(cos(e2)*sin(e1)*sin(e3) + cos(e3)*sin(e1)*sin(e2))) - sin(e5)*(cos(e2)*cos(e3)*sin(e1) - 1.0*sin(e1)*sin(e2)*sin(e3))) + 1.0*sin(e6)*(sin(e4)*(cos(e2)*sin(e1)*sin(e3) + cos(e3)*sin(e1)*sin(e2)) + cos(e1)*cos(e4)))*(z6*(cos(e6)*(sin(e2 + e3)*sin(e5) - 1.0*cos(e2 + e3)*cos(e4)*cos(e5)) + cos(e2 + e3)*sin(e4)*sin(e6)) - 1.0*cos(e4)*cos(e6)*(a1 + d4*cos(e2 + e3) + a3*sin(e2 + e3) + a2*sin(e2)) + cos(e5)*sin(e4)*sin(e6)*(a1 + d4*cos(e2 + e3) + a3*sin(e2 + e3) + a2*sin(e2))) + (sin(e6)*(1.0*cos(e5)*(cos(e1)*sin(e4) - 1.0*cos(e4)*(cos(e2)*sin(e1)*sin(e3) + cos(e3)*sin(e1)*sin(e2))) - sin(e5)*(cos(e2)*cos(e3)*sin(e1) - 1.0*sin(e1)*sin(e2)*sin(e3))) - cos(e6)*(sin(e4)*(cos(e2)*sin(e1)*sin(e3) + cos(e3)*sin(e1)*sin(e2)) + cos(e1)*cos(e4)))*(cos(e4)*sin(e6)*(a1 + d4*cos(e2 + e3) + a3*sin(e2 + e3) + a2*sin(e2)) - 1.0*z6*(sin(e6)*(sin(e2 + e3)*sin(e5) - 1.0*cos(e2 + e3)*cos(e4)*cos(e5)) - 1.0*cos(e2 + e3)*cos(e6)*sin(e4)) + cos(e5)*cos(e6)*sin(e4)*(a1 + d4*cos(e2 + e3) + a3*sin(e2 + e3) + a2*sin(e2)))) - 0.5*sin(e4)*sin(e5)*(I6yz*(cos(e6)*(sin(e2 + e3)*sin(e5) - 1.0*cos(e2 + e3)*cos(e4)*cos(e5)) + cos(e2 + e3)*sin(e4)*sin(e6)) + I6xz*(sin(e6)*(sin(e2 + e3)*sin(e5) - 1.0*cos(e2 + e3)*cos(e4)*cos(e5)) - 1.0*cos(e2 + e3)*cos(e6)*sin(e4))) + m6*((cos(e6)*(sin(e5)*(cos(e2)*sin(e3) + cos(e3)*sin(e2)) + cos(e4)*cos(e5)*(sin(e2)*sin(e3) - 1.0*cos(e2)*cos(e3))) - 1.0*sin(e4)*sin(e6)*(sin(e2)*sin(e3) - 1.0*cos(e2)*cos(e3)))*(z6*(cos(e4)*cos(e6) - 1.0*cos(e5)*sin(e4)*sin(e6)) - 1.0*cos(e6)*(a3*sin(e5) - 1.0*d4*cos(e4)*cos(e5)) - 1.0*d4*sin(e4)*sin(e6) + y6*sin(e4)*sin(e5)) + (sin(e6)*(sin(e5)*(cos(e2)*sin(e3) + cos(e3)*sin(e2)) + cos(e4)*cos(e5)*(sin(e2)*sin(e3) - 1.0*cos(e2)*cos(e3))) + cos(e6)*sin(e4)*(sin(e2)*sin(e3) - 1.0*cos(e2)*cos(e3)))*(z6*(cos(e4)*sin(e6) + cos(e5)*cos(e6)*sin(e4)) - 1.0*sin(e6)*(a3*sin(e5) - 1.0*d4*cos(e4)*cos(e5)) + d4*cos(e6)*sin(e4) + x6*sin(e4)*sin(e5)) - 1.0*(cos(e5)*(cos(e2)*sin(e3) + cos(e3)*sin(e2)) - 1.0*cos(e4)*sin(e5)*(sin(e2)*sin(e3) - 1.0*cos(e2)*cos(e3)))*(x6*(cos(e4)*cos(e6) - 1.0*cos(e5)*sin(e4)*sin(e6)) - 1.0*y6*(cos(e4)*sin(e6) + cos(e5)*cos(e6)*sin(e4)) + a3*cos(e5) + d4*cos(e4)*sin(e5)))*(1.0*(cos(e6)*(sin(e5)*(cos(e2)*sin(e3) + cos(e3)*sin(e2)) + cos(e4)*cos(e5)*(sin(e2)*sin(e3) - 1.0*cos(e2)*cos(e3))) - 1.0*sin(e4)*sin(e6)*(sin(e2)*sin(e3) - 1.0*cos(e2)*cos(e3)))*(x6*(sin(e2 + e3)*cos(e5) + cos(e2 + e3)*cos(e4)*sin(e5)) - 1.0*z6*(cos(e6)*(sin(e2 + e3)*sin(e5) - 1.0*cos(e2 + e3)*cos(e4)*cos(e5)) + cos(e2 + e3)*sin(e4)*sin(e6)) + cos(e4)*cos(e6)*(a1 + d4*cos(e2 + e3) + a3*sin(e2 + e3) + a2*sin(e2)) - 1.0*cos(e5)*sin(e4)*sin(e6)*(a1 + d4*cos(e2 + e3) + a3*sin(e2 + e3) + a2*sin(e2))) - (sin(e6)*(sin(e5)*(cos(e2)*sin(e3) + cos(e3)*sin(e2)) + cos(e4)*cos(e5)*(sin(e2)*sin(e3) - 1.0*cos(e2)*cos(e3))) + cos(e6)*sin(e4)*(sin(e2)*sin(e3) - 1.0*cos(e2)*cos(e3)))*(z6*(sin(e6)*(sin(e2 + e3)*sin(e5) - 1.0*cos(e2 + e3)*cos(e4)*cos(e5)) - 1.0*cos(e2 + e3)*cos(e6)*sin(e4)) + y6*(sin(e2 + e3)*cos(e5) + cos(e2 + e3)*cos(e4)*sin(e5)) - 1.0*cos(e4)*sin(e6)*(a1 + d4*cos(e2 + e3) + a3*sin(e2 + e3) + a2*sin(e2)) - 1.0*cos(e5)*cos(e6)*sin(e4)*(a1 + d4*cos(e2 + e3) + a3*sin(e2 + e3) + a2*sin(e2))) - (sin(e6)*(sin(e5)*(cos(e2)*sin(e3) + cos(e3)*sin(e2)) + cos(e4)*cos(e5)*(sin(e2)*sin(e3) - 1.0*cos(e2)*cos(e3))) + cos(e6)*sin(e4)*(sin(e2)*sin(e3) - 1.0*cos(e2)*cos(e3)))*(cos(e4)*sin(e6)*(a1 + d4*cos(e2 + e3) + a3*sin(e2 + e3) + a2*sin(e2)) - 1.0*z6*(sin(e6)*(sin(e2 + e3)*sin(e5) - 1.0*cos(e2 + e3)*cos(e4)*cos(e5)) - 1.0*cos(e2 + e3)*cos(e6)*sin(e4)) + cos(e5)*cos(e6)*sin(e4)*(a1 + d4*cos(e2 + e3) + a3*sin(e2 + e3) + a2*sin(e2))) + 1.0*(cos(e6)*(sin(e5)*(cos(e2)*sin(e3) + cos(e3)*sin(e2)) + cos(e4)*cos(e5)*(sin(e2)*sin(e3) - 1.0*cos(e2)*cos(e3))) - 1.0*sin(e4)*sin(e6)*(sin(e2)*sin(e3) - 1.0*cos(e2)*cos(e3)))*(z6*(cos(e6)*(sin(e2 + e3)*sin(e5) - 1.0*cos(e2 + e3)*cos(e4)*cos(e5)) + cos(e2 + e3)*sin(e4)*sin(e6)) - 1.0*cos(e4)*cos(e6)*(a1 + d4*cos(e2 + e3) + a3*sin(e2 + e3) + a2*sin(e2)) + cos(e5)*sin(e4)*sin(e6)*(a1 + d4*cos(e2 + e3) + a3*sin(e2 + e3) + a2*sin(e2))) + (1.0*y6*(sin(e6)*(sin(e2 + e3)*sin(e5) - 1.0*cos(e2 + e3)*cos(e4)*cos(e5)) - 1.0*cos(e2 + e3)*cos(e6)*sin(e4)) - x6*(cos(e6)*(sin(e2 + e3)*sin(e5) - 1.0*cos(e2 + e3)*cos(e4)*cos(e5)) + cos(e2 + e3)*sin(e4)*sin(e6)))*(cos(e5)*(cos(e2)*sin(e3) + cos(e3)*sin(e2)) - 1.0*cos(e4)*sin(e5)*(sin(e2)*sin(e3) - 1.0*cos(e2)*cos(e3)))) - m6*((sin(e6)*(sin(e5)*(cos(e1)*cos(e2)*cos(e3) - 1.0*cos(e1)*sin(e2)*sin(e3)) + cos(e5)*(sin(e1)*sin(e4) + cos(e4)*(cos(e1)*cos(e2)*sin(e3) + cos(e1)*cos(e3)*sin(e2)))) - 1.0*cos(e6)*(cos(e4)*sin(e1) - 1.0*sin(e4)*(cos(e1)*cos(e2)*sin(e3) + cos(e1)*cos(e3)*sin(e2))))*(x6*(sin(e2 + e3)*cos(e5) + cos(e2 + e3)*cos(e4)*sin(e5)) - 1.0*z6*(cos(e6)*(sin(e2 + e3)*sin(e5) - 1.0*cos(e2 + e3)*cos(e4)*cos(e5)) + cos(e2 + e3)*sin(e4)*sin(e6)) + cos(e4)*cos(e6)*(a1 + d4*cos(e2 + e3) + a3*sin(e2 + e3) + a2*sin(e2)) - 1.0*cos(e5)*sin(e4)*sin(e6)*(a1 + d4*cos(e2 + e3) + a3*sin(e2 + e3) + a2*sin(e2))) + (sin(e6)*(cos(e4)*sin(e1) - 1.0*sin(e4)*(cos(e1)*cos(e2)*sin(e3) + cos(e1)*cos(e3)*sin(e2))) + cos(e6)*(sin(e5)*(cos(e1)*cos(e2)*cos(e3) - 1.0*cos(e1)*sin(e2)*sin(e3)) + cos(e5)*(sin(e1)*sin(e4) + cos(e4)*(cos(e1)*cos(e2)*sin(e3) + cos(e1)*cos(e3)*sin(e2)))))*(z6*(sin(e6)*(sin(e2 + e3)*sin(e5) - 1.0*cos(e2 + e3)*cos(e4)*cos(e5)) - 1.0*cos(e2 + e3)*cos(e6)*sin(e4)) + y6*(sin(e2 + e3)*cos(e5) + cos(e2 + e3)*cos(e4)*sin(e5)) - 1.0*cos(e4)*sin(e6)*(a1 + d4*cos(e2 + e3) + a3*sin(e2 + e3) + a2*sin(e2)) - 1.0*cos(e5)*cos(e6)*sin(e4)*(a1 + d4*cos(e2 + e3) + a3*sin(e2 + e3) + a2*sin(e2))) - 1.0*(cos(e5)*(cos(e1)*cos(e2)*cos(e3) - 1.0*cos(e1)*sin(e2)*sin(e3)) - 1.0*sin(e5)*(sin(e1)*sin(e4) + cos(e4)*(cos(e1)*cos(e2)*sin(e3) + cos(e1)*cos(e3)*sin(e2))))*(x6*(sin(e6)*(sin(e2 + e3)*sin(e5) - 1.0*cos(e2 + e3)*cos(e4)*cos(e5)) - 1.0*cos(e2 + e3)*cos(e6)*sin(e4)) + y6*(cos(e6)*(sin(e2 + e3)*sin(e5) - 1.0*cos(e2 + e3)*cos(e4)*cos(e5)) + cos(e2 + e3)*sin(e4)*sin(e6)) - 1.0*sin(e4)*sin(e5)*(a1 + d4*cos(e2 + e3) + a3*sin(e2 + e3) + a2*sin(e2))))*((sin(e6)*(cos(e4)*sin(e1) - 1.0*sin(e4)*(cos(e1)*cos(e2)*sin(e3) + cos(e1)*cos(e3)*sin(e2))) + cos(e6)*(sin(e5)*(cos(e1)*cos(e2)*cos(e3) - 1.0*cos(e1)*sin(e2)*sin(e3)) + cos(e5)*(sin(e1)*sin(e4) + cos(e4)*(cos(e1)*cos(e2)*sin(e3) + cos(e1)*cos(e3)*sin(e2)))))*(z6*(cos(e4)*sin(e6) + cos(e5)*cos(e6)*sin(e4)) - 1.0*sin(e6)*(a3*sin(e5) - 1.0*d4*cos(e4)*cos(e5)) + d4*cos(e6)*sin(e4)) + (sin(e6)*(sin(e5)*(cos(e1)*cos(e2)*cos(e3) - 1.0*cos(e1)*sin(e2)*sin(e3)) + cos(e5)*(sin(e1)*sin(e4) + cos(e4)*(cos(e1)*cos(e2)*sin(e3) + cos(e1)*cos(e3)*sin(e2)))) - 1.0*cos(e6)*(cos(e4)*sin(e1) - 1.0*sin(e4)*(cos(e1)*cos(e2)*sin(e3) + cos(e1)*cos(e3)*sin(e2))))*(z6*(cos(e4)*cos(e6) - 1.0*cos(e5)*sin(e4)*sin(e6)) - 1.0*cos(e6)*(a3*sin(e5) - 1.0*d4*cos(e4)*cos(e5)) - 1.0*d4*sin(e4)*sin(e6) + y6*sin(e4)*sin(e5)) + (sin(e6)*(sin(e5)*(cos(e1)*cos(e2)*cos(e3) - 1.0*cos(e1)*sin(e2)*sin(e3)) + cos(e5)*(sin(e1)*sin(e4) + cos(e4)*(cos(e1)*cos(e2)*sin(e3) + cos(e1)*cos(e3)*sin(e2)))) - 1.0*cos(e6)*(cos(e4)*sin(e1) - 1.0*sin(e4)*(cos(e1)*cos(e2)*sin(e3) + cos(e1)*cos(e3)*sin(e2))))*(cos(e6)*(a3*sin(e5) - 1.0*d4*cos(e4)*cos(e5)) - 1.0*z6*(cos(e4)*cos(e6) - 1.0*cos(e5)*sin(e4)*sin(e6)) + d4*sin(e4)*sin(e6)) - 1.0*(sin(e6)*(cos(e4)*sin(e1) - 1.0*sin(e4)*(cos(e1)*cos(e2)*sin(e3) + cos(e1)*cos(e3)*sin(e2))) + cos(e6)*(sin(e5)*(cos(e1)*cos(e2)*cos(e3) - 1.0*cos(e1)*sin(e2)*sin(e3)) + cos(e5)*(sin(e1)*sin(e4) + cos(e4)*(cos(e1)*cos(e2)*sin(e3) + cos(e1)*cos(e3)*sin(e2)))))*(z6*(cos(e4)*sin(e6) + cos(e5)*cos(e6)*sin(e4)) - 1.0*sin(e6)*(a3*sin(e5) - 1.0*d4*cos(e4)*cos(e5)) + d4*cos(e6)*sin(e4) + x6*sin(e4)*sin(e5)) - 1.0*(y6*(cos(e4)*cos(e6) - 1.0*cos(e5)*sin(e4)*sin(e6)) + x6*(cos(e4)*sin(e6) + cos(e5)*cos(e6)*sin(e4)))*(cos(e5)*(cos(e1)*cos(e2)*cos(e3) - 1.0*cos(e1)*sin(e2)*sin(e3)) - 1.0*sin(e5)*(sin(e1)*sin(e4) + cos(e4)*(cos(e1)*cos(e2)*sin(e3) + cos(e1)*cos(e3)*sin(e2))))) + m6*((sin(e6)*(cos(e4)*sin(e1) - 1.0*sin(e4)*(cos(e1)*cos(e2)*sin(e3) + cos(e1)*cos(e3)*sin(e2))) + cos(e6)*(sin(e5)*(cos(e1)*cos(e2)*cos(e3) - 1.0*cos(e1)*sin(e2)*sin(e3)) + cos(e5)*(sin(e1)*sin(e4) + cos(e4)*(cos(e1)*cos(e2)*sin(e3) + cos(e1)*cos(e3)*sin(e2)))))*(z6*(cos(e4)*cos(e6) - 1.0*cos(e5)*sin(e4)*sin(e6)) - 1.0*cos(e6)*(a3*sin(e5) - 1.0*d4*cos(e4)*cos(e5)) - 1.0*d4*sin(e4)*sin(e6) + y6*sin(e4)*sin(e5)) - 1.0*(cos(e5)*(cos(e1)*cos(e2)*cos(e3) - 1.0*cos(e1)*sin(e2)*sin(e3)) - 1.0*sin(e5)*(sin(e1)*sin(e4) + cos(e4)*(cos(e1)*cos(e2)*sin(e3) + cos(e1)*cos(e3)*sin(e2))))*(x6*(cos(e4)*cos(e6) - 1.0*cos(e5)*sin(e4)*sin(e6)) - 1.0*y6*(cos(e4)*sin(e6) + cos(e5)*cos(e6)*sin(e4)) + a3*cos(e5) + d4*cos(e4)*sin(e5)) + (sin(e6)*(sin(e5)*(cos(e1)*cos(e2)*cos(e3) - 1.0*cos(e1)*sin(e2)*sin(e3)) + cos(e5)*(sin(e1)*sin(e4) + cos(e4)*(cos(e1)*cos(e2)*sin(e3) + cos(e1)*cos(e3)*sin(e2)))) - 1.0*cos(e6)*(cos(e4)*sin(e1) - 1.0*sin(e4)*(cos(e1)*cos(e2)*sin(e3) + cos(e1)*cos(e3)*sin(e2))))*(z6*(cos(e4)*sin(e6) + cos(e5)*cos(e6)*sin(e4)) - 1.0*sin(e6)*(a3*sin(e5) - 1.0*d4*cos(e4)*cos(e5)) + d4*cos(e6)*sin(e4) + x6*sin(e4)*sin(e5)))*(1.0*(sin(e6)*(cos(e4)*sin(e1) - 1.0*sin(e4)*(cos(e1)*cos(e2)*sin(e3) + cos(e1)*cos(e3)*sin(e2))) + cos(e6)*(sin(e5)*(cos(e1)*cos(e2)*cos(e3) - 1.0*cos(e1)*sin(e2)*sin(e3)) + cos(e5)*(sin(e1)*sin(e4) + cos(e4)*(cos(e1)*cos(e2)*sin(e3) + cos(e1)*cos(e3)*sin(e2)))))*(x6*(sin(e2 + e3)*cos(e5) + cos(e2 + e3)*cos(e4)*sin(e5)) - 1.0*z6*(cos(e6)*(sin(e2 + e3)*sin(e5) - 1.0*cos(e2 + e3)*cos(e4)*cos(e5)) + cos(e2 + e3)*sin(e4)*sin(e6)) + cos(e4)*cos(e6)*(a1 + d4*cos(e2 + e3) + a3*sin(e2 + e3) + a2*sin(e2)) - 1.0*cos(e5)*sin(e4)*sin(e6)*(a1 + d4*cos(e2 + e3) + a3*sin(e2 + e3) + a2*sin(e2))) - (sin(e6)*(sin(e5)*(cos(e1)*cos(e2)*cos(e3) - 1.0*cos(e1)*sin(e2)*sin(e3)) + cos(e5)*(sin(e1)*sin(e4) + cos(e4)*(cos(e1)*cos(e2)*sin(e3) + cos(e1)*cos(e3)*sin(e2)))) - 1.0*cos(e6)*(cos(e4)*sin(e1) - 1.0*sin(e4)*(cos(e1)*cos(e2)*sin(e3) + cos(e1)*cos(e3)*sin(e2))))*(cos(e4)*sin(e6)*(a1 + d4*cos(e2 + e3) + a3*sin(e2 + e3) + a2*sin(e2)) - 1.0*z6*(sin(e6)*(sin(e2 + e3)*sin(e5) - 1.0*cos(e2 + e3)*cos(e4)*cos(e5)) - 1.0*cos(e2 + e3)*cos(e6)*sin(e4)) + cos(e5)*cos(e6)*sin(e4)*(a1 + d4*cos(e2 + e3) + a3*sin(e2 + e3) + a2*sin(e2))) - (sin(e6)*(sin(e5)*(cos(e1)*cos(e2)*cos(e3) - 1.0*cos(e1)*sin(e2)*sin(e3)) + cos(e5)*(sin(e1)*sin(e4) + cos(e4)*(cos(e1)*cos(e2)*sin(e3) + cos(e1)*cos(e3)*sin(e2)))) - 1.0*cos(e6)*(cos(e4)*sin(e1) - 1.0*sin(e4)*(cos(e1)*cos(e2)*sin(e3) + cos(e1)*cos(e3)*sin(e2))))*(z6*(sin(e6)*(sin(e2 + e3)*sin(e5) - 1.0*cos(e2 + e3)*cos(e4)*cos(e5)) - 1.0*cos(e2 + e3)*cos(e6)*sin(e4)) + y6*(sin(e2 + e3)*cos(e5) + cos(e2 + e3)*cos(e4)*sin(e5)) - 1.0*cos(e4)*sin(e6)*(a1 + d4*cos(e2 + e3) + a3*sin(e2 + e3) + a2*sin(e2)) - 1.0*cos(e5)*cos(e6)*sin(e4)*(a1 + d4*cos(e2 + e3) + a3*sin(e2 + e3) + a2*sin(e2))) + 1.0*(sin(e6)*(cos(e4)*sin(e1) - 1.0*sin(e4)*(cos(e1)*cos(e2)*sin(e3) + cos(e1)*cos(e3)*sin(e2))) + cos(e6)*(sin(e5)*(cos(e1)*cos(e2)*cos(e3) - 1.0*cos(e1)*sin(e2)*sin(e3)) + cos(e5)*(sin(e1)*sin(e4) + cos(e4)*(cos(e1)*cos(e2)*sin(e3) + cos(e1)*cos(e3)*sin(e2)))))*(z6*(cos(e6)*(sin(e2 + e3)*sin(e5) - 1.0*cos(e2 + e3)*cos(e4)*cos(e5)) + cos(e2 + e3)*sin(e4)*sin(e6)) - 1.0*cos(e4)*cos(e6)*(a1 + d4*cos(e2 + e3) + a3*sin(e2 + e3) + a2*sin(e2)) + cos(e5)*sin(e4)*sin(e6)*(a1 + d4*cos(e2 + e3) + a3*sin(e2 + e3) + a2*sin(e2))) + (cos(e5)*(cos(e1)*cos(e2)*cos(e3) - 1.0*cos(e1)*sin(e2)*sin(e3)) - 1.0*sin(e5)*(sin(e1)*sin(e4) + cos(e4)*(cos(e1)*cos(e2)*sin(e3) + cos(e1)*cos(e3)*sin(e2))))*(1.0*y6*(sin(e6)*(sin(e2 + e3)*sin(e5) - 1.0*cos(e2 + e3)*cos(e4)*cos(e5)) - 1.0*cos(e2 + e3)*cos(e6)*sin(e4)) - x6*(cos(e6)*(sin(e2 + e3)*sin(e5) - 1.0*cos(e2 + e3)*cos(e4)*cos(e5)) + cos(e2 + e3)*sin(e4)*sin(e6)))) - m6*((sin(e6)*(1.0*cos(e5)*(cos(e1)*sin(e4) - 1.0*cos(e4)*(cos(e2)*sin(e1)*sin(e3) + cos(e3)*sin(e1)*sin(e2))) - sin(e5)*(cos(e2)*cos(e3)*sin(e1) - 1.0*sin(e1)*sin(e2)*sin(e3))) - cos(e6)*(sin(e4)*(cos(e2)*sin(e1)*sin(e3) + cos(e3)*sin(e1)*sin(e2)) + cos(e1)*cos(e4)))*(x6*(sin(e2 + e3)*cos(e5) + cos(e2 + e3)*cos(e4)*sin(e5)) - 1.0*z6*(cos(e6)*(sin(e2 + e3)*sin(e5) - 1.0*cos(e2 + e3)*cos(e4)*cos(e5)) + cos(e2 + e3)*sin(e4)*sin(e6)) + cos(e4)*cos(e6)*(a1 + d4*cos(e2 + e3) + a3*sin(e2 + e3) + a2*sin(e2)) - 1.0*cos(e5)*sin(e4)*sin(e6)*(a1 + d4*cos(e2 + e3) + a3*sin(e2 + e3) + a2*sin(e2))) + 1.0*(sin(e5)*(cos(e1)*sin(e4) - 1.0*cos(e4)*(cos(e2)*sin(e1)*sin(e3) + cos(e3)*sin(e1)*sin(e2))) + cos(e5)*(cos(e2)*cos(e3)*sin(e1) - 1.0*sin(e1)*sin(e2)*sin(e3)))*(x6*(sin(e6)*(sin(e2 + e3)*sin(e5) - 1.0*cos(e2 + e3)*cos(e4)*cos(e5)) - 1.0*cos(e2 + e3)*cos(e6)*sin(e4)) + y6*(cos(e6)*(sin(e2 + e3)*sin(e5) - 1.0*cos(e2 + e3)*cos(e4)*cos(e5)) + cos(e2 + e3)*sin(e4)*sin(e6)) - 1.0*sin(e4)*sin(e5)*(a1 + d4*cos(e2 + e3) + a3*sin(e2 + e3) + a2*sin(e2))) + (cos(e6)*(1.0*cos(e5)*(cos(e1)*sin(e4) - 1.0*cos(e4)*(cos(e2)*sin(e1)*sin(e3) + cos(e3)*sin(e1)*sin(e2))) - sin(e5)*(cos(e2)*cos(e3)*sin(e1) - 1.0*sin(e1)*sin(e2)*sin(e3))) + 1.0*sin(e6)*(sin(e4)*(cos(e2)*sin(e1)*sin(e3) + cos(e3)*sin(e1)*sin(e2)) + cos(e1)*cos(e4)))*(z6*(sin(e6)*(sin(e2 + e3)*sin(e5) - 1.0*cos(e2 + e3)*cos(e4)*cos(e5)) - 1.0*cos(e2 + e3)*cos(e6)*sin(e4)) + y6*(sin(e2 + e3)*cos(e5) + cos(e2 + e3)*cos(e4)*sin(e5)) - 1.0*cos(e4)*sin(e6)*(a1 + d4*cos(e2 + e3) + a3*sin(e2 + e3) + a2*sin(e2)) - 1.0*cos(e5)*cos(e6)*sin(e4)*(a1 + d4*cos(e2 + e3) + a3*sin(e2 + e3) + a2*sin(e2))))*((sin(e6)*(1.0*cos(e5)*(cos(e1)*sin(e4) - 1.0*cos(e4)*(cos(e2)*sin(e1)*sin(e3) + cos(e3)*sin(e1)*sin(e2))) - sin(e5)*(cos(e2)*cos(e3)*sin(e1) - 1.0*sin(e1)*sin(e2)*sin(e3))) - cos(e6)*(sin(e4)*(cos(e2)*sin(e1)*sin(e3) + cos(e3)*sin(e1)*sin(e2)) + cos(e1)*cos(e4)))*(z6*(cos(e4)*cos(e6) - 1.0*cos(e5)*sin(e4)*sin(e6)) - 1.0*cos(e6)*(a3*sin(e5) - 1.0*d4*cos(e4)*cos(e5)) - 1.0*d4*sin(e4)*sin(e6) + y6*sin(e4)*sin(e5)) - 1.0*(cos(e6)*(1.0*cos(e5)*(cos(e1)*sin(e4) - 1.0*cos(e4)*(cos(e2)*sin(e1)*sin(e3) + cos(e3)*sin(e1)*sin(e2))) - sin(e5)*(cos(e2)*cos(e3)*sin(e1) - 1.0*sin(e1)*sin(e2)*sin(e3))) + 1.0*sin(e6)*(sin(e4)*(cos(e2)*sin(e1)*sin(e3) + cos(e3)*sin(e1)*sin(e2)) + cos(e1)*cos(e4)))*(z6*(cos(e4)*sin(e6) + cos(e5)*cos(e6)*sin(e4)) - 1.0*sin(e6)*(a3*sin(e5) - 1.0*d4*cos(e4)*cos(e5)) + d4*cos(e6)*sin(e4) + x6*sin(e4)*sin(e5)) + 1.0*(y6*(cos(e4)*cos(e6) - 1.0*cos(e5)*sin(e4)*sin(e6)) + x6*(cos(e4)*sin(e6) + cos(e5)*cos(e6)*sin(e4)))*(sin(e5)*(cos(e1)*sin(e4) - 1.0*cos(e4)*(cos(e2)*sin(e1)*sin(e3) + cos(e3)*sin(e1)*sin(e2))) + cos(e5)*(cos(e2)*cos(e3)*sin(e1) - 1.0*sin(e1)*sin(e2)*sin(e3))) + (cos(e6)*(1.0*cos(e5)*(cos(e1)*sin(e4) - 1.0*cos(e4)*(cos(e2)*sin(e1)*sin(e3) + cos(e3)*sin(e1)*sin(e2))) - sin(e5)*(cos(e2)*cos(e3)*sin(e1) - 1.0*sin(e1)*sin(e2)*sin(e3))) + 1.0*sin(e6)*(sin(e4)*(cos(e2)*sin(e1)*sin(e3) + cos(e3)*sin(e1)*sin(e2)) + cos(e1)*cos(e4)))*(z6*(cos(e4)*sin(e6) + cos(e5)*cos(e6)*sin(e4)) - 1.0*sin(e6)*(a3*sin(e5) - 1.0*d4*cos(e4)*cos(e5)) + d4*cos(e6)*sin(e4)) + (sin(e6)*(1.0*cos(e5)*(cos(e1)*sin(e4) - 1.0*cos(e4)*(cos(e2)*sin(e1)*sin(e3) + cos(e3)*sin(e1)*sin(e2))) - sin(e5)*(cos(e2)*cos(e3)*sin(e1) - 1.0*sin(e1)*sin(e2)*sin(e3))) - cos(e6)*(sin(e4)*(cos(e2)*sin(e1)*sin(e3) + cos(e3)*sin(e1)*sin(e2)) + cos(e1)*cos(e4)))*(cos(e6)*(a3*sin(e5) - 1.0*d4*cos(e4)*cos(e5)) - 1.0*z6*(cos(e4)*cos(e6) - 1.0*cos(e5)*sin(e4)*sin(e6)) + d4*sin(e4)*sin(e6)))))/2 + de3*((I6yz*(sin(e6)*(cos(e2 + e3)*sin(e5) + sin(e2 + e3)*cos(e4)*cos(e5)) + sin(e2 + e3)*cos(e6)*sin(e4)))/2 - (I6xz*(cos(e6)*(cos(e2 + e3)*sin(e5) + sin(e2 + e3)*cos(e4)*cos(e5)) - sin(e2 + e3)*sin(e4)*sin(e6)))/2 - I6zz*(cos(e2 + e3)*cos(e5) - sin(e2 + e3)*cos(e4)*sin(e5)) - (I6zx*(cos(e6)*(cos(e2 + e3)*sin(e5) + sin(e2 + e3)*cos(e4)*cos(e5)) - sin(e2 + e3)*sin(e4)*sin(e6)))/2 + (I6zy*(sin(e6)*(cos(e2 + e3)*sin(e5) + sin(e2 + e3)*cos(e4)*cos(e5)) + sin(e2 + e3)*cos(e6)*sin(e4)))/2 + m6*(x6*(sin(e6)*(sin(e5)*(cos(e1)*cos(e2)*sin(e3) + cos(e1)*cos(e3)*sin(e2)) - cos(e4)*cos(e5)*(cos(e1)*cos(e2)*cos(e3) - cos(e1)*sin(e2)*sin(e3))) - cos(e6)*sin(e4)*(cos(e1)*cos(e2)*cos(e3) - cos(e1)*sin(e2)*sin(e3))) + y6*(cos(e6)*(sin(e5)*(cos(e1)*cos(e2)*sin(e3) + cos(e1)*cos(e3)*sin(e2)) - cos(e4)*cos(e5)*(cos(e1)*cos(e2)*cos(e3) - cos(e1)*sin(e2)*sin(e3))) + sin(e4)*sin(e6)*(cos(e1)*cos(e2)*cos(e3) - cos(e1)*sin(e2)*sin(e3))))*((sin(e6)*(sin(e5)*(cos(e1)*cos(e2)*cos(e3) - cos(e1)*sin(e2)*sin(e3)) + cos(e5)*(sin(e1)*sin(e4) + cos(e4)*(cos(e1)*cos(e2)*sin(e3) + cos(e1)*cos(e3)*sin(e2)))) - cos(e6)*(cos(e4)*sin(e1) - sin(e4)*(cos(e1)*cos(e2)*sin(e3) + cos(e1)*cos(e3)*sin(e2))))*(x6*(sin(e2 + e3)*cos(e5) + cos(e2 + e3)*cos(e4)*sin(e5)) - z6*(cos(e6)*(sin(e2 + e3)*sin(e5) - cos(e2 + e3)*cos(e4)*cos(e5)) + cos(e2 + e3)*sin(e4)*sin(e6)) + cos(e4)*cos(e6)*(a1 + d4*cos(e2 + e3) + a3*sin(e2 + e3) + a2*sin(e2)) - cos(e5)*sin(e4)*sin(e6)*(a1 + d4*cos(e2 + e3) + a3*sin(e2 + e3) + a2*sin(e2))) + (cos(e6)*(sin(e5)*(cos(e1)*cos(e2)*cos(e3) - cos(e1)*sin(e2)*sin(e3)) + cos(e5)*(sin(e1)*sin(e4) + cos(e4)*(cos(e1)*cos(e2)*sin(e3) + cos(e1)*cos(e3)*sin(e2)))) + sin(e6)*(cos(e4)*sin(e1) - sin(e4)*(cos(e1)*cos(e2)*sin(e3) + cos(e1)*cos(e3)*sin(e2))))*(y6*(sin(e2 + e3)*cos(e5) + cos(e2 + e3)*cos(e4)*sin(e5)) + z6*(sin(e6)*(sin(e2 + e3)*sin(e5) - cos(e2 + e3)*cos(e4)*cos(e5)) - cos(e2 + e3)*cos(e6)*sin(e4)) - cos(e4)*sin(e6)*(a1 + d4*cos(e2 + e3) + a3*sin(e2 + e3) + a2*sin(e2)) - cos(e5)*cos(e6)*sin(e4)*(a1 + d4*cos(e2 + e3) + a3*sin(e2 + e3) + a2*sin(e2))) - (cos(e5)*(cos(e1)*cos(e2)*cos(e3) - cos(e1)*sin(e2)*sin(e3)) - sin(e5)*(sin(e1)*sin(e4) + cos(e4)*(cos(e1)*cos(e2)*sin(e3) + cos(e1)*cos(e3)*sin(e2))))*(x6*(sin(e6)*(sin(e2 + e3)*sin(e5) - cos(e2 + e3)*cos(e4)*cos(e5)) - cos(e2 + e3)*cos(e6)*sin(e4)) + y6*(cos(e6)*(sin(e2 + e3)*sin(e5) - cos(e2 + e3)*cos(e4)*cos(e5)) + cos(e2 + e3)*sin(e4)*sin(e6)) - sin(e4)*sin(e5)*(a1 + d4*cos(e2 + e3) + a3*sin(e2 + e3) + a2*sin(e2)))) + m6*(x6*(sin(e6)*(sin(e5)*(cos(e2)*sin(e3) + cos(e3)*sin(e2)) + cos(e4)*cos(e5)*(sin(e2)*sin(e3) - cos(e2)*cos(e3))) + cos(e6)*sin(e4)*(sin(e2)*sin(e3) - cos(e2)*cos(e3))) + y6*(cos(e6)*(sin(e5)*(cos(e2)*sin(e3) + cos(e3)*sin(e2)) + cos(e4)*cos(e5)*(sin(e2)*sin(e3) - cos(e2)*cos(e3))) - sin(e4)*sin(e6)*(sin(e2)*sin(e3) - cos(e2)*cos(e3))))*((sin(e6)*(sin(e5)*(sin(e2)*sin(e3) - cos(e2)*cos(e3)) - cos(e4)*cos(e5)*(cos(e2)*sin(e3) + cos(e3)*sin(e2))) - cos(e6)*sin(e4)*(cos(e2)*sin(e3) + cos(e3)*sin(e2)))*(x6*(sin(e2 + e3)*cos(e5) + cos(e2 + e3)*cos(e4)*sin(e5)) - z6*(cos(e6)*(sin(e2 + e3)*sin(e5) - cos(e2 + e3)*cos(e4)*cos(e5)) + cos(e2 + e3)*sin(e4)*sin(e6)) + cos(e4)*cos(e6)*(a1 + d4*cos(e2 + e3) + a3*sin(e2 + e3) + a2*sin(e2)) - cos(e5)*sin(e4)*sin(e6)*(a1 + d4*cos(e2 + e3) + a3*sin(e2 + e3) + a2*sin(e2))) + (cos(e6)*(sin(e5)*(sin(e2)*sin(e3) - cos(e2)*cos(e3)) - cos(e4)*cos(e5)*(cos(e2)*sin(e3) + cos(e3)*sin(e2))) + sin(e4)*sin(e6)*(cos(e2)*sin(e3) + cos(e3)*sin(e2)))*(y6*(sin(e2 + e3)*cos(e5) + cos(e2 + e3)*cos(e4)*sin(e5)) + z6*(sin(e6)*(sin(e2 + e3)*sin(e5) - cos(e2 + e3)*cos(e4)*cos(e5)) - cos(e2 + e3)*cos(e6)*sin(e4)) - cos(e4)*sin(e6)*(a1 + d4*cos(e2 + e3) + a3*sin(e2 + e3) + a2*sin(e2)) - cos(e5)*cos(e6)*sin(e4)*(a1 + d4*cos(e2 + e3) + a3*sin(e2 + e3) + a2*sin(e2))) - (sin(e6)*(sin(e5)*(cos(e2)*sin(e3) + cos(e3)*sin(e2)) + cos(e4)*cos(e5)*(sin(e2)*sin(e3) - cos(e2)*cos(e3))) + cos(e6)*sin(e4)*(sin(e2)*sin(e3) - cos(e2)*cos(e3)))*(x6*(cos(e2 + e3)*cos(e5) - sin(e2 + e3)*cos(e4)*sin(e5)) - z6*(cos(e6)*(cos(e2 + e3)*sin(e5) + sin(e2 + e3)*cos(e4)*cos(e5)) - sin(e2 + e3)*sin(e4)*sin(e6)) + cos(e4)*cos(e6)*(a3*cos(e2 + e3) - d4*sin(e2 + e3)) - cos(e5)*sin(e4)*sin(e6)*(a3*cos(e2 + e3) - d4*sin(e2 + e3))) - (cos(e6)*(sin(e5)*(cos(e2)*sin(e3) + cos(e3)*sin(e2)) + cos(e4)*cos(e5)*(sin(e2)*sin(e3) - cos(e2)*cos(e3))) - sin(e4)*sin(e6)*(sin(e2)*sin(e3) - cos(e2)*cos(e3)))*(y6*(cos(e2 + e3)*cos(e5) - sin(e2 + e3)*cos(e4)*sin(e5)) + z6*(sin(e6)*(cos(e2 + e3)*sin(e5) + sin(e2 + e3)*cos(e4)*cos(e5)) + sin(e2 + e3)*cos(e6)*sin(e4)) - cos(e4)*sin(e6)*(a3*cos(e2 + e3) - d4*sin(e2 + e3)) - cos(e5)*cos(e6)*sin(e4)*(a3*cos(e2 + e3) - d4*sin(e2 + e3))) - (cos(e5)*(sin(e2)*sin(e3) - cos(e2)*cos(e3)) + cos(e4)*sin(e5)*(cos(e2)*sin(e3) + cos(e3)*sin(e2)))*(x6*(sin(e6)*(sin(e2 + e3)*sin(e5) - cos(e2 + e3)*cos(e4)*cos(e5)) - cos(e2 + e3)*cos(e6)*sin(e4)) + y6*(cos(e6)*(sin(e2 + e3)*sin(e5) - cos(e2 + e3)*cos(e4)*cos(e5)) + cos(e2 + e3)*sin(e4)*sin(e6)) - sin(e4)*sin(e5)*(a1 + d4*cos(e2 + e3) + a3*sin(e2 + e3) + a2*sin(e2))) + (cos(e5)*(cos(e2)*sin(e3) + cos(e3)*sin(e2)) - cos(e4)*sin(e5)*(sin(e2)*sin(e3) - cos(e2)*cos(e3)))*(x6*(sin(e6)*(cos(e2 + e3)*sin(e5) + sin(e2 + e3)*cos(e4)*cos(e5)) + sin(e2 + e3)*cos(e6)*sin(e4)) + y6*(cos(e6)*(cos(e2 + e3)*sin(e5) + sin(e2 + e3)*cos(e4)*cos(e5)) - sin(e2 + e3)*sin(e4)*sin(e6)) - sin(e4)*sin(e5)*(a3*cos(e2 + e3) - d4*sin(e2 + e3)))) + m6*(x6*(sin(e6)*(sin(e5)*(sin(e2)*sin(e3) - cos(e2)*cos(e3)) - cos(e4)*cos(e5)*(cos(e2)*sin(e3) + cos(e3)*sin(e2))) - cos(e6)*sin(e4)*(cos(e2)*sin(e3) + cos(e3)*sin(e2))) + y6*(cos(e6)*(sin(e5)*(sin(e2)*sin(e3) - cos(e2)*cos(e3)) - cos(e4)*cos(e5)*(cos(e2)*sin(e3) + cos(e3)*sin(e2))) + sin(e4)*sin(e6)*(cos(e2)*sin(e3) + cos(e3)*sin(e2))))*((sin(e6)*(sin(e5)*(cos(e2)*sin(e3) + cos(e3)*sin(e2)) + cos(e4)*cos(e5)*(sin(e2)*sin(e3) - cos(e2)*cos(e3))) + cos(e6)*sin(e4)*(sin(e2)*sin(e3) - cos(e2)*cos(e3)))*(x6*(sin(e2 + e3)*cos(e5) + cos(e2 + e3)*cos(e4)*sin(e5)) - z6*(cos(e6)*(sin(e2 + e3)*sin(e5) - cos(e2 + e3)*cos(e4)*cos(e5)) + cos(e2 + e3)*sin(e4)*sin(e6)) + cos(e4)*cos(e6)*(a1 + d4*cos(e2 + e3) + a3*sin(e2 + e3) + a2*sin(e2)) - cos(e5)*sin(e4)*sin(e6)*(a1 + d4*cos(e2 + e3) + a3*sin(e2 + e3) + a2*sin(e2))) + (cos(e6)*(sin(e5)*(cos(e2)*sin(e3) + cos(e3)*sin(e2)) + cos(e4)*cos(e5)*(sin(e2)*sin(e3) - cos(e2)*cos(e3))) - sin(e4)*sin(e6)*(sin(e2)*sin(e3) - cos(e2)*cos(e3)))*(y6*(sin(e2 + e3)*cos(e5) + cos(e2 + e3)*cos(e4)*sin(e5)) + z6*(sin(e6)*(sin(e2 + e3)*sin(e5) - cos(e2 + e3)*cos(e4)*cos(e5)) - cos(e2 + e3)*cos(e6)*sin(e4)) - cos(e4)*sin(e6)*(a1 + d4*cos(e2 + e3) + a3*sin(e2 + e3) + a2*sin(e2)) - cos(e5)*cos(e6)*sin(e4)*(a1 + d4*cos(e2 + e3) + a3*sin(e2 + e3) + a2*sin(e2))) - (cos(e5)*(cos(e2)*sin(e3) + cos(e3)*sin(e2)) - cos(e4)*sin(e5)*(sin(e2)*sin(e3) - cos(e2)*cos(e3)))*(x6*(sin(e6)*(sin(e2 + e3)*sin(e5) - cos(e2 + e3)*cos(e4)*cos(e5)) - cos(e2 + e3)*cos(e6)*sin(e4)) + y6*(cos(e6)*(sin(e2 + e3)*sin(e5) - cos(e2 + e3)*cos(e4)*cos(e5)) + cos(e2 + e3)*sin(e4)*sin(e6)) - sin(e4)*sin(e5)*(a1 + d4*cos(e2 + e3) + a3*sin(e2 + e3) + a2*sin(e2)))) + m6*(x6*(sin(e6)*(sin(e5)*(cos(e2)*sin(e1)*sin(e3) + cos(e3)*sin(e1)*sin(e2)) - cos(e4)*cos(e5)*(cos(e2)*cos(e3)*sin(e1) - sin(e1)*sin(e2)*sin(e3))) - cos(e6)*sin(e4)*(cos(e2)*cos(e3)*sin(e1) - sin(e1)*sin(e2)*sin(e3))) + y6*(cos(e6)*(sin(e5)*(cos(e2)*sin(e1)*sin(e3) + cos(e3)*sin(e1)*sin(e2)) - cos(e4)*cos(e5)*(cos(e2)*cos(e3)*sin(e1) - sin(e1)*sin(e2)*sin(e3))) + sin(e4)*sin(e6)*(cos(e2)*cos(e3)*sin(e1) - sin(e1)*sin(e2)*sin(e3))))*((sin(e6)*(sin(e5)*(cos(e2)*cos(e3)*sin(e1) - sin(e1)*sin(e2)*sin(e3)) - cos(e5)*(cos(e1)*sin(e4) - cos(e4)*(cos(e2)*sin(e1)*sin(e3) + cos(e3)*sin(e1)*sin(e2)))) + cos(e6)*(sin(e4)*(cos(e2)*sin(e1)*sin(e3) + cos(e3)*sin(e1)*sin(e2)) + cos(e1)*cos(e4)))*(x6*(sin(e2 + e3)*cos(e5) + cos(e2 + e3)*cos(e4)*sin(e5)) - z6*(cos(e6)*(sin(e2 + e3)*sin(e5) - cos(e2 + e3)*cos(e4)*cos(e5)) + cos(e2 + e3)*sin(e4)*sin(e6)) + cos(e4)*cos(e6)*(a1 + d4*cos(e2 + e3) + a3*sin(e2 + e3) + a2*sin(e2)) - cos(e5)*sin(e4)*sin(e6)*(a1 + d4*cos(e2 + e3) + a3*sin(e2 + e3) + a2*sin(e2))) + (cos(e6)*(sin(e5)*(cos(e2)*cos(e3)*sin(e1) - sin(e1)*sin(e2)*sin(e3)) - cos(e5)*(cos(e1)*sin(e4) - cos(e4)*(cos(e2)*sin(e1)*sin(e3) + cos(e3)*sin(e1)*sin(e2)))) - sin(e6)*(sin(e4)*(cos(e2)*sin(e1)*sin(e3) + cos(e3)*sin(e1)*sin(e2)) + cos(e1)*cos(e4)))*(y6*(sin(e2 + e3)*cos(e5) + cos(e2 + e3)*cos(e4)*sin(e5)) + z6*(sin(e6)*(sin(e2 + e3)*sin(e5) - cos(e2 + e3)*cos(e4)*cos(e5)) - cos(e2 + e3)*cos(e6)*sin(e4)) - cos(e4)*sin(e6)*(a1 + d4*cos(e2 + e3) + a3*sin(e2 + e3) + a2*sin(e2)) - cos(e5)*cos(e6)*sin(e4)*(a1 + d4*cos(e2 + e3) + a3*sin(e2 + e3) + a2*sin(e2))) - (cos(e5)*(cos(e2)*cos(e3)*sin(e1) - sin(e1)*sin(e2)*sin(e3)) + sin(e5)*(cos(e1)*sin(e4) - cos(e4)*(cos(e2)*sin(e1)*sin(e3) + cos(e3)*sin(e1)*sin(e2))))*(x6*(sin(e6)*(sin(e2 + e3)*sin(e5) - cos(e2 + e3)*cos(e4)*cos(e5)) - cos(e2 + e3)*cos(e6)*sin(e4)) + y6*(cos(e6)*(sin(e2 + e3)*sin(e5) - cos(e2 + e3)*cos(e4)*cos(e5)) + cos(e2 + e3)*sin(e4)*sin(e6)) - sin(e4)*sin(e5)*(a1 + d4*cos(e2 + e3) + a3*sin(e2 + e3) + a2*sin(e2)))) - m6*(x6*(sin(e6)*(sin(e5)*(cos(e1)*cos(e2)*cos(e3) - cos(e1)*sin(e2)*sin(e3)) + cos(e5)*(sin(e1)*sin(e4) + cos(e4)*(cos(e1)*cos(e2)*sin(e3) + cos(e1)*cos(e3)*sin(e2)))) - cos(e6)*(cos(e4)*sin(e1) - sin(e4)*(cos(e1)*cos(e2)*sin(e3) + cos(e1)*cos(e3)*sin(e2)))) + y6*(cos(e6)*(sin(e5)*(cos(e1)*cos(e2)*cos(e3) - cos(e1)*sin(e2)*sin(e3)) + cos(e5)*(sin(e1)*sin(e4) + cos(e4)*(cos(e1)*cos(e2)*sin(e3) + cos(e1)*cos(e3)*sin(e2)))) + sin(e6)*(cos(e4)*sin(e1) - sin(e4)*(cos(e1)*cos(e2)*sin(e3) + cos(e1)*cos(e3)*sin(e2)))))*((sin(e6)*(sin(e5)*(cos(e1)*cos(e2)*cos(e3) - cos(e1)*sin(e2)*sin(e3)) + cos(e5)*(sin(e1)*sin(e4) + cos(e4)*(cos(e1)*cos(e2)*sin(e3) + cos(e1)*cos(e3)*sin(e2)))) - cos(e6)*(cos(e4)*sin(e1) - sin(e4)*(cos(e1)*cos(e2)*sin(e3) + cos(e1)*cos(e3)*sin(e2))))*(x6*(cos(e2 + e3)*cos(e5) - sin(e2 + e3)*cos(e4)*sin(e5)) - z6*(cos(e6)*(cos(e2 + e3)*sin(e5) + sin(e2 + e3)*cos(e4)*cos(e5)) - sin(e2 + e3)*sin(e4)*sin(e6)) + cos(e4)*cos(e6)*(a3*cos(e2 + e3) - d4*sin(e2 + e3)) - cos(e5)*sin(e4)*sin(e6)*(a3*cos(e2 + e3) - d4*sin(e2 + e3))) + (cos(e6)*(sin(e5)*(cos(e1)*cos(e2)*cos(e3) - cos(e1)*sin(e2)*sin(e3)) + cos(e5)*(sin(e1)*sin(e4) + cos(e4)*(cos(e1)*cos(e2)*sin(e3) + cos(e1)*cos(e3)*sin(e2)))) + sin(e6)*(cos(e4)*sin(e1) - sin(e4)*(cos(e1)*cos(e2)*sin(e3) + cos(e1)*cos(e3)*sin(e2))))*(y6*(cos(e2 + e3)*cos(e5) - sin(e2 + e3)*cos(e4)*sin(e5)) + z6*(sin(e6)*(cos(e2 + e3)*sin(e5) + sin(e2 + e3)*cos(e4)*cos(e5)) + sin(e2 + e3)*cos(e6)*sin(e4)) - cos(e4)*sin(e6)*(a3*cos(e2 + e3) - d4*sin(e2 + e3)) - cos(e5)*cos(e6)*sin(e4)*(a3*cos(e2 + e3) - d4*sin(e2 + e3))) - (cos(e5)*(cos(e1)*cos(e2)*cos(e3) - cos(e1)*sin(e2)*sin(e3)) - sin(e5)*(sin(e1)*sin(e4) + cos(e4)*(cos(e1)*cos(e2)*sin(e3) + cos(e1)*cos(e3)*sin(e2))))*(x6*(sin(e6)*(cos(e2 + e3)*sin(e5) + sin(e2 + e3)*cos(e4)*cos(e5)) + sin(e2 + e3)*cos(e6)*sin(e4)) + y6*(cos(e6)*(cos(e2 + e3)*sin(e5) + sin(e2 + e3)*cos(e4)*cos(e5)) - sin(e2 + e3)*sin(e4)*sin(e6)) - sin(e4)*sin(e5)*(a3*cos(e2 + e3) - d4*sin(e2 + e3))) + (cos(e5)*(cos(e1)*cos(e2)*sin(e3) + cos(e1)*cos(e3)*sin(e2)) + cos(e4)*sin(e5)*(cos(e1)*cos(e2)*cos(e3) - cos(e1)*sin(e2)*sin(e3)))*(x6*(sin(e6)*(sin(e2 + e3)*sin(e5) - cos(e2 + e3)*cos(e4)*cos(e5)) - cos(e2 + e3)*cos(e6)*sin(e4)) + y6*(cos(e6)*(sin(e2 + e3)*sin(e5) - cos(e2 + e3)*cos(e4)*cos(e5)) + cos(e2 + e3)*sin(e4)*sin(e6)) - sin(e4)*sin(e5)*(a1 + d4*cos(e2 + e3) + a3*sin(e2 + e3) + a2*sin(e2))) - (sin(e6)*(sin(e5)*(cos(e1)*cos(e2)*sin(e3) + cos(e1)*cos(e3)*sin(e2)) - cos(e4)*cos(e5)*(cos(e1)*cos(e2)*cos(e3) - cos(e1)*sin(e2)*sin(e3))) - cos(e6)*sin(e4)*(cos(e1)*cos(e2)*cos(e3) - cos(e1)*sin(e2)*sin(e3)))*(x6*(sin(e2 + e3)*cos(e5) + cos(e2 + e3)*cos(e4)*sin(e5)) - z6*(cos(e6)*(sin(e2 + e3)*sin(e5) - cos(e2 + e3)*cos(e4)*cos(e5)) + cos(e2 + e3)*sin(e4)*sin(e6)) + cos(e4)*cos(e6)*(a1 + d4*cos(e2 + e3) + a3*sin(e2 + e3) + a2*sin(e2)) - cos(e5)*sin(e4)*sin(e6)*(a1 + d4*cos(e2 + e3) + a3*sin(e2 + e3) + a2*sin(e2))) - (cos(e6)*(sin(e5)*(cos(e1)*cos(e2)*sin(e3) + cos(e1)*cos(e3)*sin(e2)) - cos(e4)*cos(e5)*(cos(e1)*cos(e2)*cos(e3) - cos(e1)*sin(e2)*sin(e3))) + sin(e4)*sin(e6)*(cos(e1)*cos(e2)*cos(e3) - cos(e1)*sin(e2)*sin(e3)))*(y6*(sin(e2 + e3)*cos(e5) + cos(e2 + e3)*cos(e4)*sin(e5)) + z6*(sin(e6)*(sin(e2 + e3)*sin(e5) - cos(e2 + e3)*cos(e4)*cos(e5)) - cos(e2 + e3)*cos(e6)*sin(e4)) - cos(e4)*sin(e6)*(a1 + d4*cos(e2 + e3) + a3*sin(e2 + e3) + a2*sin(e2)) - cos(e5)*cos(e6)*sin(e4)*(a1 + d4*cos(e2 + e3) + a3*sin(e2 + e3) + a2*sin(e2)))) + m6*(x6*(sin(e6)*(sin(e5)*(cos(e2)*cos(e3)*sin(e1) - sin(e1)*sin(e2)*sin(e3)) - cos(e5)*(cos(e1)*sin(e4) - cos(e4)*(cos(e2)*sin(e1)*sin(e3) + cos(e3)*sin(e1)*sin(e2)))) + cos(e6)*(sin(e4)*(cos(e2)*sin(e1)*sin(e3) + cos(e3)*sin(e1)*sin(e2)) + cos(e1)*cos(e4))) + y6*(cos(e6)*(sin(e5)*(cos(e2)*cos(e3)*sin(e1) - sin(e1)*sin(e2)*sin(e3)) - cos(e5)*(cos(e1)*sin(e4) - cos(e4)*(cos(e2)*sin(e1)*sin(e3) + cos(e3)*sin(e1)*sin(e2)))) - sin(e6)*(sin(e4)*(cos(e2)*sin(e1)*sin(e3) + cos(e3)*sin(e1)*sin(e2)) + cos(e1)*cos(e4))))*((sin(e6)*(sin(e5)*(cos(e2)*sin(e1)*sin(e3) + cos(e3)*sin(e1)*sin(e2)) - cos(e4)*cos(e5)*(cos(e2)*cos(e3)*sin(e1) - sin(e1)*sin(e2)*sin(e3))) - cos(e6)*sin(e4)*(cos(e2)*cos(e3)*sin(e1) - sin(e1)*sin(e2)*sin(e3)))*(x6*(sin(e2 + e3)*cos(e5) + cos(e2 + e3)*cos(e4)*sin(e5)) - z6*(cos(e6)*(sin(e2 + e3)*sin(e5) - cos(e2 + e3)*cos(e4)*cos(e5)) + cos(e2 + e3)*sin(e4)*sin(e6)) + cos(e4)*cos(e6)*(a1 + d4*cos(e2 + e3) + a3*sin(e2 + e3) + a2*sin(e2)) - cos(e5)*sin(e4)*sin(e6)*(a1 + d4*cos(e2 + e3) + a3*sin(e2 + e3) + a2*sin(e2))) + (cos(e6)*(sin(e5)*(cos(e2)*sin(e1)*sin(e3) + cos(e3)*sin(e1)*sin(e2)) - cos(e4)*cos(e5)*(cos(e2)*cos(e3)*sin(e1) - sin(e1)*sin(e2)*sin(e3))) + sin(e4)*sin(e6)*(cos(e2)*cos(e3)*sin(e1) - sin(e1)*sin(e2)*sin(e3)))*(y6*(sin(e2 + e3)*cos(e5) + cos(e2 + e3)*cos(e4)*sin(e5)) + z6*(sin(e6)*(sin(e2 + e3)*sin(e5) - cos(e2 + e3)*cos(e4)*cos(e5)) - cos(e2 + e3)*cos(e6)*sin(e4)) - cos(e4)*sin(e6)*(a1 + d4*cos(e2 + e3) + a3*sin(e2 + e3) + a2*sin(e2)) - cos(e5)*cos(e6)*sin(e4)*(a1 + d4*cos(e2 + e3) + a3*sin(e2 + e3) + a2*sin(e2))) - (sin(e6)*(sin(e5)*(cos(e2)*cos(e3)*sin(e1) - sin(e1)*sin(e2)*sin(e3)) - cos(e5)*(cos(e1)*sin(e4) - cos(e4)*(cos(e2)*sin(e1)*sin(e3) + cos(e3)*sin(e1)*sin(e2)))) + cos(e6)*(sin(e4)*(cos(e2)*sin(e1)*sin(e3) + cos(e3)*sin(e1)*sin(e2)) + cos(e1)*cos(e4)))*(x6*(cos(e2 + e3)*cos(e5) - sin(e2 + e3)*cos(e4)*sin(e5)) - z6*(cos(e6)*(cos(e2 + e3)*sin(e5) + sin(e2 + e3)*cos(e4)*cos(e5)) - sin(e2 + e3)*sin(e4)*sin(e6)) + cos(e4)*cos(e6)*(a3*cos(e2 + e3) - d4*sin(e2 + e3)) - cos(e5)*sin(e4)*sin(e6)*(a3*cos(e2 + e3) - d4*sin(e2 + e3))) - (cos(e6)*(sin(e5)*(cos(e2)*cos(e3)*sin(e1) - sin(e1)*sin(e2)*sin(e3)) - cos(e5)*(cos(e1)*sin(e4) - cos(e4)*(cos(e2)*sin(e1)*sin(e3) + cos(e3)*sin(e1)*sin(e2)))) - sin(e6)*(sin(e4)*(cos(e2)*sin(e1)*sin(e3) + cos(e3)*sin(e1)*sin(e2)) + cos(e1)*cos(e4)))*(y6*(cos(e2 + e3)*cos(e5) - sin(e2 + e3)*cos(e4)*sin(e5)) + z6*(sin(e6)*(cos(e2 + e3)*sin(e5) + sin(e2 + e3)*cos(e4)*cos(e5)) + sin(e2 + e3)*cos(e6)*sin(e4)) - cos(e4)*sin(e6)*(a3*cos(e2 + e3) - d4*sin(e2 + e3)) - cos(e5)*cos(e6)*sin(e4)*(a3*cos(e2 + e3) - d4*sin(e2 + e3))) + (cos(e5)*(cos(e2)*cos(e3)*sin(e1) - sin(e1)*sin(e2)*sin(e3)) + sin(e5)*(cos(e1)*sin(e4) - cos(e4)*(cos(e2)*sin(e1)*sin(e3) + cos(e3)*sin(e1)*sin(e2))))*(x6*(sin(e6)*(cos(e2 + e3)*sin(e5) + sin(e2 + e3)*cos(e4)*cos(e5)) + sin(e2 + e3)*cos(e6)*sin(e4)) + y6*(cos(e6)*(cos(e2 + e3)*sin(e5) + sin(e2 + e3)*cos(e4)*cos(e5)) - sin(e2 + e3)*sin(e4)*sin(e6)) - sin(e4)*sin(e5)*(a3*cos(e2 + e3) - d4*sin(e2 + e3))) - (cos(e5)*(cos(e2)*sin(e1)*sin(e3) + cos(e3)*sin(e1)*sin(e2)) + cos(e4)*sin(e5)*(cos(e2)*cos(e3)*sin(e1) - sin(e1)*sin(e2)*sin(e3)))*(x6*(sin(e6)*(sin(e2 + e3)*sin(e5) - cos(e2 + e3)*cos(e4)*cos(e5)) - cos(e2 + e3)*cos(e6)*sin(e4)) + y6*(cos(e6)*(sin(e2 + e3)*sin(e5) - cos(e2 + e3)*cos(e4)*cos(e5)) + cos(e2 + e3)*sin(e4)*sin(e6)) - sin(e4)*sin(e5)*(a1 + d4*cos(e2 + e3) + a3*sin(e2 + e3) + a2*sin(e2))))) + de2*((I6yz*(sin(e6)*(cos(e2 + e3)*sin(e5) + sin(e2 + e3)*cos(e4)*cos(e5)) + sin(e2 + e3)*cos(e6)*sin(e4)))/2 - (I6xz*(cos(e6)*(cos(e2 + e3)*sin(e5) + sin(e2 + e3)*cos(e4)*cos(e5)) - sin(e2 + e3)*sin(e4)*sin(e6)))/2 - I6zz*(cos(e2 + e3)*cos(e5) - sin(e2 + e3)*cos(e4)*sin(e5)) - (I6zx*(cos(e6)*(cos(e2 + e3)*sin(e5) + sin(e2 + e3)*cos(e4)*cos(e5)) - sin(e2 + e3)*sin(e4)*sin(e6)))/2 + (I6zy*(sin(e6)*(cos(e2 + 